simulink model "model"  (R2014a)
(part 1 of 6)
settings: Solver=VariableStepAuto  StartTime=0.0  StopTime=10.0  RelTol=1e-3
libraries: powerlib x1872
settings Model: Creator=lej  LastModifiedBy=leimhofe
settings DataIOCC: SaveFormat=Dataset
settings OptimizationCC: SimCompilerOptimization=off
settings DebuggingCC: MergeDetectMultiDrivingBlocksExec=error  SolverPrmCheckMsg=none  FrameProcessingCompatibilityMsg=error  AllowSymbolicDim=off
settings HardwareCC: ProdBitPerPointer=64  ProdLargestAtomicFloat=Float  ProdIntDivRoundTo=Zero  ProdEndianess=LittleEndian  ProdWordSize=64  ProdHWDeviceType=Intel->x86-64 (Windows64)
settings RTWCC: RTWCompilerOptimization=off
settings GRTTargetCC: GeneratePreprocessorConditionals=Use local settings
settings ConfigComp: CovMetricSettings=dw  CovHtmlReporting=on  CovSaveCumulativeToWorkspaceVar=on  CovSaveSingleToWorkspaceVar=on  CovExternalEMLEnable=off

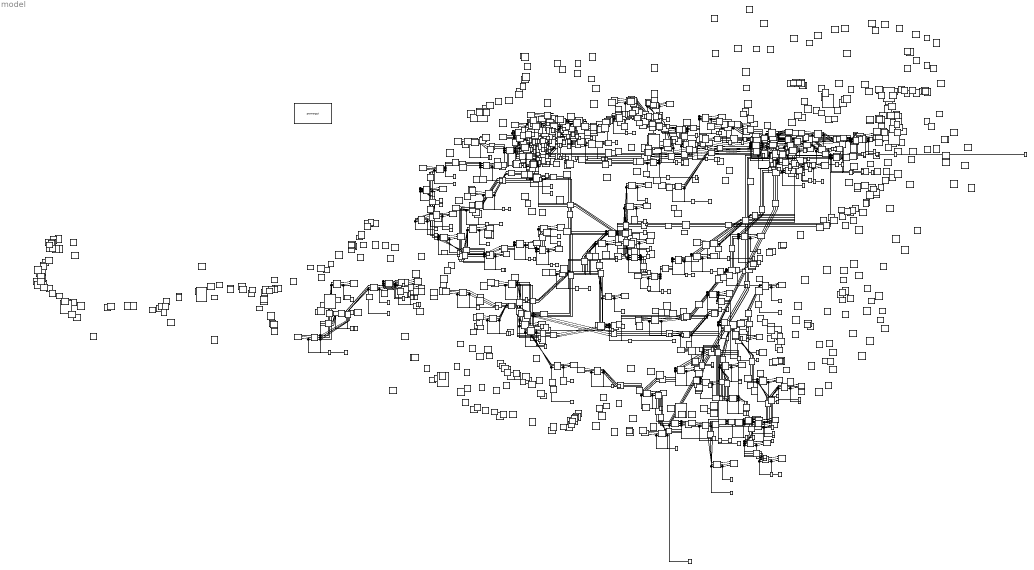
== system model ==
  note: 110000 Volts Power Line
  note: 330000 Volts Power Line
  Aigerding___Antiesenhofen_CN_95975628_110000_CN_95972388_110000 : powerlib/Elements/Distributed Parameters Line  Phases=3  Frequency=60  Resistance=[0.01273 0.3864]  Inductance="[0.9337e-3  4.1264e-3]"  Capacitance=[12.74e-9 7.751e-9]  Length=100  x1=[0 0 0 0; 0.0001244 0 0 0; 0.0002488 0 0 0; 0.0003733 0 0 0; 0.0004977 0 0 0; 0.0006221 0 0 0]  x2=[0 0 0 0; 0.0001244 0 0 0; 0.0002488 0 0 0; 0.0003733 0 0 0; 0.0004977 0 0 0; 0.0006221 0 0 0]  x3=[0 0 0 0; 0.0001244 0 0 0; 0.0002488 0 0 0; 0.0003733 0 0 0; 0.0004977 0 0 0; 0.0006221 0 0 0]  x4=[0 0 0 0; 0.0001244 0 0 0; 0.0002488 0 0 0; 0.0003733 0 0 0; 0.0004977 0 0 0; 0.0006221 0 0 0]  x5=0  V1=ones(3,3)  V2=ones(3,3)  I1=ones(3,3)  I2=ones(3,3)  nHarmo=1  Measurements=None
  Aigerding___Antiesenhofen_CN_95975628_110000_CN_95978048_110000 : powerlib/Elements/Distributed Parameters Line  Phases=3  Frequency=60  Resistance=[0.01273 0.3864]  Inductance="[0.9337e-3  4.1264e-3]"  Capacitance=[12.74e-9 7.751e-9]  Length=100  x1=[0 0 0 0; 0.0001244 0 0 0; 0.0002488 0 0 0; 0.0003733 0 0 0; 0.0004977 0 0 0; 0.0006221 0 0 0]  x2=[0 0 0 0; 0.0001244 0 0 0; 0.0002488 0 0 0; 0.0003733 0 0 0; 0.0004977 0 0 0; 0.0006221 0 0 0]  x3=[0 0 0 0; 0.0001244 0 0 0; 0.0002488 0 0 0; 0.0003733 0 0 0; 0.0004977 0 0 0; 0.0006221 0 0 0]  x4=[0 0 0 0; 0.0001244 0 0 0; 0.0002488 0 0 0; 0.0003733 0 0 0; 0.0004977 0 0 0; 0.0006221 0 0 0]  x5=0  V1=ones(3,3)  V2=ones(3,3)  I1=ones(3,3)  I2=ones(3,3)  nHarmo=1  Measurements=None
  Alutaguse_—_Estonia_Põhja_110_kV_CN_35367472_110000_CN_35594689_110000 : powerlib/Elements/Distributed Parameters Line  Phases=3  Frequency=60  Resistance=[0.01273 0.3864]  Inductance="[0.9337e-3  4.1264e-3]"  Capacitance=[12.74e-9 7.751e-9]  Length=6.3466  x1=[0 0 0 0; 0.0001244 0 0 0; 0.0002488 0 0 0; 0.0003733 0 0 0; 0.0004977 0 0 0; 0.0006221 0 0 0]  x2=[0 0 0 0; 0.0001244 0 0 0; 0.0002488 0 0 0; 0.0003733 0 0 0; 0.0004977 0 0 0; 0.0006221 0 0 0]  x3=[0 0 0 0; 0.0001244 0 0 0; 0.0002488 0 0 0; 0.0003733 0 0 0; 0.0004977 0 0 0; 0.0006221 0 0 0]  x4=[0 0 0 0; 0.0001244 0 0 0; 0.0002488 0 0 0; 0.0003733 0 0 0; 0.0004977 0 0 0; 0.0006221 0 0 0]  x5=0  V1=ones(3,3)  V2=ones(3,3)  I1=ones(3,3)  I2=ones(3,3)  nHarmo=1  Measurements=None
  Alutaguse_—_Konsu_110_kV_CN_35367472_110000_CN_34903294_110000 : powerlib/Elements/Distributed Parameters Line  Phases=3  Frequency=60  Resistance=[0.01273 0.3864]  Inductance="[0.9337e-3  4.1264e-3]"  Capacitance=[12.74e-9 7.751e-9]  Length=14.9855  x1=[0 0 0 0; 0.0001244 0 0 0; 0.0002488 0 0 0; 0.0003733 0 0 0; 0.0004977 0 0 0; 0.0006221 0 0 0]  x2=[0 0 0 0; 0.0001244 0 0 0; 0.0002488 0 0 0; 0.0003733 0 0 0; 0.0004977 0 0 0; 0.0006221 0 0 0]  x3=[0 0 0 0; 0.0001244 0 0 0; 0.0002488 0 0 0; 0.0003733 0 0 0; 0.0004977 0 0 0; 0.0006221 0 0 0]  x4=[0 0 0 0; 0.0001244 0 0 0; 0.0002488 0 0 0; 0.0003733 0 0 0; 0.0004977 0 0 0; 0.0006221 0 0 0]  x5=0  V1=ones(3,3)  V2=ones(3,3)  I1=ones(3,3)  I2=ones(3,3)  nHarmo=1  Measurements=None
  Andau___Frauenkirchen_CN_60222001_110000_CN_174474431_110000 : powerlib/Elements/Distributed Parameters Line  Phases=3  Frequency=60  Resistance=[0.01273 0.3864]  Inductance="[0.9337e-3  4.1264e-3]"  Capacitance=[12.74e-9 7.751e-9]  Length=100  x1=[0 0 0 0; 0.0001244 0 0 0; 0.0002488 0 0 0; 0.0003733 0 0 0; 0.0004977 0 0 0; 0.0006221 0 0 0]  x2=[0 0 0 0; 0.0001244 0 0 0; 0.0002488 0 0 0; 0.0003733 0 0 0; 0.0004977 0 0 0; 0.0006221 0 0 0]  x3=[0 0 0 0; 0.0001244 0 0 0; 0.0002488 0 0 0; 0.0003733 0 0 0; 0.0004977 0 0 0; 0.0006221 0 0 0]  x4=[0 0 0 0; 0.0001244 0 0 0; 0.0002488 0 0 0; 0.0003733 0 0 0; 0.0004977 0 0 0; 0.0006221 0 0 0]  x5=0  V1=ones(3,3)  V2=ones(3,3)  I1=ones(3,3)  I2=ones(3,3)  nHarmo=1  Measurements=None
  Anne_—_Kuuste_110_kV_CN_35445346_110000_CN_30228363_110000 : powerlib/Elements/Distributed Parameters Line  Phases=3  Frequency=60  Resistance=[0.01273 0.3864]  Inductance="[0.9337e-3  4.1264e-3]"  Capacitance=[12.74e-9 7.751e-9]  Length=10.9015  x1=[0 0 0 0; 0.0001244 0 0 0; 0.0002488 0 0 0; 0.0003733 0 0 0; 0.0004977 0 0 0; 0.0006221 0 0 0]  x2=[0 0 0 0; 0.0001244 0 0 0; 0.0002488 0 0 0; 0.0003733 0 0 0; 0.0004977 0 0 0; 0.0006221 0 0 0]  x3=[0 0 0 0; 0.0001244 0 0 0; 0.0002488 0 0 0; 0.0003733 0 0 0; 0.0004977 0 0 0; 0.0006221 0 0 0]  x4=[0 0 0 0; 0.0001244 0 0 0; 0.0002488 0 0 0; 0.0003733 0 0 0; 0.0004977 0 0 0; 0.0006221 0 0 0]  x5=0  V1=ones(3,3)  V2=ones(3,3)  I1=ones(3,3)  I2=ones(3,3)  nHarmo=1  Measurements=None
  Anne_—_Kuuste_110_kV_CN_35445346_110000_CN_35594688_110000 : powerlib/Elements/Distributed Parameters Line  Phases=3  Frequency=60  Resistance=[0.01273 0.3864]  Inductance="[0.9337e-3  4.1264e-3]"  Capacitance=[12.74e-9 7.751e-9]  Length=45.2985  x1=[0 0 0 0; 0.0001244 0 0 0; 0.0002488 0 0 0; 0.0003733 0 0 0; 0.0004977 0 0 0; 0.0006221 0 0 0]  x2=[0 0 0 0; 0.0001244 0 0 0; 0.0002488 0 0 0; 0.0003733 0 0 0; 0.0004977 0 0 0; 0.0006221 0 0 0]  x3=[0 0 0 0; 0.0001244 0 0 0; 0.0002488 0 0 0; 0.0003733 0 0 0; 0.0004977 0 0 0; 0.0006221 0 0 0]  x4=[0 0 0 0; 0.0001244 0 0 0; 0.0002488 0 0 0; 0.0003733 0 0 0; 0.0004977 0 0 0; 0.0006221 0 0 0]  x5=0  V1=ones(3,3)  V2=ones(3,3)  I1=ones(3,3)  I2=ones(3,3)  nHarmo=1  Measurements=None
  Aruküla_—_Jüri_110_kV_CN_34968285_110000_CN_204914596_110000 : powerlib/Elements/Distributed Parameters Line  Phases=3  Frequency=60  Resistance=[0.01273 0.3864]  Inductance="[0.9337e-3  4.1264e-3]"  Capacitance=[12.74e-9 7.751e-9]  Length=9.3434  x1=[0 0 0 0; 0.0001244 0 0 0; 0.0002488 0 0 0; 0.0003733 0 0 0; 0.0004977 0 0 0; 0.0006221 0 0 0]  x2=[0 0 0 0; 0.0001244 0 0 0; 0.0002488 0 0 0; 0.0003733 0 0 0; 0.0004977 0 0 0; 0.0006221 0 0 0]  x3=[0 0 0 0; 0.0001244 0 0 0; 0.0002488 0 0 0; 0.0003733 0 0 0; 0.0004977 0 0 0; 0.0006221 0 0 0]  x4=[0 0 0 0; 0.0001244 0 0 0; 0.0002488 0 0 0; 0.0003733 0 0 0; 0.0004977 0 0 0; 0.0006221 0 0 0]  x5=0  V1=ones(3,3)  V2=ones(3,3)  I1=ones(3,3)  I2=ones(3,3)  nHarmo=1  Measurements=None
  Aruküla_—_Kallavere_110_kV_CN_204914596_110000_CN_29979106_110000 : powerlib/Elements/Distributed Parameters Line  Phases=3  Frequency=60  Resistance=[0.01273 0.3864]  Inductance="[0.9337e-3  4.1264e-3]"  Capacitance=[12.74e-9 7.751e-9]  Length=24.2792  x1=[0 0 0 0; 0.0001244 0 0 0; 0.0002488 0 0 0; 0.0003733 0 0 0; 0.0004977 0 0 0; 0.0006221 0 0 0]  x2=[0 0 0 0; 0.0001244 0 0 0; 0.0002488 0 0 0; 0.0003733 0 0 0; 0.0004977 0 0 0; 0.0006221 0 0 0]  x3=[0 0 0 0; 0.0001244 0 0 0; 0.0002488 0 0 0; 0.0003733 0 0 0; 0.0004977 0 0 0; 0.0006221 0 0 0]  x4=[0 0 0 0; 0.0001244 0 0 0; 0.0002488 0 0 0; 0.0003733 0 0 0; 0.0004977 0 0 0; 0.0006221 0 0 0]  x5=0  V1=ones(3,3)  V2=ones(3,3)  I1=ones(3,3)  I2=ones(3,3)  nHarmo=1  Measurements=None
  Aruküla_—_Kehra_110_kV_CN_35379726_110000_CN_204914596_110000 : powerlib/Elements/Distributed Parameters Line  Phases=3  Frequency=60  Resistance=[0.01273 0.3864]  Inductance="[0.9337e-3  4.1264e-3]"  Capacitance=[12.74e-9 7.751e-9]  Length=19.2682  x1=[0 0 0 0; 0.0001244 0 0 0; 0.0002488 0 0 0; 0.0003733 0 0 0; 0.0004977 0 0 0; 0.0006221 0 0 0]  x2=[0 0 0 0; 0.0001244 0 0 0; 0.0002488 0 0 0; 0.0003733 0 0 0; 0.0004977 0 0 0; 0.0006221 0 0 0]  x3=[0 0 0 0; 0.0001244 0 0 0; 0.0002488 0 0 0; 0.0003733 0 0 0; 0.0004977 0 0 0; 0.0006221 0 0 0]  x4=[0 0 0 0; 0.0001244 0 0 0; 0.0002488 0 0 0; 0.0003733 0 0 0; 0.0004977 0 0 0; 0.0006221 0 0 0]  x5=0  V1=ones(3,3)  V2=ones(3,3)  I1=ones(3,3)  I2=ones(3,3)  nHarmo=1  Measurements=None
  Aruküla_—_Kehra_110_kV_CN_35379726_110000_CN_35384064_110000 : powerlib/Elements/Distributed Parameters Line  Phases=3  Frequency=60  Resistance=[0.01273 0.3864]  Inductance="[0.9337e-3  4.1264e-3]"  Capacitance=[12.74e-9 7.751e-9]  Length=17.352  x1=[0 0 0 0; 0.0001244 0 0 0; 0.0002488 0 0 0; 0.0003733 0 0 0; 0.0004977 0 0 0; 0.0006221 0 0 0]  x2=[0 0 0 0; 0.0001244 0 0 0; 0.0002488 0 0 0; 0.0003733 0 0 0; 0.0004977 0 0 0; 0.0006221 0 0 0]  x3=[0 0 0 0; 0.0001244 0 0 0; 0.0002488 0 0 0; 0.0003733 0 0 0; 0.0004977 0 0 0; 0.0006221 0 0 0]  x4=[0 0 0 0; 0.0001244 0 0 0; 0.0002488 0 0 0; 0.0003733 0 0 0; 0.0004977 0 0 0; 0.0006221 0 0 0]  x5=0  V1=ones(3,3)  V2=ones(3,3)  I1=ones(3,3)  I2=ones(3,3)  nHarmo=1  Measurements=None
  Attnang_Puchheim_–_Steindorf_CN_33685690_110000_CN_32493406_110000 : powerlib/Elements/Distributed Parameters Line  Phases=3  Frequency=60  Resistance=[0.01273 0.3864]  Inductance="[0.9337e-3  4.1264e-3]"  Capacitance=[12.74e-9 7.751e-9]  Length=100  x1=[0 0 0 0; 0.0001244 0 0 0; 0.0002488 0 0 0; 0.0003733 0 0 0; 0.0004977 0 0 0; 0.0006221 0 0 0]  x2=[0 0 0 0; 0.0001244 0 0 0; 0.0002488 0 0 0; 0.0003733 0 0 0; 0.0004977 0 0 0; 0.0006221 0 0 0]  x3=[0 0 0 0; 0.0001244 0 0 0; 0.0002488 0 0 0; 0.0003733 0 0 0; 0.0004977 0 0 0; 0.0006221 0 0 0]  x4=[0 0 0 0; 0.0001244 0 0 0; 0.0002488 0 0 0; 0.0003733 0 0 0; 0.0004977 0 0 0; 0.0006221 0 0 0]  x5=0  V1=ones(3,3)  V2=ones(3,3)  I1=ones(3,3)  I2=ones(3,3)  nHarmo=1  Measurements=None
  Aulepa_—_Taebla_110_kV_CN_101177924_110000_CN_34988525_110000 : powerlib/Elements/Distributed Parameters Line  Phases=3  Frequency=60  Resistance=[0.01273 0.3864]  Inductance="[0.9337e-3  4.1264e-3]"  Capacitance=[12.74e-9 7.751e-9]  Length=41.8737  x1=[0 0 0 0; 0.0001244 0 0 0; 0.0002488 0 0 0; 0.0003733 0 0 0; 0.0004977 0 0 0; 0.0006221 0 0 0]  x2=[0 0 0 0; 0.0001244 0 0 0; 0.0002488 0 0 0; 0.0003733 0 0 0; 0.0004977 0 0 0; 0.0006221 0 0 0]  x3=[0 0 0 0; 0.0001244 0 0 0; 0.0002488 0 0 0; 0.0003733 0 0 0; 0.0004977 0 0 0; 0.0006221 0 0 0]  x4=[0 0 0 0; 0.0001244 0 0 0; 0.0002488 0 0 0; 0.0003733 0 0 0; 0.0004977 0 0 0; 0.0006221 0 0 0]  x5=0  V1=ones(3,3)  V2=ones(3,3)  I1=ones(3,3)  I2=ones(3,3)  nHarmo=1  Measurements=None
  Aulepa_—_Taebla_110_kV_CN_101177924_110000_CN_34988527_110000 : powerlib/Elements/Distributed Parameters Line  Phases=3  Frequency=60  Resistance=[0.01273 0.3864]  Inductance="[0.9337e-3  4.1264e-3]"  Capacitance=[12.74e-9 7.751e-9]  Length=28.206  x1=[0 0 0 0; 0.0001244 0 0 0; 0.0002488 0 0 0; 0.0003733 0 0 0; 0.0004977 0 0 0; 0.0006221 0 0 0]  x2=[0 0 0 0; 0.0001244 0 0 0; 0.0002488 0 0 0; 0.0003733 0 0 0; 0.0004977 0 0 0; 0.0006221 0 0 0]  x3=[0 0 0 0; 0.0001244 0 0 0; 0.0002488 0 0 0; 0.0003733 0 0 0; 0.0004977 0 0 0; 0.0006221 0 0 0]  x4=[0 0 0 0; 0.0001244 0 0 0; 0.0002488 0 0 0; 0.0003733 0 0 0; 0.0004977 0 0 0; 0.0006221 0 0 0]  x5=0  V1=ones(3,3)  V2=ones(3,3)  I1=ones(3,3)  I2=ones(3,3)  nHarmo=1  Measurements=None
  Aulepa_—_Taebla_110_kV_CN_101177924_110000_CN_34988531_110000 : powerlib/Elements/Distributed Parameters Line  Phases=3  Frequency=60  Resistance=[0.01273 0.3864]  Inductance="[0.9337e-3  4.1264e-3]"  Capacitance=[12.74e-9 7.751e-9]  Length=17.3473  x1=[0 0 0 0; 0.0001244 0 0 0; 0.0002488 0 0 0; 0.0003733 0 0 0; 0.0004977 0 0 0; 0.0006221 0 0 0]  x2=[0 0 0 0; 0.0001244 0 0 0; 0.0002488 0 0 0; 0.0003733 0 0 0; 0.0004977 0 0 0; 0.0006221 0 0 0]  x3=[0 0 0 0; 0.0001244 0 0 0; 0.0002488 0 0 0; 0.0003733 0 0 0; 0.0004977 0 0 0; 0.0006221 0 0 0]  x4=[0 0 0 0; 0.0001244 0 0 0; 0.0002488 0 0 0; 0.0003733 0 0 0; 0.0004977 0 0 0; 0.0006221 0 0 0]  x5=0  V1=ones(3,3)  V2=ones(3,3)  I1=ones(3,3)  I2=ones(3,3)  nHarmo=1  Measurements=None
  Bad_Hall___Steyr_Nord;Kremsmünster___Bad_Hall_CN_95025698_110000_CN_33066376_110000 : powerlib/Elements/Distributed Parameters Line  Phases=3  Frequency=60  Resistance=[0.01273 0.3864]  Inductance="[0.9337e-3  4.1264e-3]"  Capacitance=[12.74e-9 7.751e-9]  Length=100  x1=[0 0 0 0; 0.0001244 0 0 0; 0.0002488 0 0 0; 0.0003733 0 0 0; 0.0004977 0 0 0; 0.0006221 0 0 0]  x2=[0 0 0 0; 0.0001244 0 0 0; 0.0002488 0 0 0; 0.0003733 0 0 0; 0.0004977 0 0 0; 0.0006221 0 0 0]  x3=[0 0 0 0; 0.0001244 0 0 0; 0.0002488 0 0 0; 0.0003733 0 0 0; 0.0004977 0 0 0; 0.0006221 0 0 0]  x4=[0 0 0 0; 0.0001244 0 0 0; 0.0002488 0 0 0; 0.0003733 0 0 0; 0.0004977 0 0 0; 0.0006221 0 0 0]  x5=0  V1=ones(3,3)  V2=ones(3,3)  I1=ones(3,3)  I2=ones(3,3)  nHarmo=1  Measurements=None
  Bad_Hall___Steyr_Nord;Kremsmünster___Bad_Hall_CN_95025698_110000_CN_50899766_110000 : powerlib/Elements/Distributed Parameters Line  Phases=3  Frequency=60  Resistance=[0.01273 0.3864]  Inductance="[0.9337e-3  4.1264e-3]"  Capacitance=[12.74e-9 7.751e-9]  Length=100  x1=[0 0 0 0; 0.0001244 0 0 0; 0.0002488 0 0 0; 0.0003733 0 0 0; 0.0004977 0 0 0; 0.0006221 0 0 0]  x2=[0 0 0 0; 0.0001244 0 0 0; 0.0002488 0 0 0; 0.0003733 0 0 0; 0.0004977 0 0 0; 0.0006221 0 0 0]  x3=[0 0 0 0; 0.0001244 0 0 0; 0.0002488 0 0 0; 0.0003733 0 0 0; 0.0004977 0 0 0; 0.0006221 0 0 0]  x4=[0 0 0 0; 0.0001244 0 0 0; 0.0002488 0 0 0; 0.0003733 0 0 0; 0.0004977 0 0 0; 0.0006221 0 0 0]  x5=0  V1=ones(3,3)  V2=ones(3,3)  I1=ones(3,3)  I2=ones(3,3)  nHarmo=1  Measurements=None
  Balti_EJ_—_Allika_110_kV_CN_35367481_110000_CN_34682059_110000 : powerlib/Elements/Distributed Parameters Line  Phases=3  Frequency=60  Resistance=[0.01273 0.3864]  Inductance="[0.9337e-3  4.1264e-3]"  Capacitance=[12.74e-9 7.751e-9]  Length=28.5895  x1=[0 0 0 0; 0.0001244 0 0 0; 0.0002488 0 0 0; 0.0003733 0 0 0; 0.0004977 0 0 0; 0.0006221 0 0 0]  x2=[0 0 0 0; 0.0001244 0 0 0; 0.0002488 0 0 0; 0.0003733 0 0 0; 0.0004977 0 0 0; 0.0006221 0 0 0]  x3=[0 0 0 0; 0.0001244 0 0 0; 0.0002488 0 0 0; 0.0003733 0 0 0; 0.0004977 0 0 0; 0.0006221 0 0 0]  x4=[0 0 0 0; 0.0001244 0 0 0; 0.0002488 0 0 0; 0.0003733 0 0 0; 0.0004977 0 0 0; 0.0006221 0 0 0]  x5=0  V1=ones(3,3)  V2=ones(3,3)  I1=ones(3,3)  I2=ones(3,3)  nHarmo=1  Measurements=None
  Balti_EJ_—_Narva_HEJ_110_kV_CN_34682059_110000_CN_321829090_110000 : powerlib/Elements/Distributed Parameters Line  Phases=3  Frequency=60  Resistance=[0.01273 0.3864]  Inductance="[0.9337e-3  4.1264e-3]"  Capacitance=[12.74e-9 7.751e-9]  Length=4.3361  x1=[0 0 0 0; 0.0001244 0 0 0; 0.0002488 0 0 0; 0.0003733 0 0 0; 0.0004977 0 0 0; 0.0006221 0 0 0]  x2=[0 0 0 0; 0.0001244 0 0 0; 0.0002488 0 0 0; 0.0003733 0 0 0; 0.0004977 0 0 0; 0.0006221 0 0 0]  x3=[0 0 0 0; 0.0001244 0 0 0; 0.0002488 0 0 0; 0.0003733 0 0 0; 0.0004977 0 0 0; 0.0006221 0 0 0]  x4=[0 0 0 0; 0.0001244 0 0 0; 0.0002488 0 0 0; 0.0003733 0 0 0; 0.0004977 0 0 0; 0.0006221 0 0 0]  x5=0  V1=ones(3,3)  V2=ones(3,3)  I1=ones(3,3)  I2=ones(3,3)  nHarmo=1  Measurements=None
  Balti_EJ_—_PTK_110_kV_CN_264287766_110000_CN_139400061_110000 : powerlib/Elements/Distributed Parameters Line  Phases=3  Frequency=60  Resistance=[0.01273 0.3864]  Inductance="[0.9337e-3  4.1264e-3]"  Capacitance=[12.74e-9 7.751e-9]  Length=50.4258  x1=[0 0 0 0; 0.0001244 0 0 0; 0.0002488 0 0 0; 0.0003733 0 0 0; 0.0004977 0 0 0; 0.0006221 0 0 0]  x2=[0 0 0 0; 0.0001244 0 0 0; 0.0002488 0 0 0; 0.0003733 0 0 0; 0.0004977 0 0 0; 0.0006221 0 0 0]  x3=[0 0 0 0; 0.0001244 0 0 0; 0.0002488 0 0 0; 0.0003733 0 0 0; 0.0004977 0 0 0; 0.0006221 0 0 0]  x4=[0 0 0 0; 0.0001244 0 0 0; 0.0002488 0 0 0; 0.0003733 0 0 0; 0.0004977 0 0 0; 0.0006221 0 0 0]  x5=0  V1=ones(3,3)  V2=ones(3,3)  I1=ones(3,3)  I2=ones(3,3)  nHarmo=1  Measurements=None
  Balti_EJ_—_PTK_110_kV_CN_264287766_110000_CN_205980356_110000 : powerlib/Elements/Distributed Parameters Line  Phases=3  Frequency=60  Resistance=[0.01273 0.3864]  Inductance="[0.9337e-3  4.1264e-3]"  Capacitance=[12.74e-9 7.751e-9]  Length=25.9983  x1=[0 0 0 0; 0.0001244 0 0 0; 0.0002488 0 0 0; 0.0003733 0 0 0; 0.0004977 0 0 0; 0.0006221 0 0 0]  x2=[0 0 0 0; 0.0001244 0 0 0; 0.0002488 0 0 0; 0.0003733 0 0 0; 0.0004977 0 0 0; 0.0006221 0 0 0]  x3=[0 0 0 0; 0.0001244 0 0 0; 0.0002488 0 0 0; 0.0003733 0 0 0; 0.0004977 0 0 0; 0.0006221 0 0 0]  x4=[0 0 0 0; 0.0001244 0 0 0; 0.0002488 0 0 0; 0.0003733 0 0 0; 0.0004977 0 0 0; 0.0006221 0 0 0]  x5=0  V1=ones(3,3)  V2=ones(3,3)  I1=ones(3,3)  I2=ones(3,3)  nHarmo=1  Measurements=None
  Balti_EJ_—_PTK_110_kV_CN_264287766_110000_CN_34682059_110000 : powerlib/Elements/Distributed Parameters Line  Phases=3  Frequency=60  Resistance=[0.01273 0.3864]  Inductance="[0.9337e-3  4.1264e-3]"  Capacitance=[12.74e-9 7.751e-9]  Length=53.3424  x1=[0 0 0 0; 0.0001244 0 0 0; 0.0002488 0 0 0; 0.0003733 0 0 0; 0.0004977 0 0 0; 0.0006221 0 0 0]  x2=[0 0 0 0; 0.0001244 0 0 0; 0.0002488 0 0 0; 0.0003733 0 0 0; 0.0004977 0 0 0; 0.0006221 0 0 0]  x3=[0 0 0 0; 0.0001244 0 0 0; 0.0002488 0 0 0; 0.0003733 0 0 0; 0.0004977 0 0 0; 0.0006221 0 0 0]  x4=[0 0 0 0; 0.0001244 0 0 0; 0.0002488 0 0 0; 0.0003733 0 0 0; 0.0004977 0 0 0; 0.0006221 0 0 0]  x5=0  V1=ones(3,3)  V2=ones(3,3)  I1=ones(3,3)  I2=ones(3,3)  nHarmo=1  Measurements=None
  Balti_EJ_—_PTK_110_kV_CN_264287766_110000_CN_35367480_110000 : powerlib/Elements/Distributed Parameters Line  Phases=3  Frequency=60  Resistance=[0.01273 0.3864]  Inductance="[0.9337e-3  4.1264e-3]"  Capacitance=[12.74e-9 7.751e-9]  Length=36.831  x1=[0 0 0 0; 0.0001244 0 0 0; 0.0002488 0 0 0; 0.0003733 0 0 0; 0.0004977 0 0 0; 0.0006221 0 0 0]  x2=[0 0 0 0; 0.0001244 0 0 0; 0.0002488 0 0 0; 0.0003733 0 0 0; 0.0004977 0 0 0; 0.0006221 0 0 0]  x3=[0 0 0 0; 0.0001244 0 0 0; 0.0002488 0 0 0; 0.0003733 0 0 0; 0.0004977 0 0 0; 0.0006221 0 0 0]  x4=[0 0 0 0; 0.0001244 0 0 0; 0.0002488 0 0 0; 0.0003733 0 0 0; 0.0004977 0 0 0; 0.0006221 0 0 0]  x5=0  V1=ones(3,3)  V2=ones(3,3)  I1=ones(3,3)  I2=ones(3,3)  nHarmo=1  Measurements=None
  Balti_EJ_—_PTK_110_kV_CN_264287766_110000_CN_35594697_110000 : powerlib/Elements/Distributed Parameters Line  Phases=3  Frequency=60  Resistance=[0.01273 0.3864]  Inductance="[0.9337e-3  4.1264e-3]"  Capacitance=[12.74e-9 7.751e-9]  Length=24.8341  x1=[0 0 0 0; 0.0001244 0 0 0; 0.0002488 0 0 0; 0.0003733 0 0 0; 0.0004977 0 0 0; 0.0006221 0 0 0]  x2=[0 0 0 0; 0.0001244 0 0 0; 0.0002488 0 0 0; 0.0003733 0 0 0; 0.0004977 0 0 0; 0.0006221 0 0 0]  x3=[0 0 0 0; 0.0001244 0 0 0; 0.0002488 0 0 0; 0.0003733 0 0 0; 0.0004977 0 0 0; 0.0006221 0 0 0]  x4=[0 0 0 0; 0.0001244 0 0 0; 0.0002488 0 0 0; 0.0003733 0 0 0; 0.0004977 0 0 0; 0.0006221 0 0 0]  x5=0  V1=ones(3,3)  V2=ones(3,3)  I1=ones(3,3)  I2=ones(3,3)  nHarmo=1  Measurements=None
  Balti_EJ_—_Püssi_330_kV_CN_34920675_330000_CN_34682059_330000 : powerlib/Elements/Distributed Parameters Line  Phases=3  Frequency=60  Resistance=[0.01273 0.3864]  Inductance="[0.9337e-3  4.1264e-3]"  Capacitance=[12.74e-9 7.751e-9]  Length=51.056  x1=[0 0 0 0; 0.0001244 0 0 0; 0.0002488 0 0 0; 0.0003733 0 0 0; 0.0004977 0 0 0; 0.0006221 0 0 0]  x2=[0 0 0 0; 0.0001244 0 0 0; 0.0002488 0 0 0; 0.0003733 0 0 0; 0.0004977 0 0 0; 0.0006221 0 0 0]  x3=[0 0 0 0; 0.0001244 0 0 0; 0.0002488 0 0 0; 0.0003733 0 0 0; 0.0004977 0 0 0; 0.0006221 0 0 0]  x4=[0 0 0 0; 0.0001244 0 0 0; 0.0002488 0 0 0; 0.0003733 0 0 0; 0.0004977 0 0 0; 0.0006221 0 0 0]  x5=0  V1=ones(3,3)  V2=ones(3,3)  I1=ones(3,3)  I2=ones(3,3)  nHarmo=1  Measurements=None
  Balti_—_Tartu_330_kV_&_Tartu_—_Viljandi_330_kV_CN_34682089_330000_CN_34682059_330000 : powerlib/Elements/Distributed Parameters Line  Phases=3  Frequency=60  Resistance=[0.01273 0.3864]  Inductance="[0.9337e-3  4.1264e-3]"  Capacitance=[12.74e-9 7.751e-9]  Length=51.4732  x1=[0 0 0 0; 0.0001244 0 0 0; 0.0002488 0 0 0; 0.0003733 0 0 0; 0.0004977 0 0 0; 0.0006221 0 0 0]  x2=[0 0 0 0; 0.0001244 0 0 0; 0.0002488 0 0 0; 0.0003733 0 0 0; 0.0004977 0 0 0; 0.0006221 0 0 0]  x3=[0 0 0 0; 0.0001244 0 0 0; 0.0002488 0 0 0; 0.0003733 0 0 0; 0.0004977 0 0 0; 0.0006221 0 0 0]  x4=[0 0 0 0; 0.0001244 0 0 0; 0.0002488 0 0 0; 0.0003733 0 0 0; 0.0004977 0 0 0; 0.0006221 0 0 0]  x5=0  V1=ones(3,3)  V2=ones(3,3)  I1=ones(3,3)  I2=ones(3,3)  nHarmo=1  Measurements=None
  Balti_—_Tartu_330_kV_&_Tartu_—_Viljandi_330_kV_CN_34682089_330000_CN_35450930_330000 : powerlib/Elements/Distributed Parameters Line  Phases=3  Frequency=60  Resistance=[0.01273 0.3864]  Inductance="[0.9337e-3  4.1264e-3]"  Capacitance=[12.74e-9 7.751e-9]  Length=162.6337  x1=[0 0 0 0; 0.0001244 0 0 0; 0.0002488 0 0 0; 0.0003733 0 0 0; 0.0004977 0 0 0; 0.0006221 0 0 0]  x2=[0 0 0 0; 0.0001244 0 0 0; 0.0002488 0 0 0; 0.0003733 0 0 0; 0.0004977 0 0 0; 0.0006221 0 0 0]  x3=[0 0 0 0; 0.0001244 0 0 0; 0.0002488 0 0 0; 0.0003733 0 0 0; 0.0004977 0 0 0; 0.0006221 0 0 0]  x4=[0 0 0 0; 0.0001244 0 0 0; 0.0002488 0 0 0; 0.0003733 0 0 0; 0.0004977 0 0 0; 0.0006221 0 0 0]  x5=0  V1=ones(3,3)  V2=ones(3,3)  I1=ones(3,3)  I2=ones(3,3)  nHarmo=1  Measurements=None
  Bisamberg___Mistelbach_CN_28504203_110000_CN_128734659_110000 : powerlib/Elements/Distributed Parameters Line  Phases=3  Frequency=60  Resistance=[0.01273 0.3864]  Inductance="[0.9337e-3  4.1264e-3]"  Capacitance=[12.74e-9 7.751e-9]  Length=100  x1=[0 0 0 0; 0.0001244 0 0 0; 0.0002488 0 0 0; 0.0003733 0 0 0; 0.0004977 0 0 0; 0.0006221 0 0 0]  x2=[0 0 0 0; 0.0001244 0 0 0; 0.0002488 0 0 0; 0.0003733 0 0 0; 0.0004977 0 0 0; 0.0006221 0 0 0]  x3=[0 0 0 0; 0.0001244 0 0 0; 0.0002488 0 0 0; 0.0003733 0 0 0; 0.0004977 0 0 0; 0.0006221 0 0 0]  x4=[0 0 0 0; 0.0001244 0 0 0; 0.0002488 0 0 0; 0.0003733 0 0 0; 0.0004977 0 0 0; 0.0006221 0 0 0]  x5=0  V1=ones(3,3)  V2=ones(3,3)  I1=ones(3,3)  I2=ones(3,3)  nHarmo=1  Measurements=None
  Bisamberg___Mistelbach_CN_28504203_110000_CN_96616299_110000 : powerlib/Elements/Distributed Parameters Line  Phases=3  Frequency=60  Resistance=[0.01273 0.3864]  Inductance="[0.9337e-3  4.1264e-3]"  Capacitance=[12.74e-9 7.751e-9]  Length=100  x1=[0 0 0 0; 0.0001244 0 0 0; 0.0002488 0 0 0; 0.0003733 0 0 0; 0.0004977 0 0 0; 0.0006221 0 0 0]  x2=[0 0 0 0; 0.0001244 0 0 0; 0.0002488 0 0 0; 0.0003733 0 0 0; 0.0004977 0 0 0; 0.0006221 0 0 0]  x3=[0 0 0 0; 0.0001244 0 0 0; 0.0002488 0 0 0; 0.0003733 0 0 0; 0.0004977 0 0 0; 0.0006221 0 0 0]  x4=[0 0 0 0; 0.0001244 0 0 0; 0.0002488 0 0 0; 0.0003733 0 0 0; 0.0004977 0 0 0; 0.0006221 0 0 0]  x5=0  V1=ones(3,3)  V2=ones(3,3)  I1=ones(3,3)  I2=ones(3,3)  nHarmo=1  Measurements=None
  Bockfließ___Gänserndorf_CN_96346322_110000_CN_123444716_110000 : powerlib/Elements/Distributed Parameters Line  Phases=3  Frequency=60  Resistance=[0.01273 0.3864]  Inductance="[0.9337e-3  4.1264e-3]"  Capacitance=[12.74e-9 7.751e-9]  Length=100  x1=[0 0 0 0; 0.0001244 0 0 0; 0.0002488 0 0 0; 0.0003733 0 0 0; 0.0004977 0 0 0; 0.0006221 0 0 0]  x2=[0 0 0 0; 0.0001244 0 0 0; 0.0002488 0 0 0; 0.0003733 0 0 0; 0.0004977 0 0 0; 0.0006221 0 0 0]  x3=[0 0 0 0; 0.0001244 0 0 0; 0.0002488 0 0 0; 0.0003733 0 0 0; 0.0004977 0 0 0; 0.0006221 0 0 0]  x4=[0 0 0 0; 0.0001244 0 0 0; 0.0002488 0 0 0; 0.0003733 0 0 0; 0.0004977 0 0 0; 0.0006221 0 0 0]  x5=0  V1=ones(3,3)  V2=ones(3,3)  I1=ones(3,3)  I2=ones(3,3)  nHarmo=1  Measurements=None
  Braz_–_Bludenz_CN_126218483_110000_CN_101976746_110000 : powerlib/Elements/Distributed Parameters Line  Phases=3  Frequency=60  Resistance=[0.01273 0.3864]  Inductance="[0.9337e-3  4.1264e-3]"  Capacitance=[12.74e-9 7.751e-9]  Length=100  x1=[0 0 0 0; 0.0001244 0 0 0; 0.0002488 0 0 0; 0.0003733 0 0 0; 0.0004977 0 0 0; 0.0006221 0 0 0]  x2=[0 0 0 0; 0.0001244 0 0 0; 0.0002488 0 0 0; 0.0003733 0 0 0; 0.0004977 0 0 0; 0.0006221 0 0 0]  x3=[0 0 0 0; 0.0001244 0 0 0; 0.0002488 0 0 0; 0.0003733 0 0 0; 0.0004977 0 0 0; 0.0006221 0 0 0]  x4=[0 0 0 0; 0.0001244 0 0 0; 0.0002488 0 0 0; 0.0003733 0 0 0; 0.0004977 0 0 0; 0.0006221 0 0 0]  x5=0  V1=ones(3,3)  V2=ones(3,3)  I1=ones(3,3)  I2=ones(3,3)  nHarmo=1  Measurements=None
  Braz_–_Bludenz_CN_126218483_110000_CN_32821660_110000 : powerlib/Elements/Distributed Parameters Line  Phases=3  Frequency=60  Resistance=[0.01273 0.3864]  Inductance="[0.9337e-3  4.1264e-3]"  Capacitance=[12.74e-9 7.751e-9]  Length=100  x1=[0 0 0 0; 0.0001244 0 0 0; 0.0002488 0 0 0; 0.0003733 0 0 0; 0.0004977 0 0 0; 0.0006221 0 0 0]  x2=[0 0 0 0; 0.0001244 0 0 0; 0.0002488 0 0 0; 0.0003733 0 0 0; 0.0004977 0 0 0; 0.0006221 0 0 0]  x3=[0 0 0 0; 0.0001244 0 0 0; 0.0002488 0 0 0; 0.0003733 0 0 0; 0.0004977 0 0 0; 0.0006221 0 0 0]  x4=[0 0 0 0; 0.0001244 0 0 0; 0.0002488 0 0 0; 0.0003733 0 0 0; 0.0004977 0 0 0; 0.0006221 0 0 0]  x5=0  V1=ones(3,3)  V2=ones(3,3)  I1=ones(3,3)  I2=ones(3,3)  nHarmo=1  Measurements=None
  Bruck_Mur___Hieflau_CN_81611149_110000_CN_96763013_110000 : powerlib/Elements/Distributed Parameters Line  Phases=3  Frequency=60  Resistance=[0.01273 0.3864]  Inductance="[0.9337e-3  4.1264e-3]"  Capacitance=[12.74e-9 7.751e-9]  Length=100  x1=[0 0 0 0; 0.0001244 0 0 0; 0.0002488 0 0 0; 0.0003733 0 0 0; 0.0004977 0 0 0; 0.0006221 0 0 0]  x2=[0 0 0 0; 0.0001244 0 0 0; 0.0002488 0 0 0; 0.0003733 0 0 0; 0.0004977 0 0 0; 0.0006221 0 0 0]  x3=[0 0 0 0; 0.0001244 0 0 0; 0.0002488 0 0 0; 0.0003733 0 0 0; 0.0004977 0 0 0; 0.0006221 0 0 0]  x4=[0 0 0 0; 0.0001244 0 0 0; 0.0002488 0 0 0; 0.0003733 0 0 0; 0.0004977 0 0 0; 0.0006221 0 0 0]  x5=0  V1=ones(3,3)  V2=ones(3,3)  I1=ones(3,3)  I2=ones(3,3)  nHarmo=1  Measurements=None
  Böckstein___Angertal_CN_88844735_110000_CN_86331083_110000 : powerlib/Elements/Distributed Parameters Line  Phases=3  Frequency=60  Resistance=[0.01273 0.3864]  Inductance="[0.9337e-3  4.1264e-3]"  Capacitance=[12.74e-9 7.751e-9]  Length=100  x1=[0 0 0 0; 0.0001244 0 0 0; 0.0002488 0 0 0; 0.0003733 0 0 0; 0.0004977 0 0 0; 0.0006221 0 0 0]  x2=[0 0 0 0; 0.0001244 0 0 0; 0.0002488 0 0 0; 0.0003733 0 0 0; 0.0004977 0 0 0; 0.0006221 0 0 0]  x3=[0 0 0 0; 0.0001244 0 0 0; 0.0002488 0 0 0; 0.0003733 0 0 0; 0.0004977 0 0 0; 0.0006221 0 0 0]  x4=[0 0 0 0; 0.0001244 0 0 0; 0.0002488 0 0 0; 0.0003733 0 0 0; 0.0004977 0 0 0; 0.0006221 0 0 0]  x5=0  V1=ones(3,3)  V2=ones(3,3)  I1=ones(3,3)  I2=ones(3,3)  nHarmo=1  Measurements=None
  Böckstein___Angertal_CN_88844735_110000_CN_86331084_110000 : powerlib/Elements/Distributed Parameters Line  Phases=3  Frequency=60  Resistance=[0.01273 0.3864]  Inductance="[0.9337e-3  4.1264e-3]"  Capacitance=[12.74e-9 7.751e-9]  Length=100  x1=[0 0 0 0; 0.0001244 0 0 0; 0.0002488 0 0 0; 0.0003733 0 0 0; 0.0004977 0 0 0; 0.0006221 0 0 0]  x2=[0 0 0 0; 0.0001244 0 0 0; 0.0002488 0 0 0; 0.0003733 0 0 0; 0.0004977 0 0 0; 0.0006221 0 0 0]  x3=[0 0 0 0; 0.0001244 0 0 0; 0.0002488 0 0 0; 0.0003733 0 0 0; 0.0004977 0 0 0; 0.0006221 0 0 0]  x4=[0 0 0 0; 0.0001244 0 0 0; 0.0002488 0 0 0; 0.0003733 0 0 0; 0.0004977 0 0 0; 0.0006221 0 0 0]  x5=0  V1=ones(3,3)  V2=ones(3,3)  I1=ones(3,3)  I2=ones(3,3)  nHarmo=1  Measurements=None
  Bösdornau___Zell_CN_156973414_110000_CN_99858973_110000 : powerlib/Elements/Distributed Parameters Line  Phases=3  Frequency=60  Resistance=[0.01273 0.3864]  Inductance="[0.9337e-3  4.1264e-3]"  Capacitance=[12.74e-9 7.751e-9]  Length=100  x1=[0 0 0 0; 0.0001244 0 0 0; 0.0002488 0 0 0; 0.0003733 0 0 0; 0.0004977 0 0 0; 0.0006221 0 0 0]  x2=[0 0 0 0; 0.0001244 0 0 0; 0.0002488 0 0 0; 0.0003733 0 0 0; 0.0004977 0 0 0; 0.0006221 0 0 0]  x3=[0 0 0 0; 0.0001244 0 0 0; 0.0002488 0 0 0; 0.0003733 0 0 0; 0.0004977 0 0 0; 0.0006221 0 0 0]  x4=[0 0 0 0; 0.0001244 0 0 0; 0.0002488 0 0 0; 0.0003733 0 0 0; 0.0004977 0 0 0; 0.0006221 0 0 0]  x5=0  V1=ones(3,3)  V2=ones(3,3)  I1=ones(3,3)  I2=ones(3,3)  nHarmo=1  Measurements=None
  Deutsch_Altenburg___Gänserndorf_CN_96346322_110000_CN_83643796_110000 : powerlib/Elements/Distributed Parameters Line  Phases=3  Frequency=60  Resistance=[0.01273 0.3864]  Inductance="[0.9337e-3  4.1264e-3]"  Capacitance=[12.74e-9 7.751e-9]  Length=100  x1=[0 0 0 0; 0.0001244 0 0 0; 0.0002488 0 0 0; 0.0003733 0 0 0; 0.0004977 0 0 0; 0.0006221 0 0 0]  x2=[0 0 0 0; 0.0001244 0 0 0; 0.0002488 0 0 0; 0.0003733 0 0 0; 0.0004977 0 0 0; 0.0006221 0 0 0]  x3=[0 0 0 0; 0.0001244 0 0 0; 0.0002488 0 0 0; 0.0003733 0 0 0; 0.0004977 0 0 0; 0.0006221 0 0 0]  x4=[0 0 0 0; 0.0001244 0 0 0; 0.0002488 0 0 0; 0.0003733 0 0 0; 0.0004977 0 0 0; 0.0006221 0 0 0]  x5=0  V1=ones(3,3)  V2=ones(3,3)  I1=ones(3,3)  I2=ones(3,3)  nHarmo=1  Measurements=None
  Deutschlandsberg___Bergla_CN_89555133_110000_CN_87702041_110000 : powerlib/Elements/Distributed Parameters Line  Phases=3  Frequency=60  Resistance=[0.01273 0.3864]  Inductance="[0.9337e-3  4.1264e-3]"  Capacitance=[12.74e-9 7.751e-9]  Length=100  x1=[0 0 0 0; 0.0001244 0 0 0; 0.0002488 0 0 0; 0.0003733 0 0 0; 0.0004977 0 0 0; 0.0006221 0 0 0]  x2=[0 0 0 0; 0.0001244 0 0 0; 0.0002488 0 0 0; 0.0003733 0 0 0; 0.0004977 0 0 0; 0.0006221 0 0 0]  x3=[0 0 0 0; 0.0001244 0 0 0; 0.0002488 0 0 0; 0.0003733 0 0 0; 0.0004977 0 0 0; 0.0006221 0 0 0]  x4=[0 0 0 0; 0.0001244 0 0 0; 0.0002488 0 0 0; 0.0003733 0 0 0; 0.0004977 0 0 0; 0.0006221 0 0 0]  x5=0  V1=ones(3,3)  V2=ones(3,3)  I1=ones(3,3)  I2=ones(3,3)  nHarmo=1  Measurements=None
  Dürnrohr___Tulln_CN_33632720_110000_CN_288347513_110000 : powerlib/Elements/Distributed Parameters Line  Phases=3  Frequency=60  Resistance=[0.01273 0.3864]  Inductance="[0.9337e-3  4.1264e-3]"  Capacitance=[12.74e-9 7.751e-9]  Length=100  x1=[0 0 0 0; 0.0001244 0 0 0; 0.0002488 0 0 0; 0.0003733 0 0 0; 0.0004977 0 0 0; 0.0006221 0 0 0]  x2=[0 0 0 0; 0.0001244 0 0 0; 0.0002488 0 0 0; 0.0003733 0 0 0; 0.0004977 0 0 0; 0.0006221 0 0 0]  x3=[0 0 0 0; 0.0001244 0 0 0; 0.0002488 0 0 0; 0.0003733 0 0 0; 0.0004977 0 0 0; 0.0006221 0 0 0]  x4=[0 0 0 0; 0.0001244 0 0 0; 0.0002488 0 0 0; 0.0003733 0 0 0; 0.0004977 0 0 0; 0.0006221 0 0 0]  x5=0  V1=ones(3,3)  V2=ones(3,3)  I1=ones(3,3)  I2=ones(3,3)  nHarmo=1  Measurements=None
  Dürnrohr___Tulln_CN_33632720_110000_CN_33631764_110000 : powerlib/Elements/Distributed Parameters Line  Phases=3  Frequency=60  Resistance=[0.01273 0.3864]  Inductance="[0.9337e-3  4.1264e-3]"  Capacitance=[12.74e-9 7.751e-9]  Length=100  x1=[0 0 0 0; 0.0001244 0 0 0; 0.0002488 0 0 0; 0.0003733 0 0 0; 0.0004977 0 0 0; 0.0006221 0 0 0]  x2=[0 0 0 0; 0.0001244 0 0 0; 0.0002488 0 0 0; 0.0003733 0 0 0; 0.0004977 0 0 0; 0.0006221 0 0 0]  x3=[0 0 0 0; 0.0001244 0 0 0; 0.0002488 0 0 0; 0.0003733 0 0 0; 0.0004977 0 0 0; 0.0006221 0 0 0]  x4=[0 0 0 0; 0.0001244 0 0 0; 0.0002488 0 0 0; 0.0003733 0 0 0; 0.0004977 0 0 0; 0.0006221 0 0 0]  x5=0  V1=ones(3,3)  V2=ones(3,3)  I1=ones(3,3)  I2=ones(3,3)  nHarmo=1  Measurements=None
  Eesti_EJ_—_Balti_EJ_330_kV_CN_34682059_330000_CN_34685101_330000 : powerlib/Elements/Distributed Parameters Line  Phases=3  Frequency=60  Resistance=[0.01273 0.3864]  Inductance="[0.9337e-3  4.1264e-3]"  Capacitance=[12.74e-9 7.751e-9]  Length=21.7388  x1=[0 0 0 0; 0.0001244 0 0 0; 0.0002488 0 0 0; 0.0003733 0 0 0; 0.0004977 0 0 0; 0.0006221 0 0 0]  x2=[0 0 0 0; 0.0001244 0 0 0; 0.0002488 0 0 0; 0.0003733 0 0 0; 0.0004977 0 0 0; 0.0006221 0 0 0]  x3=[0 0 0 0; 0.0001244 0 0 0; 0.0002488 0 0 0; 0.0003733 0 0 0; 0.0004977 0 0 0; 0.0006221 0 0 0]  x4=[0 0 0 0; 0.0001244 0 0 0; 0.0002488 0 0 0; 0.0003733 0 0 0; 0.0004977 0 0 0; 0.0006221 0 0 0]  x5=0  V1=ones(3,3)  V2=ones(3,3)  I1=ones(3,3)  I2=ones(3,3)  nHarmo=1  Measurements=None
  Eesti_EJ_—_Paide_330_kV_CN_34685101_330000_CN_35343343_330000 : powerlib/Elements/Distributed Parameters Line  Phases=3  Frequency=60  Resistance=[0.01273 0.3864]  Inductance="[0.9337e-3  4.1264e-3]"  Capacitance=[12.74e-9 7.751e-9]  Length=13.6908  x1=[0 0 0 0; 0.0001244 0 0 0; 0.0002488 0 0 0; 0.0003733 0 0 0; 0.0004977 0 0 0; 0.0006221 0 0 0]  x2=[0 0 0 0; 0.0001244 0 0 0; 0.0002488 0 0 0; 0.0003733 0 0 0; 0.0004977 0 0 0; 0.0006221 0 0 0]  x3=[0 0 0 0; 0.0001244 0 0 0; 0.0002488 0 0 0; 0.0003733 0 0 0; 0.0004977 0 0 0; 0.0006221 0 0 0]  x4=[0 0 0 0; 0.0001244 0 0 0; 0.0002488 0 0 0; 0.0003733 0 0 0; 0.0004977 0 0 0; 0.0006221 0 0 0]  x5=0  V1=ones(3,3)  V2=ones(3,3)  I1=ones(3,3)  I2=ones(3,3)  nHarmo=1  Measurements=None
  Eesti_EJ_—_Püssi_330_kV_CN_34920675_330000_CN_34685101_330000 : powerlib/Elements/Distributed Parameters Line  Phases=3  Frequency=60  Resistance=[0.01273 0.3864]  Inductance="[0.9337e-3  4.1264e-3]"  Capacitance=[12.74e-9 7.751e-9]  Length=51.0804  x1=[0 0 0 0; 0.0001244 0 0 0; 0.0002488 0 0 0; 0.0003733 0 0 0; 0.0004977 0 0 0; 0.0006221 0 0 0]  x2=[0 0 0 0; 0.0001244 0 0 0; 0.0002488 0 0 0; 0.0003733 0 0 0; 0.0004977 0 0 0; 0.0006221 0 0 0]  x3=[0 0 0 0; 0.0001244 0 0 0; 0.0002488 0 0 0; 0.0003733 0 0 0; 0.0004977 0 0 0; 0.0006221 0 0 0]  x4=[0 0 0 0; 0.0001244 0 0 0; 0.0002488 0 0 0; 0.0003733 0 0 0; 0.0004977 0 0 0; 0.0006221 0 0 0]  x5=0  V1=ones(3,3)  V2=ones(3,3)  I1=ones(3,3)  I2=ones(3,3)  nHarmo=1  Measurements=None
  Egglfing___Rotthalmünster___Ering_CN_133669362_110000_CN_81540198_110000 : powerlib/Elements/Distributed Parameters Line  Phases=3  Frequency=60  Resistance=[0.01273 0.3864]  Inductance="[0.9337e-3  4.1264e-3]"  Capacitance=[12.74e-9 7.751e-9]  Length=100  x1=[0 0 0 0; 0.0001244 0 0 0; 0.0002488 0 0 0; 0.0003733 0 0 0; 0.0004977 0 0 0; 0.0006221 0 0 0]  x2=[0 0 0 0; 0.0001244 0 0 0; 0.0002488 0 0 0; 0.0003733 0 0 0; 0.0004977 0 0 0; 0.0006221 0 0 0]  x3=[0 0 0 0; 0.0001244 0 0 0; 0.0002488 0 0 0; 0.0003733 0 0 0; 0.0004977 0 0 0; 0.0006221 0 0 0]  x4=[0 0 0 0; 0.0001244 0 0 0; 0.0002488 0 0 0; 0.0003733 0 0 0; 0.0004977 0 0 0; 0.0006221 0 0 0]  x5=0  V1=ones(3,3)  V2=ones(3,3)  I1=ones(3,3)  I2=ones(3,3)  nHarmo=1  Measurements=None
  Egglfing___Rotthalmünster___Ering_CN_133669362_110000_CN_95972388_110000 : powerlib/Elements/Distributed Parameters Line  Phases=3  Frequency=60  Resistance=[0.01273 0.3864]  Inductance="[0.9337e-3  4.1264e-3]"  Capacitance=[12.74e-9 7.751e-9]  Length=100  x1=[0 0 0 0; 0.0001244 0 0 0; 0.0002488 0 0 0; 0.0003733 0 0 0; 0.0004977 0 0 0; 0.0006221 0 0 0]  x2=[0 0 0 0; 0.0001244 0 0 0; 0.0002488 0 0 0; 0.0003733 0 0 0; 0.0004977 0 0 0; 0.0006221 0 0 0]  x3=[0 0 0 0; 0.0001244 0 0 0; 0.0002488 0 0 0; 0.0003733 0 0 0; 0.0004977 0 0 0; 0.0006221 0 0 0]  x4=[0 0 0 0; 0.0001244 0 0 0; 0.0002488 0 0 0; 0.0003733 0 0 0; 0.0004977 0 0 0; 0.0006221 0 0 0]  x5=0  V1=ones(3,3)  V2=ones(3,3)  I1=ones(3,3)  I2=ones(3,3)  nHarmo=1  Measurements=None
  Eibesbrunn___Bockfließ_CN_28504203_110000_CN_123444716_110000 : powerlib/Elements/Distributed Parameters Line  Phases=3  Frequency=60  Resistance=[0.01273 0.3864]  Inductance="[0.9337e-3  4.1264e-3]"  Capacitance=[12.74e-9 7.751e-9]  Length=100  x1=[0 0 0 0; 0.0001244 0 0 0; 0.0002488 0 0 0; 0.0003733 0 0 0; 0.0004977 0 0 0; 0.0006221 0 0 0]  x2=[0 0 0 0; 0.0001244 0 0 0; 0.0002488 0 0 0; 0.0003733 0 0 0; 0.0004977 0 0 0; 0.0006221 0 0 0]  x3=[0 0 0 0; 0.0001244 0 0 0; 0.0002488 0 0 0; 0.0003733 0 0 0; 0.0004977 0 0 0; 0.0006221 0 0 0]  x4=[0 0 0 0; 0.0001244 0 0 0; 0.0002488 0 0 0; 0.0003733 0 0 0; 0.0004977 0 0 0; 0.0006221 0 0 0]  x5=0  V1=ones(3,3)  V2=ones(3,3)  I1=ones(3,3)  I2=ones(3,3)  nHarmo=1  Measurements=None
  Eibesbrunn___Bockfließ_CN_28504203_110000_CN_24253250_110000 : powerlib/Elements/Distributed Parameters Line  Phases=3  Frequency=60  Resistance=[0.01273 0.3864]  Inductance="[0.9337e-3  4.1264e-3]"  Capacitance=[12.74e-9 7.751e-9]  Length=100  x1=[0 0 0 0; 0.0001244 0 0 0; 0.0002488 0 0 0; 0.0003733 0 0 0; 0.0004977 0 0 0; 0.0006221 0 0 0]  x2=[0 0 0 0; 0.0001244 0 0 0; 0.0002488 0 0 0; 0.0003733 0 0 0; 0.0004977 0 0 0; 0.0006221 0 0 0]  x3=[0 0 0 0; 0.0001244 0 0 0; 0.0002488 0 0 0; 0.0003733 0 0 0; 0.0004977 0 0 0; 0.0006221 0 0 0]  x4=[0 0 0 0; 0.0001244 0 0 0; 0.0002488 0 0 0; 0.0003733 0 0 0; 0.0004977 0 0 0; 0.0006221 0 0 0]  x5=0  V1=ones(3,3)  V2=ones(3,3)  I1=ones(3,3)  I2=ones(3,3)  nHarmo=1  Measurements=None
  Ernsthofen___Hütte_Linz_CN_29563097_110000_CN_93370554_110000 : powerlib/Elements/Distributed Parameters Line  Phases=3  Frequency=60  Resistance=[0.01273 0.3864]  Inductance="[0.9337e-3  4.1264e-3]"  Capacitance=[12.74e-9 7.751e-9]  Length=100  x1=[0 0 0 0; 0.0001244 0 0 0; 0.0002488 0 0 0; 0.0003733 0 0 0; 0.0004977 0 0 0; 0.0006221 0 0 0]  x2=[0 0 0 0; 0.0001244 0 0 0; 0.0002488 0 0 0; 0.0003733 0 0 0; 0.0004977 0 0 0; 0.0006221 0 0 0]  x3=[0 0 0 0; 0.0001244 0 0 0; 0.0002488 0 0 0; 0.0003733 0 0 0; 0.0004977 0 0 0; 0.0006221 0 0 0]  x4=[0 0 0 0; 0.0001244 0 0 0; 0.0002488 0 0 0; 0.0003733 0 0 0; 0.0004977 0 0 0; 0.0006221 0 0 0]  x5=0  V1=ones(3,3)  V2=ones(3,3)  I1=ones(3,3)  I2=ones(3,3)  nHarmo=1  Measurements=None
  Ernsthofen___St__Pantaleon_CN_95828351_110000_CN_27763479_110000 : powerlib/Elements/Distributed Parameters Line  Phases=3  Frequency=60  Resistance=[0.01273 0.3864]  Inductance="[0.9337e-3  4.1264e-3]"  Capacitance=[12.74e-9 7.751e-9]  Length=100  x1=[0 0 0 0; 0.0001244 0 0 0; 0.0002488 0 0 0; 0.0003733 0 0 0; 0.0004977 0 0 0; 0.0006221 0 0 0]  x2=[0 0 0 0; 0.0001244 0 0 0; 0.0002488 0 0 0; 0.0003733 0 0 0; 0.0004977 0 0 0; 0.0006221 0 0 0]  x3=[0 0 0 0; 0.0001244 0 0 0; 0.0002488 0 0 0; 0.0003733 0 0 0; 0.0004977 0 0 0; 0.0006221 0 0 0]  x4=[0 0 0 0; 0.0001244 0 0 0; 0.0002488 0 0 0; 0.0003733 0 0 0; 0.0004977 0 0 0; 0.0006221 0 0 0]  x5=0  V1=ones(3,3)  V2=ones(3,3)  I1=ones(3,3)  I2=ones(3,3)  nHarmo=1  Measurements=None
  Ernsthofen___St__Pantaleon_CN_95828351_110000_CN_33064531_110000 : powerlib/Elements/Distributed Parameters Line  Phases=3  Frequency=60  Resistance=[0.01273 0.3864]  Inductance="[0.9337e-3  4.1264e-3]"  Capacitance=[12.74e-9 7.751e-9]  Length=100  x1=[0 0 0 0; 0.0001244 0 0 0; 0.0002488 0 0 0; 0.0003733 0 0 0; 0.0004977 0 0 0; 0.0006221 0 0 0]  x2=[0 0 0 0; 0.0001244 0 0 0; 0.0002488 0 0 0; 0.0003733 0 0 0; 0.0004977 0 0 0; 0.0006221 0 0 0]  x3=[0 0 0 0; 0.0001244 0 0 0; 0.0002488 0 0 0; 0.0003733 0 0 0; 0.0004977 0 0 0; 0.0006221 0 0 0]  x4=[0 0 0 0; 0.0001244 0 0 0; 0.0002488 0 0 0; 0.0003733 0 0 0; 0.0004977 0 0 0; 0.0006221 0 0 0]  x5=0  V1=ones(3,3)  V2=ones(3,3)  I1=ones(3,3)  I2=ones(3,3)  nHarmo=1  Measurements=None
  Frastanz___Feldkirch_weiß_CN_169304139_110000_CN_32293834_110000 : powerlib/Elements/Distributed Parameters Line  Phases=3  Frequency=60  Resistance=[0.01273 0.3864]  Inductance="[0.9337e-3  4.1264e-3]"  Capacitance=[12.74e-9 7.751e-9]  Length=100  x1=[0 0 0 0; 0.0001244 0 0 0; 0.0002488 0 0 0; 0.0003733 0 0 0; 0.0004977 0 0 0; 0.0006221 0 0 0]  x2=[0 0 0 0; 0.0001244 0 0 0; 0.0002488 0 0 0; 0.0003733 0 0 0; 0.0004977 0 0 0; 0.0006221 0 0 0]  x3=[0 0 0 0; 0.0001244 0 0 0; 0.0002488 0 0 0; 0.0003733 0 0 0; 0.0004977 0 0 0; 0.0006221 0 0 0]  x4=[0 0 0 0; 0.0001244 0 0 0; 0.0002488 0 0 0; 0.0003733 0 0 0; 0.0004977 0 0 0; 0.0006221 0 0 0]  x5=0  V1=ones(3,3)  V2=ones(3,3)  I1=ones(3,3)  I2=ones(3,3)  nHarmo=1  Measurements=None
  Funsingau___Zell_CN_156973414_110000_CN_106512774_110000 : powerlib/Elements/Distributed Parameters Line  Phases=3  Frequency=60  Resistance=[0.01273 0.3864]  Inductance="[0.9337e-3  4.1264e-3]"  Capacitance=[12.74e-9 7.751e-9]  Length=100  x1=[0 0 0 0; 0.0001244 0 0 0; 0.0002488 0 0 0; 0.0003733 0 0 0; 0.0004977 0 0 0; 0.0006221 0 0 0]  x2=[0 0 0 0; 0.0001244 0 0 0; 0.0002488 0 0 0; 0.0003733 0 0 0; 0.0004977 0 0 0; 0.0006221 0 0 0]  x3=[0 0 0 0; 0.0001244 0 0 0; 0.0002488 0 0 0; 0.0003733 0 0 0; 0.0004977 0 0 0; 0.0006221 0 0 0]  x4=[0 0 0 0; 0.0001244 0 0 0; 0.0002488 0 0 0; 0.0003733 0 0 0; 0.0004977 0 0 0; 0.0006221 0 0 0]  x5=0  V1=ones(3,3)  V2=ones(3,3)  I1=ones(3,3)  I2=ones(3,3)  nHarmo=1  Measurements=None
  G_100872499_Kraftwerk_Imst : powerlib/Electrical Sources/Three-Phase Source  Voltage=25e3  PhaseAngle=0  Frequency=60  InternalConnection=Yg  SpecifyImpedance=on  Resistance=0.8929  Inductance=16.58e-3  ShortCircuitLevel=100e6  BaseVoltage=25e3  XRratio=7  BusType=swing  Pref=0  Qref=0  Qmin=-inf  Qmax=inf
  G_102702768_Kraftwerk_Dießbach : powerlib/Electrical Sources/Three-Phase Source  Voltage=25e3  PhaseAngle=0  Frequency=60  InternalConnection=Yg  SpecifyImpedance=on  Resistance=0.8929  Inductance=16.58e-3  ShortCircuitLevel=100e6  BaseVoltage=25e3  XRratio=7  BusType=swing  Pref=0  Qref=0  Qmin=-inf  Qmax=inf
  G_106512774_Kraftwerk_Funsingau : powerlib/Electrical Sources/Three-Phase Source  Voltage=25e3  PhaseAngle=0  Frequency=60  InternalConnection=Yg  SpecifyImpedance=on  Resistance=0.8929  Inductance=16.58e-3  ShortCircuitLevel=100e6  BaseVoltage=25e3  XRratio=7  BusType=swing  Pref=0  Qref=0  Qmin=-inf  Qmax=inf
  G_118134590_Kraftwerk_Krippau : powerlib/Electrical Sources/Three-Phase Source  Voltage=25e3  PhaseAngle=0  Frequency=60  InternalConnection=Yg  SpecifyImpedance=on  Resistance=0.8929  Inductance=16.58e-3  ShortCircuitLevel=100e6  BaseVoltage=25e3  XRratio=7  BusType=swing  Pref=0  Qref=0  Qmin=-inf  Qmax=inf
  G_118135035_Kraftwerk_Altenmarkt : powerlib/Electrical Sources/Three-Phase Source  Voltage=25e3  PhaseAngle=0  Frequency=60  InternalConnection=Yg  SpecifyImpedance=on  Resistance=0.8929  Inductance=16.58e-3  ShortCircuitLevel=100e6  BaseVoltage=25e3  XRratio=7  BusType=swing  Pref=0  Qref=0  Qmin=-inf  Qmax=inf
  G_122776766_Wasserkraftwerk_Opponitz : powerlib/Electrical Sources/Three-Phase Source  Voltage=25e3  PhaseAngle=0  Frequency=60  InternalConnection=Yg  SpecifyImpedance=on  Resistance=0.8929  Inductance=16.58e-3  ShortCircuitLevel=100e6  BaseVoltage=25e3  XRratio=7  BusType=swing  Pref=0  Qref=0  Qmin=-inf  Qmax=inf
  G_122820367_Kraftwerk_Annabrücke : powerlib/Electrical Sources/Three-Phase Source  Voltage=25e3  PhaseAngle=0  Frequency=60  InternalConnection=Yg  SpecifyImpedance=on  Resistance=0.8929  Inductance=16.58e-3  ShortCircuitLevel=100e6  BaseVoltage=25e3  XRratio=7  BusType=swing  Pref=0  Qref=0  Qmin=-inf  Qmax=inf
  G_123588260_Kraftwerk_Rosegg_St__Jakob : powerlib/Electrical Sources/Three-Phase Source  Voltage=25e3  PhaseAngle=0  Frequency=60  InternalConnection=Yg  SpecifyImpedance=on  Resistance=0.8929  Inductance=16.58e-3  ShortCircuitLevel=100e6  BaseVoltage=25e3  XRratio=7  BusType=swing  Pref=0  Qref=0  Qmin=-inf  Qmax=inf
  G_123754668_Fernheizkraftwerk_Linz_Süd : powerlib/Electrical Sources/Three-Phase Source  Voltage=25e3  PhaseAngle=0  Frequency=60  InternalConnection=Yg  SpecifyImpedance=on  Resistance=0.8929  Inductance=16.58e-3  ShortCircuitLevel=100e6  BaseVoltage=25e3  XRratio=7  BusType=swing  Pref=0  Qref=0  Qmin=-inf  Qmax=inf
  G_156083802_Kraftwerk_Kühtai : powerlib/Electrical Sources/Three-Phase Source  Voltage=25e3  PhaseAngle=0  Frequency=60  InternalConnection=Yg  SpecifyImpedance=on  Resistance=0.8929  Inductance=16.58e-3  ShortCircuitLevel=100e6  BaseVoltage=25e3  XRratio=7  BusType=swing  Pref=0  Qref=0  Qmin=-inf  Qmax=inf
  G_15734776_Heizkraftwerk_Linz_Mitte : powerlib/Electrical Sources/Three-Phase Source  Voltage=25e3  PhaseAngle=0  Frequency=60  InternalConnection=Yg  SpecifyImpedance=on  Resistance=0.8929  Inductance=16.58e-3  ShortCircuitLevel=100e6  BaseVoltage=25e3  XRratio=7  BusType=swing  Pref=0  Qref=0  Qmin=-inf  Qmax=inf
  G_176377270_Kraftwerk_Malta_Oberstufe : powerlib/Electrical Sources/Three-Phase Source  Voltage=25e3  PhaseAngle=0  Frequency=60  InternalConnection=Yg  SpecifyImpedance=on  Resistance=0.8929  Inductance=16.58e-3  ShortCircuitLevel=100e6  BaseVoltage=25e3  XRratio=7  BusType=swing  Pref=0  Qref=0  Qmin=-inf  Qmax=inf
  G_265791084_Kiisa_AREJ : powerlib/Electrical Sources/Three-Phase Source  Voltage=110000  PhaseAngle=0  Frequency=60  InternalConnection=Yg  SpecifyImpedance=on  Resistance=0.8929  Inductance=16.58e-3  ShortCircuitLevel=100e6  BaseVoltage=110000  XRratio=7  BusType=swing  Pref=250000000  Qref=0  Qmin=-inf  Qmax=inf
  G_27661875_Kraftwerk_Passau_Ingling : powerlib/Electrical Sources/Three-Phase Source  Voltage=25e3  PhaseAngle=0  Frequency=60  InternalConnection=Yg  SpecifyImpedance=on  Resistance=0.8929  Inductance=16.58e-3  ShortCircuitLevel=100e6  BaseVoltage=25e3  XRratio=7  BusType=swing  Pref=0  Qref=0  Qmin=-inf  Qmax=inf
  G_30880774_Achenseekraftwerk : powerlib/Electrical Sources/Three-Phase Source  Voltage=25e3  PhaseAngle=0  Frequency=60  InternalConnection=Yg  SpecifyImpedance=on  Resistance=0.8929  Inductance=16.58e-3  ShortCircuitLevel=100e6  BaseVoltage=25e3  XRratio=7  BusType=swing  Pref=0  Qref=0  Qmin=-inf  Qmax=inf
  G_30893241_Kraftwerk_Fulpmes : powerlib/Electrical Sources/Three-Phase Source  Voltage=25e3  PhaseAngle=0  Frequency=60  InternalConnection=Yg  SpecifyImpedance=on  Resistance=0.8929  Inductance=16.58e-3  ShortCircuitLevel=100e6  BaseVoltage=25e3  XRratio=7  BusType=swing  Pref=0  Qref=0  Qmin=-inf  Qmax=inf
  G_316403914_BürgerInnen_Solarkraftwerk_Hietzing : powerlib/Electrical Sources/Three-Phase Source  Voltage=25e3  PhaseAngle=0  Frequency=60  InternalConnection=Yg  SpecifyImpedance=on  Resistance=0.8929  Inductance=16.58e-3  ShortCircuitLevel=100e6  BaseVoltage=25e3  XRratio=7  BusType=swing  Pref=0  Qref=0  Qmin=-inf  Qmax=inf
  G_32497342_Wasserkraftwerk_Abwinden_Asten : powerlib/Electrical Sources/Three-Phase Source  Voltage=25e3  PhaseAngle=0  Frequency=60  InternalConnection=Yg  SpecifyImpedance=on  Resistance=0.8929  Inductance=16.58e-3  ShortCircuitLevel=100e6  BaseVoltage=25e3  XRratio=7  BusType=swing  Pref=0  Qref=0  Qmin=-inf  Qmax=inf
  G_33062622_Kraftwerk_Staning : powerlib/Electrical Sources/Three-Phase Source  Voltage=25e3  PhaseAngle=0  Frequency=60  InternalConnection=Yg  SpecifyImpedance=on  Resistance=0.8929  Inductance=16.58e-3  ShortCircuitLevel=100e6  BaseVoltage=25e3  XRratio=7  BusType=swing  Pref=0  Qref=0  Qmin=-inf  Qmax=inf
  G_34682060_Balti_Elektrijaam : powerlib/Electrical Sources/Three-Phase Source  Voltage=110000  PhaseAngle=0  Frequency=60  InternalConnection=Yg  SpecifyImpedance=on  Resistance=0.8929  Inductance=16.58e-3  ShortCircuitLevel=100e6  BaseVoltage=110000  XRratio=7  BusType=swing  Pref=0  Qref=0  Qmin=-inf  Qmax=inf
  G_34682061_ : powerlib/Electrical Sources/Three-Phase Source  Voltage=330000  PhaseAngle=0  Frequency=60  InternalConnection=Yg  SpecifyImpedance=on  Resistance=0.8929  Inductance=16.58e-3  ShortCircuitLevel=100e6  BaseVoltage=330000  XRratio=7  BusType=swing  Pref=0  Qref=0  Qmin=-inf  Qmax=inf
  G_39596992_Pumpspeicherkraftwerk_Ottenstein : powerlib/Electrical Sources/Three-Phase Source  Voltage=25e3  PhaseAngle=0  Frequency=60  InternalConnection=Yg  SpecifyImpedance=on  Resistance=0.8929  Inductance=16.58e-3  ShortCircuitLevel=100e6  BaseVoltage=25e3  XRratio=7  BusType=swing  Pref=0  Qref=0  Qmin=-inf  Qmax=inf
  G_41970883_Kraftwerk_Arnstein : powerlib/Electrical Sources/Three-Phase Source  Voltage=25e3  PhaseAngle=0  Frequency=60  InternalConnection=Yg  SpecifyImpedance=on  Resistance=0.8929  Inductance=16.58e-3  ShortCircuitLevel=100e6  BaseVoltage=25e3  XRratio=7  BusType=swing  Pref=0  Qref=0  Qmin=-inf  Qmax=inf
  G_47001764_Kraftwerk_Theiß : powerlib/Electrical Sources/Three-Phase Source  Voltage=25e3  PhaseAngle=0  Frequency=60  InternalConnection=Yg  SpecifyImpedance=on  Resistance=0.8929  Inductance=16.58e-3  ShortCircuitLevel=100e6  BaseVoltage=25e3  XRratio=7  BusType=swing  Pref=0  Qref=0  Qmin=-inf  Qmax=inf
  G_62238576_Kraftwerk_Häusling : powerlib/Electrical Sources/Three-Phase Source  Voltage=25e3  PhaseAngle=0  Frequency=60  InternalConnection=Yg  SpecifyImpedance=on  Resistance=0.8929  Inductance=16.58e-3  ShortCircuitLevel=100e6  BaseVoltage=25e3  XRratio=7  BusType=swing  Pref=0  Qref=0  Qmin=-inf  Qmax=inf
  G_83805041_Kraftstation_Rottau : powerlib/Electrical Sources/Three-Phase Source  Voltage=25e3  PhaseAngle=0  Frequency=60  InternalConnection=Yg  SpecifyImpedance=on  Resistance=0.8929  Inductance=16.58e-3  ShortCircuitLevel=100e6  BaseVoltage=25e3  XRratio=7  BusType=swing  Pref=0  Qref=0  Qmin=-inf  Qmax=inf
  G_84526686_Kraftwerk_Obervellach : powerlib/Electrical Sources/Three-Phase Source  Voltage=25e3  PhaseAngle=0  Frequency=60  InternalConnection=Yg  SpecifyImpedance=on  Resistance=0.8929  Inductance=16.58e-3  ShortCircuitLevel=100e6  BaseVoltage=25e3  XRratio=7  BusType=swing  Pref=0  Qref=0  Qmin=-inf  Qmax=inf
  G_85291082_KW_Amlach : powerlib/Electrical Sources/Three-Phase Source  Voltage=25e3  PhaseAngle=0  Frequency=60  InternalConnection=Yg  SpecifyImpedance=on  Resistance=0.8929  Inductance=16.58e-3  ShortCircuitLevel=100e6  BaseVoltage=25e3  XRratio=7  BusType=swing  Pref=0  Qref=0  Qmin=-inf  Qmax=inf
  G_85673117_Kraftwerk_Losenstein : powerlib/Electrical Sources/Three-Phase Source  Voltage=25e3  PhaseAngle=0  Frequency=60  InternalConnection=Yg  SpecifyImpedance=on  Resistance=0.8929  Inductance=16.58e-3  ShortCircuitLevel=100e6  BaseVoltage=25e3  XRratio=7  BusType=swing  Pref=0  Qref=0  Qmin=-inf  Qmax=inf
  G_86299764_KW_Zirknitz : powerlib/Electrical Sources/Three-Phase Source  Voltage=25e3  PhaseAngle=0  Frequency=60  InternalConnection=Yg  SpecifyImpedance=on  Resistance=0.8929  Inductance=16.58e-3  ShortCircuitLevel=100e6  BaseVoltage=25e3  XRratio=7  BusType=swing  Pref=0  Qref=0  Qmin=-inf  Qmax=inf
  G_86321271_KW_Ferlach : powerlib/Electrical Sources/Three-Phase Source  Voltage=25e3  PhaseAngle=0  Frequency=60  InternalConnection=Yg  SpecifyImpedance=on  Resistance=0.8929  Inductance=16.58e-3  ShortCircuitLevel=100e6  BaseVoltage=25e3  XRratio=7  BusType=swing  Pref=0  Qref=0  Qmin=-inf  Qmax=inf
  G_86331083_Kraftwerk_Nassfeld : powerlib/Electrical Sources/Three-Phase Source  Voltage=25e3  PhaseAngle=0  Frequency=60  InternalConnection=Yg  SpecifyImpedance=on  Resistance=0.8929  Inductance=16.58e-3  ShortCircuitLevel=100e6  BaseVoltage=25e3  XRratio=7  BusType=swing  Pref=0  Qref=0  Qmin=-inf  Qmax=inf
  G_86331084_Kraftwerk_Böckstein : powerlib/Electrical Sources/Three-Phase Source  Voltage=25e3  PhaseAngle=0  Frequency=60  InternalConnection=Yg  SpecifyImpedance=on  Resistance=0.8929  Inductance=16.58e-3  ShortCircuitLevel=100e6  BaseVoltage=25e3  XRratio=7  BusType=swing  Pref=0  Qref=0  Qmin=-inf  Qmax=inf
  G_94098464_KW_Uttendorf : powerlib/Electrical Sources/Three-Phase Source  Voltage=25e3  PhaseAngle=0  Frequency=60  InternalConnection=Yg  SpecifyImpedance=on  Resistance=0.8929  Inductance=16.58e-3  ShortCircuitLevel=100e6  BaseVoltage=25e3  XRratio=7  BusType=swing  Pref=0  Qref=0  Qmin=-inf  Qmax=inf
  G_94149192_KW_Schneiderau : powerlib/Electrical Sources/Three-Phase Source  Voltage=25e3  PhaseAngle=0  Frequency=60  InternalConnection=Yg  SpecifyImpedance=on  Resistance=0.8929  Inductance=16.58e-3  ShortCircuitLevel=100e6  BaseVoltage=25e3  XRratio=7  BusType=swing  Pref=0  Qref=0  Qmin=-inf  Qmax=inf
  G_94412177_Kraftwerk_Langkampfen : powerlib/Electrical Sources/Three-Phase Source  Voltage=25e3  PhaseAngle=0  Frequency=60  InternalConnection=Yg  SpecifyImpedance=on  Resistance=0.8929  Inductance=16.58e-3  ShortCircuitLevel=100e6  BaseVoltage=25e3  XRratio=7  BusType=swing  Pref=0  Qref=0  Qmin=-inf  Qmax=inf
  G_95195213_Kraftwerk_Erlauf : powerlib/Electrical Sources/Three-Phase Source  Voltage=25e3  PhaseAngle=0  Frequency=60  InternalConnection=Yg  SpecifyImpedance=on  Resistance=0.8929  Inductance=16.58e-3  ShortCircuitLevel=100e6  BaseVoltage=25e3  XRratio=7  BusType=swing  Pref=0  Qref=0  Qmin=-inf  Qmax=inf
  G_95828353_Kraftwerk_St__Pantaleon_Erla : powerlib/Electrical Sources/Three-Phase Source  Voltage=25e3  PhaseAngle=0  Frequency=60  InternalConnection=Yg  SpecifyImpedance=on  Resistance=0.8929  Inductance=16.58e-3  ShortCircuitLevel=100e6  BaseVoltage=25e3  XRratio=7  BusType=swing  Pref=0  Qref=0  Qmin=-inf  Qmax=inf
  G_96250617_Kraftwerk_Partenstein : powerlib/Electrical Sources/Three-Phase Source  Voltage=25e3  PhaseAngle=0  Frequency=60  InternalConnection=Yg  SpecifyImpedance=on  Resistance=0.8929  Inductance=16.58e-3  ShortCircuitLevel=100e6  BaseVoltage=25e3  XRratio=7  BusType=swing  Pref=0  Qref=0  Qmin=-inf  Qmax=inf
  G_96763013_Kraftwerk_Hieflau : powerlib/Electrical Sources/Three-Phase Source  Voltage=25e3  PhaseAngle=0  Frequency=60  InternalConnection=Yg  SpecifyImpedance=on  Resistance=0.8929  Inductance=16.58e-3  ShortCircuitLevel=100e6  BaseVoltage=25e3  XRratio=7  BusType=swing  Pref=0  Qref=0  Qmin=-inf  Qmax=inf
  G_96837486_Kraftwerk_Weyer : powerlib/Electrical Sources/Three-Phase Source  Voltage=25e3  PhaseAngle=0  Frequency=60  InternalConnection=Yg  SpecifyImpedance=on  Resistance=0.8929  Inductance=16.58e-3  ShortCircuitLevel=100e6  BaseVoltage=25e3  XRratio=7  BusType=swing  Pref=0  Qref=0  Qmin=-inf  Qmax=inf
  G_98291700_Kraftwerk_Lavamünd : powerlib/Electrical Sources/Three-Phase Source  Voltage=25e3  PhaseAngle=0  Frequency=60  InternalConnection=Yg  SpecifyImpedance=on  Resistance=0.8929  Inductance=16.58e-3  ShortCircuitLevel=100e6  BaseVoltage=25e3  XRratio=7  BusType=swing  Pref=0  Qref=0  Qmin=-inf  Qmax=inf
  G_98429378_Kraftwerk_Wald : powerlib/Electrical Sources/Three-Phase Source  Voltage=25e3  PhaseAngle=0  Frequency=60  InternalConnection=Yg  SpecifyImpedance=on  Resistance=0.8929  Inductance=16.58e-3  ShortCircuitLevel=100e6  BaseVoltage=25e3  XRratio=7  BusType=swing  Pref=0  Qref=0  Qmin=-inf  Qmax=inf
  G_99858973_Kraftwerk_Bösdornau : powerlib/Electrical Sources/Three-Phase Source  Voltage=25e3  PhaseAngle=0  Frequency=60  InternalConnection=Yg  SpecifyImpedance=on  Resistance=0.8929  Inductance=16.58e-3  ShortCircuitLevel=100e6  BaseVoltage=25e3  XRratio=7  BusType=swing  Pref=0  Qref=0  Qmin=-inf  Qmax=inf
  Gisingen___Feldkirch_blau_CN_169304139_110000_CN_114715432_110000 : powerlib/Elements/Distributed Parameters Line  Phases=3  Frequency=60  Resistance=[0.01273 0.3864]  Inductance="[0.9337e-3  4.1264e-3]"  Capacitance=[12.74e-9 7.751e-9]  Length=100  x1=[0 0 0 0; 0.0001244 0 0 0; 0.0002488 0 0 0; 0.0003733 0 0 0; 0.0004977 0 0 0; 0.0006221 0 0 0]  x2=[0 0 0 0; 0.0001244 0 0 0; 0.0002488 0 0 0; 0.0003733 0 0 0; 0.0004977 0 0 0; 0.0006221 0 0 0]  x3=[0 0 0 0; 0.0001244 0 0 0; 0.0002488 0 0 0; 0.0003733 0 0 0; 0.0004977 0 0 0; 0.0006221 0 0 0]  x4=[0 0 0 0; 0.0001244 0 0 0; 0.0002488 0 0 0; 0.0003733 0 0 0; 0.0004977 0 0 0; 0.0006221 0 0 0]  x5=0  V1=ones(3,3)  V2=ones(3,3)  I1=ones(3,3)  I2=ones(3,3)  nHarmo=1  Measurements=None
  Gundertshausen___Mattighofen;Wagenham___Mattighofen_CN_185860195_110000_CN_95003268_110000 : powerlib/Elements/Distributed Parameters Line  Phases=3  Frequency=60  Resistance=[0.01273 0.3864]  Inductance="[0.9337e-3  4.1264e-3]"  Capacitance=[12.74e-9 7.751e-9]  Length=100  x1=[0 0 0 0; 0.0001244 0 0 0; 0.0002488 0 0 0; 0.0003733 0 0 0; 0.0004977 0 0 0; 0.0006221 0 0 0]  x2=[0 0 0 0; 0.0001244 0 0 0; 0.0002488 0 0 0; 0.0003733 0 0 0; 0.0004977 0 0 0; 0.0006221 0 0 0]  x3=[0 0 0 0; 0.0001244 0 0 0; 0.0002488 0 0 0; 0.0003733 0 0 0; 0.0004977 0 0 0; 0.0006221 0 0 0]  x4=[0 0 0 0; 0.0001244 0 0 0; 0.0002488 0 0 0; 0.0003733 0 0 0; 0.0004977 0 0 0; 0.0006221 0 0 0]  x5=0  V1=ones(3,3)  V2=ones(3,3)  I1=ones(3,3)  I2=ones(3,3)  nHarmo=1  Measurements=None
  Gundertshausen___Mattighofen_CN_185860195_110000_CN_122462450_110000 : powerlib/Elements/Distributed Parameters Line  Phases=3  Frequency=60  Resistance=[0.01273 0.3864]  Inductance="[0.9337e-3  4.1264e-3]"  Capacitance=[12.74e-9 7.751e-9]  Length=100  x1=[0 0 0 0; 0.0001244 0 0 0; 0.0002488 0 0 0; 0.0003733 0 0 0; 0.0004977 0 0 0; 0.0006221 0 0 0]  x2=[0 0 0 0; 0.0001244 0 0 0; 0.0002488 0 0 0; 0.0003733 0 0 0; 0.0004977 0 0 0; 0.0006221 0 0 0]  x3=[0 0 0 0; 0.0001244 0 0 0; 0.0002488 0 0 0; 0.0003733 0 0 0; 0.0004977 0 0 0; 0.0006221 0 0 0]  x4=[0 0 0 0; 0.0001244 0 0 0; 0.0002488 0 0 0; 0.0003733 0 0 0; 0.0004977 0 0 0; 0.0006221 0 0 0]  x5=0  V1=ones(3,3)  V2=ones(3,3)  I1=ones(3,3)  I2=ones(3,3)  nHarmo=1  Measurements=None
  Gundertshausen___Mattighofen_CN_185860195_110000_CN_97870174_110000 : powerlib/Elements/Distributed Parameters Line  Phases=3  Frequency=60  Resistance=[0.01273 0.3864]  Inductance="[0.9337e-3  4.1264e-3]"  Capacitance=[12.74e-9 7.751e-9]  Length=100  x1=[0 0 0 0; 0.0001244 0 0 0; 0.0002488 0 0 0; 0.0003733 0 0 0; 0.0004977 0 0 0; 0.0006221 0 0 0]  x2=[0 0 0 0; 0.0001244 0 0 0; 0.0002488 0 0 0; 0.0003733 0 0 0; 0.0004977 0 0 0; 0.0006221 0 0 0]  x3=[0 0 0 0; 0.0001244 0 0 0; 0.0002488 0 0 0; 0.0003733 0 0 0; 0.0004977 0 0 0; 0.0006221 0 0 0]  x4=[0 0 0 0; 0.0001244 0 0 0; 0.0002488 0 0 0; 0.0003733 0 0 0; 0.0004977 0 0 0; 0.0006221 0 0 0]  x5=0  V1=ones(3,3)  V2=ones(3,3)  I1=ones(3,3)  I2=ones(3,3)  nHarmo=1  Measurements=None
  Gänserndorf___Neusiedl_an_der_Zaya_CN_96346322_110000_CN_96616299_110000 : powerlib/Elements/Distributed Parameters Line  Phases=3  Frequency=60  Resistance=[0.01273 0.3864]  Inductance="[0.9337e-3  4.1264e-3]"  Capacitance=[12.74e-9 7.751e-9]  Length=100  x1=[0 0 0 0; 0.0001244 0 0 0; 0.0002488 0 0 0; 0.0003733 0 0 0; 0.0004977 0 0 0; 0.0006221 0 0 0]  x2=[0 0 0 0; 0.0001244 0 0 0; 0.0002488 0 0 0; 0.0003733 0 0 0; 0.0004977 0 0 0; 0.0006221 0 0 0]  x3=[0 0 0 0; 0.0001244 0 0 0; 0.0002488 0 0 0; 0.0003733 0 0 0; 0.0004977 0 0 0; 0.0006221 0 0 0]  x4=[0 0 0 0; 0.0001244 0 0 0; 0.0002488 0 0 0; 0.0003733 0 0 0; 0.0004977 0 0 0; 0.0006221 0 0 0]  x5=0  V1=ones(3,3)  V2=ones(3,3)  I1=ones(3,3)  I2=ones(3,3)  nHarmo=1  Measurements=None
  Göming___Riedersbach_CN_97870174_110000_CN_98007002_110000 : powerlib/Elements/Distributed Parameters Line  Phases=3  Frequency=60  Resistance=[0.01273 0.3864]  Inductance="[0.9337e-3  4.1264e-3]"  Capacitance=[12.74e-9 7.751e-9]  Length=100  x1=[0 0 0 0; 0.0001244 0 0 0; 0.0002488 0 0 0; 0.0003733 0 0 0; 0.0004977 0 0 0; 0.0006221 0 0 0]  x2=[0 0 0 0; 0.0001244 0 0 0; 0.0002488 0 0 0; 0.0003733 0 0 0; 0.0004977 0 0 0; 0.0006221 0 0 0]  x3=[0 0 0 0; 0.0001244 0 0 0; 0.0002488 0 0 0; 0.0003733 0 0 0; 0.0004977 0 0 0; 0.0006221 0 0 0]  x4=[0 0 0 0; 0.0001244 0 0 0; 0.0002488 0 0 0; 0.0003733 0 0 0; 0.0004977 0 0 0; 0.0006221 0 0 0]  x5=0  V1=ones(3,3)  V2=ones(3,3)  I1=ones(3,3)  I2=ones(3,3)  nHarmo=1  Measurements=None
  Götzendorf_–_Kledering_CN_28449168_110000_CN_25539194_110000 : powerlib/Elements/Distributed Parameters Line  Phases=3  Frequency=60  Resistance=[0.01273 0.3864]  Inductance="[0.9337e-3  4.1264e-3]"  Capacitance=[12.74e-9 7.751e-9]  Length=100  x1=[0 0 0 0; 0.0001244 0 0 0; 0.0002488 0 0 0; 0.0003733 0 0 0; 0.0004977 0 0 0; 0.0006221 0 0 0]  x2=[0 0 0 0; 0.0001244 0 0 0; 0.0002488 0 0 0; 0.0003733 0 0 0; 0.0004977 0 0 0; 0.0006221 0 0 0]  x3=[0 0 0 0; 0.0001244 0 0 0; 0.0002488 0 0 0; 0.0003733 0 0 0; 0.0004977 0 0 0; 0.0006221 0 0 0]  x4=[0 0 0 0; 0.0001244 0 0 0; 0.0002488 0 0 0; 0.0003733 0 0 0; 0.0004977 0 0 0; 0.0006221 0 0 0]  x5=0  V1=ones(3,3)  V2=ones(3,3)  I1=ones(3,3)  I2=ones(3,3)  nHarmo=1  Measurements=None
  Götzendorf_–_Kledering_CN_28449168_110000_CN_28447213_110000 : powerlib/Elements/Distributed Parameters Line  Phases=3  Frequency=60  Resistance=[0.01273 0.3864]  Inductance="[0.9337e-3  4.1264e-3]"  Capacitance=[12.74e-9 7.751e-9]  Length=100  x1=[0 0 0 0; 0.0001244 0 0 0; 0.0002488 0 0 0; 0.0003733 0 0 0; 0.0004977 0 0 0; 0.0006221 0 0 0]  x2=[0 0 0 0; 0.0001244 0 0 0; 0.0002488 0 0 0; 0.0003733 0 0 0; 0.0004977 0 0 0; 0.0006221 0 0 0]  x3=[0 0 0 0; 0.0001244 0 0 0; 0.0002488 0 0 0; 0.0003733 0 0 0; 0.0004977 0 0 0; 0.0006221 0 0 0]  x4=[0 0 0 0; 0.0001244 0 0 0; 0.0002488 0 0 0; 0.0003733 0 0 0; 0.0004977 0 0 0; 0.0006221 0 0 0]  x5=0  V1=ones(3,3)  V2=ones(3,3)  I1=ones(3,3)  I2=ones(3,3)  nHarmo=1  Measurements=None
  Götzendorf_–_Wr__Neustadt_CN_28449168_110000_CN_97094294_110000 : powerlib/Elements/Distributed Parameters Line  Phases=3  Frequency=60  Resistance=[0.01273 0.3864]  Inductance="[0.9337e-3  4.1264e-3]"  Capacitance=[12.74e-9 7.751e-9]  Length=100  x1=[0 0 0 0; 0.0001244 0 0 0; 0.0002488 0 0 0; 0.0003733 0 0 0; 0.0004977 0 0 0; 0.0006221 0 0 0]  x2=[0 0 0 0; 0.0001244 0 0 0; 0.0002488 0 0 0; 0.0003733 0 0 0; 0.0004977 0 0 0; 0.0006221 0 0 0]  x3=[0 0 0 0; 0.0001244 0 0 0; 0.0002488 0 0 0; 0.0003733 0 0 0; 0.0004977 0 0 0; 0.0006221 0 0 0]  x4=[0 0 0 0; 0.0001244 0 0 0; 0.0002488 0 0 0; 0.0003733 0 0 0; 0.0004977 0 0 0; 0.0006221 0 0 0]  x5=0  V1=ones(3,3)  V2=ones(3,3)  I1=ones(3,3)  I2=ones(3,3)  nHarmo=1  Measurements=None
  Haljala_haruliin_CN_34920691_110000_CN_34920699_110000 : powerlib/Elements/Distributed Parameters Line  Phases=3  Frequency=60  Resistance=[0.01273 0.3864]  Inductance="[0.9337e-3  4.1264e-3]"  Capacitance=[12.74e-9 7.751e-9]  Length=9.9717  x1=[0 0 0 0; 0.0001244 0 0 0; 0.0002488 0 0 0; 0.0003733 0 0 0; 0.0004977 0 0 0; 0.0006221 0 0 0]  x2=[0 0 0 0; 0.0001244 0 0 0; 0.0002488 0 0 0; 0.0003733 0 0 0; 0.0004977 0 0 0; 0.0006221 0 0 0]  x3=[0 0 0 0; 0.0001244 0 0 0; 0.0002488 0 0 0; 0.0003733 0 0 0; 0.0004977 0 0 0; 0.0006221 0 0 0]  x4=[0 0 0 0; 0.0001244 0 0 0; 0.0002488 0 0 0; 0.0003733 0 0 0; 0.0004977 0 0 0; 0.0006221 0 0 0]  x5=0  V1=ones(3,3)  V2=ones(3,3)  I1=ones(3,3)  I2=ones(3,3)  nHarmo=1  Measurements=None
  Haljala_haruliin_CN_34920691_110000_CN_35555161_110000 : powerlib/Elements/Distributed Parameters Line  Phases=3  Frequency=60  Resistance=[0.01273 0.3864]  Inductance="[0.9337e-3  4.1264e-3]"  Capacitance=[12.74e-9 7.751e-9]  Length=24.1997  x1=[0 0 0 0; 0.0001244 0 0 0; 0.0002488 0 0 0; 0.0003733 0 0 0; 0.0004977 0 0 0; 0.0006221 0 0 0]  x2=[0 0 0 0; 0.0001244 0 0 0; 0.0002488 0 0 0; 0.0003733 0 0 0; 0.0004977 0 0 0; 0.0006221 0 0 0]  x3=[0 0 0 0; 0.0001244 0 0 0; 0.0002488 0 0 0; 0.0003733 0 0 0; 0.0004977 0 0 0; 0.0006221 0 0 0]  x4=[0 0 0 0; 0.0001244 0 0 0; 0.0002488 0 0 0; 0.0003733 0 0 0; 0.0004977 0 0 0; 0.0006221 0 0 0]  x5=0  V1=ones(3,3)  V2=ones(3,3)  I1=ones(3,3)  I2=ones(3,3)  nHarmo=1  Measurements=None
  Haljala_haruliin_CN_34920691_110000_CN_35555163_110000 : powerlib/Elements/Distributed Parameters Line  Phases=3  Frequency=60  Resistance=[0.01273 0.3864]  Inductance="[0.9337e-3  4.1264e-3]"  Capacitance=[12.74e-9 7.751e-9]  Length=31.4129  x1=[0 0 0 0; 0.0001244 0 0 0; 0.0002488 0 0 0; 0.0003733 0 0 0; 0.0004977 0 0 0; 0.0006221 0 0 0]  x2=[0 0 0 0; 0.0001244 0 0 0; 0.0002488 0 0 0; 0.0003733 0 0 0; 0.0004977 0 0 0; 0.0006221 0 0 0]  x3=[0 0 0 0; 0.0001244 0 0 0; 0.0002488 0 0 0; 0.0003733 0 0 0; 0.0004977 0 0 0; 0.0006221 0 0 0]  x4=[0 0 0 0; 0.0001244 0 0 0; 0.0002488 0 0 0; 0.0003733 0 0 0; 0.0004977 0 0 0; 0.0006221 0 0 0]  x5=0  V1=ones(3,3)  V2=ones(3,3)  I1=ones(3,3)  I2=ones(3,3)  nHarmo=1  Measurements=None
  Haljala_haruliin_CN_34920691_110000_CN_35555165_110000 : powerlib/Elements/Distributed Parameters Line  Phases=3  Frequency=60  Resistance=[0.01273 0.3864]  Inductance="[0.9337e-3  4.1264e-3]"  Capacitance=[12.74e-9 7.751e-9]  Length=55.2791  x1=[0 0 0 0; 0.0001244 0 0 0; 0.0002488 0 0 0; 0.0003733 0 0 0; 0.0004977 0 0 0; 0.0006221 0 0 0]  x2=[0 0 0 0; 0.0001244 0 0 0; 0.0002488 0 0 0; 0.0003733 0 0 0; 0.0004977 0 0 0; 0.0006221 0 0 0]  x3=[0 0 0 0; 0.0001244 0 0 0; 0.0002488 0 0 0; 0.0003733 0 0 0; 0.0004977 0 0 0; 0.0006221 0 0 0]  x4=[0 0 0 0; 0.0001244 0 0 0; 0.0002488 0 0 0; 0.0003733 0 0 0; 0.0004977 0 0 0; 0.0006221 0 0 0]  x5=0  V1=ones(3,3)  V2=ones(3,3)  I1=ones(3,3)  I2=ones(3,3)  nHarmo=1  Measurements=None
  Haljala_haruliin_CN_34920691_110000_CN_35555166_110000 : powerlib/Elements/Distributed Parameters Line  Phases=3  Frequency=60  Resistance=[0.01273 0.3864]  Inductance="[0.9337e-3  4.1264e-3]"  Capacitance=[12.74e-9 7.751e-9]  Length=55.2558  x1=[0 0 0 0; 0.0001244 0 0 0; 0.0002488 0 0 0; 0.0003733 0 0 0; 0.0004977 0 0 0; 0.0006221 0 0 0]  x2=[0 0 0 0; 0.0001244 0 0 0; 0.0002488 0 0 0; 0.0003733 0 0 0; 0.0004977 0 0 0; 0.0006221 0 0 0]  x3=[0 0 0 0; 0.0001244 0 0 0; 0.0002488 0 0 0; 0.0003733 0 0 0; 0.0004977 0 0 0; 0.0006221 0 0 0]  x4=[0 0 0 0; 0.0001244 0 0 0; 0.0002488 0 0 0; 0.0003733 0 0 0; 0.0004977 0 0 0; 0.0006221 0 0 0]  x5=0  V1=ones(3,3)  V2=ones(3,3)  I1=ones(3,3)  I2=ones(3,3)  nHarmo=1  Measurements=None
  Haljala_haruliin_CN_34920691_110000_CN_35555175_110000 : powerlib/Elements/Distributed Parameters Line  Phases=3  Frequency=60  Resistance=[0.01273 0.3864]  Inductance="[0.9337e-3  4.1264e-3]"  Capacitance=[12.74e-9 7.751e-9]  Length=19.6552  x1=[0 0 0 0; 0.0001244 0 0 0; 0.0002488 0 0 0; 0.0003733 0 0 0; 0.0004977 0 0 0; 0.0006221 0 0 0]  x2=[0 0 0 0; 0.0001244 0 0 0; 0.0002488 0 0 0; 0.0003733 0 0 0; 0.0004977 0 0 0; 0.0006221 0 0 0]  x3=[0 0 0 0; 0.0001244 0 0 0; 0.0002488 0 0 0; 0.0003733 0 0 0; 0.0004977 0 0 0; 0.0006221 0 0 0]  x4=[0 0 0 0; 0.0001244 0 0 0; 0.0002488 0 0 0; 0.0003733 0 0 0; 0.0004977 0 0 0; 0.0006221 0 0 0]  x5=0  V1=ones(3,3)  V2=ones(3,3)  I1=ones(3,3)  I2=ones(3,3)  nHarmo=1  Measurements=None
  Harku_—_Aruküla_330_kV_CN_34968224_330000_CN_204914596_330000 : powerlib/Elements/Distributed Parameters Line  Phases=3  Frequency=60  Resistance=[0.01273 0.3864]  Inductance="[0.9337e-3  4.1264e-3]"  Capacitance=[12.74e-9 7.751e-9]  Length=46.282  x1=[0 0 0 0; 0.0001244 0 0 0; 0.0002488 0 0 0; 0.0003733 0 0 0; 0.0004977 0 0 0; 0.0006221 0 0 0]  x2=[0 0 0 0; 0.0001244 0 0 0; 0.0002488 0 0 0; 0.0003733 0 0 0; 0.0004977 0 0 0; 0.0006221 0 0 0]  x3=[0 0 0 0; 0.0001244 0 0 0; 0.0002488 0 0 0; 0.0003733 0 0 0; 0.0004977 0 0 0; 0.0006221 0 0 0]  x4=[0 0 0 0; 0.0001244 0 0 0; 0.0002488 0 0 0; 0.0003733 0 0 0; 0.0004977 0 0 0; 0.0006221 0 0 0]  x5=0  V1=ones(3,3)  V2=ones(3,3)  I1=ones(3,3)  I2=ones(3,3)  nHarmo=1  Measurements=None
  Harku_—_Aruküla_330_kV_CN_34968224_330000_CN_34682059_330000 : powerlib/Elements/Distributed Parameters Line  Phases=3  Frequency=60  Resistance=[0.01273 0.3864]  Inductance="[0.9337e-3  4.1264e-3]"  Capacitance=[12.74e-9 7.751e-9]  Length=78.6594  x1=[0 0 0 0; 0.0001244 0 0 0; 0.0002488 0 0 0; 0.0003733 0 0 0; 0.0004977 0 0 0; 0.0006221 0 0 0]  x2=[0 0 0 0; 0.0001244 0 0 0; 0.0002488 0 0 0; 0.0003733 0 0 0; 0.0004977 0 0 0; 0.0006221 0 0 0]  x3=[0 0 0 0; 0.0001244 0 0 0; 0.0002488 0 0 0; 0.0003733 0 0 0; 0.0004977 0 0 0; 0.0006221 0 0 0]  x4=[0 0 0 0; 0.0001244 0 0 0; 0.0002488 0 0 0; 0.0003733 0 0 0; 0.0004977 0 0 0; 0.0006221 0 0 0]  x5=0  V1=ones(3,3)  V2=ones(3,3)  I1=ones(3,3)  I2=ones(3,3)  nHarmo=1  Measurements=None
  Harku_—_Aruküla_330_kV_CN_34968224_330000_CN_34935436_330000 : powerlib/Elements/Distributed Parameters Line  Phases=3  Frequency=60  Resistance=[0.01273 0.3864]  Inductance="[0.9337e-3  4.1264e-3]"  Capacitance=[12.74e-9 7.751e-9]  Length=18.865  x1=[0 0 0 0; 0.0001244 0 0 0; 0.0002488 0 0 0; 0.0003733 0 0 0; 0.0004977 0 0 0; 0.0006221 0 0 0]  x2=[0 0 0 0; 0.0001244 0 0 0; 0.0002488 0 0 0; 0.0003733 0 0 0; 0.0004977 0 0 0; 0.0006221 0 0 0]  x3=[0 0 0 0; 0.0001244 0 0 0; 0.0002488 0 0 0; 0.0003733 0 0 0; 0.0004977 0 0 0; 0.0006221 0 0 0]  x4=[0 0 0 0; 0.0001244 0 0 0; 0.0002488 0 0 0; 0.0003733 0 0 0; 0.0004977 0 0 0; 0.0006221 0 0 0]  x5=0  V1=ones(3,3)  V2=ones(3,3)  I1=ones(3,3)  I2=ones(3,3)  nHarmo=1  Measurements=None
  Harku_—_Keila_110_kV_CN_34968224_110000_CN_262229346_110000 : powerlib/Elements/Distributed Parameters Line  Phases=3  Frequency=60  Resistance=[0.01273 0.3864]  Inductance="[0.9337e-3  4.1264e-3]"  Capacitance=[12.74e-9 7.751e-9]  Length=11.9822  x1=[0 0 0 0; 0.0001244 0 0 0; 0.0002488 0 0 0; 0.0003733 0 0 0; 0.0004977 0 0 0; 0.0006221 0 0 0]  x2=[0 0 0 0; 0.0001244 0 0 0; 0.0002488 0 0 0; 0.0003733 0 0 0; 0.0004977 0 0 0; 0.0006221 0 0 0]  x3=[0 0 0 0; 0.0001244 0 0 0; 0.0002488 0 0 0; 0.0003733 0 0 0; 0.0004977 0 0 0; 0.0006221 0 0 0]  x4=[0 0 0 0; 0.0001244 0 0 0; 0.0002488 0 0 0; 0.0003733 0 0 0; 0.0004977 0 0 0; 0.0006221 0 0 0]  x5=0  V1=ones(3,3)  V2=ones(3,3)  I1=ones(3,3)  I2=ones(3,3)  nHarmo=1  Measurements=None
  Harku_—_Keila_110_kV_CN_34968224_110000_CN_34988480_110000 : powerlib/Elements/Distributed Parameters Line  Phases=3  Frequency=60  Resistance=[0.01273 0.3864]  Inductance="[0.9337e-3  4.1264e-3]"  Capacitance=[12.74e-9 7.751e-9]  Length=5.1217  x1=[0 0 0 0; 0.0001244 0 0 0; 0.0002488 0 0 0; 0.0003733 0 0 0; 0.0004977 0 0 0; 0.0006221 0 0 0]  x2=[0 0 0 0; 0.0001244 0 0 0; 0.0002488 0 0 0; 0.0003733 0 0 0; 0.0004977 0 0 0; 0.0006221 0 0 0]  x3=[0 0 0 0; 0.0001244 0 0 0; 0.0002488 0 0 0; 0.0003733 0 0 0; 0.0004977 0 0 0; 0.0006221 0 0 0]  x4=[0 0 0 0; 0.0001244 0 0 0; 0.0002488 0 0 0; 0.0003733 0 0 0; 0.0004977 0 0 0; 0.0006221 0 0 0]  x5=0  V1=ones(3,3)  V2=ones(3,3)  I1=ones(3,3)  I2=ones(3,3)  nHarmo=1  Measurements=None
  Harku_—_Kiisa_110_kV_CN_34935436_110000_CN_34968224_110000 : powerlib/Elements/Distributed Parameters Line  Phases=3  Frequency=60  Resistance=[0.01273 0.3864]  Inductance="[0.9337e-3  4.1264e-3]"  Capacitance=[12.74e-9 7.751e-9]  Length=18.9818  x1=[0 0 0 0; 0.0001244 0 0 0; 0.0002488 0 0 0; 0.0003733 0 0 0; 0.0004977 0 0 0; 0.0006221 0 0 0]  x2=[0 0 0 0; 0.0001244 0 0 0; 0.0002488 0 0 0; 0.0003733 0 0 0; 0.0004977 0 0 0; 0.0006221 0 0 0]  x3=[0 0 0 0; 0.0001244 0 0 0; 0.0002488 0 0 0; 0.0003733 0 0 0; 0.0004977 0 0 0; 0.0006221 0 0 0]  x4=[0 0 0 0; 0.0001244 0 0 0; 0.0002488 0 0 0; 0.0003733 0 0 0; 0.0004977 0 0 0; 0.0006221 0 0 0]  x5=0  V1=ones(3,3)  V2=ones(3,3)  I1=ones(3,3)  I2=ones(3,3)  nHarmo=1  Measurements=None
  Harku_—_Veskimetsa_110_kV_CN_34968224_110000_CN_99350295_110000 : powerlib/Elements/Distributed Parameters Line  Phases=3  Frequency=60  Resistance=[0.01273 0.3864]  Inductance="[0.9337e-3  4.1264e-3]"  Capacitance=[12.74e-9 7.751e-9]  Length=7.899  x1=[0 0 0 0; 0.0001244 0 0 0; 0.0002488 0 0 0; 0.0003733 0 0 0; 0.0004977 0 0 0; 0.0006221 0 0 0]  x2=[0 0 0 0; 0.0001244 0 0 0; 0.0002488 0 0 0; 0.0003733 0 0 0; 0.0004977 0 0 0; 0.0006221 0 0 0]  x3=[0 0 0 0; 0.0001244 0 0 0; 0.0002488 0 0 0; 0.0003733 0 0 0; 0.0004977 0 0 0; 0.0006221 0 0 0]  x4=[0 0 0 0; 0.0001244 0 0 0; 0.0002488 0 0 0; 0.0003733 0 0 0; 0.0004977 0 0 0; 0.0006221 0 0 0]  x5=0  V1=ones(3,3)  V2=ones(3,3)  I1=ones(3,3)  I2=ones(3,3)  nHarmo=1  Measurements=None
  Hart___Edlitz_CN_96989592_110000_CN_96998954_110000 : powerlib/Elements/Distributed Parameters Line  Phases=3  Frequency=60  Resistance=[0.01273 0.3864]  Inductance="[0.9337e-3  4.1264e-3]"  Capacitance=[12.74e-9 7.751e-9]  Length=100  x1=[0 0 0 0; 0.0001244 0 0 0; 0.0002488 0 0 0; 0.0003733 0 0 0; 0.0004977 0 0 0; 0.0006221 0 0 0]  x2=[0 0 0 0; 0.0001244 0 0 0; 0.0002488 0 0 0; 0.0003733 0 0 0; 0.0004977 0 0 0; 0.0006221 0 0 0]  x3=[0 0 0 0; 0.0001244 0 0 0; 0.0002488 0 0 0; 0.0003733 0 0 0; 0.0004977 0 0 0; 0.0006221 0 0 0]  x4=[0 0 0 0; 0.0001244 0 0 0; 0.0002488 0 0 0; 0.0003733 0 0 0; 0.0004977 0 0 0; 0.0006221 0 0 0]  x5=0  V1=ones(3,3)  V2=ones(3,3)  I1=ones(3,3)  I2=ones(3,3)  nHarmo=1  Measurements=None
  Hartberg___Unterrohr_CN_102767009_110000_CN_96734998_110000 : powerlib/Elements/Distributed Parameters Line  Phases=3  Frequency=60  Resistance=[0.01273 0.3864]  Inductance="[0.9337e-3  4.1264e-3]"  Capacitance=[12.74e-9 7.751e-9]  Length=100  x1=[0 0 0 0; 0.0001244 0 0 0; 0.0002488 0 0 0; 0.0003733 0 0 0; 0.0004977 0 0 0; 0.0006221 0 0 0]  x2=[0 0 0 0; 0.0001244 0 0 0; 0.0002488 0 0 0; 0.0003733 0 0 0; 0.0004977 0 0 0; 0.0006221 0 0 0]  x3=[0 0 0 0; 0.0001244 0 0 0; 0.0002488 0 0 0; 0.0003733 0 0 0; 0.0004977 0 0 0; 0.0006221 0 0 0]  x4=[0 0 0 0; 0.0001244 0 0 0; 0.0002488 0 0 0; 0.0003733 0 0 0; 0.0004977 0 0 0; 0.0006221 0 0 0]  x5=0  V1=ones(3,3)  V2=ones(3,3)  I1=ones(3,3)  I2=ones(3,3)  nHarmo=1  Measurements=None
  Hartberg___Unterrohr_CN_102767009_110000_CN_99730272_110000 : powerlib/Elements/Distributed Parameters Line  Phases=3  Frequency=60  Resistance=[0.01273 0.3864]  Inductance="[0.9337e-3  4.1264e-3]"  Capacitance=[12.74e-9 7.751e-9]  Length=100  x1=[0 0 0 0; 0.0001244 0 0 0; 0.0002488 0 0 0; 0.0003733 0 0 0; 0.0004977 0 0 0; 0.0006221 0 0 0]  x2=[0 0 0 0; 0.0001244 0 0 0; 0.0002488 0 0 0; 0.0003733 0 0 0; 0.0004977 0 0 0; 0.0006221 0 0 0]  x3=[0 0 0 0; 0.0001244 0 0 0; 0.0002488 0 0 0; 0.0003733 0 0 0; 0.0004977 0 0 0; 0.0006221 0 0 0]  x4=[0 0 0 0; 0.0001244 0 0 0; 0.0002488 0 0 0; 0.0003733 0 0 0; 0.0004977 0 0 0; 0.0006221 0 0 0]  x5=0  V1=ones(3,3)  V2=ones(3,3)  I1=ones(3,3)  I2=ones(3,3)  nHarmo=1  Measurements=None
  Hessenberg___Bruck_Mur_CN_81611149_110000_CN_88680218_110000 : powerlib/Elements/Distributed Parameters Line  Phases=3  Frequency=60  Resistance=[0.01273 0.3864]  Inductance="[0.9337e-3  4.1264e-3]"  Capacitance=[12.74e-9 7.751e-9]  Length=100  x1=[0 0 0 0; 0.0001244 0 0 0; 0.0002488 0 0 0; 0.0003733 0 0 0; 0.0004977 0 0 0; 0.0006221 0 0 0]  x2=[0 0 0 0; 0.0001244 0 0 0; 0.0002488 0 0 0; 0.0003733 0 0 0; 0.0004977 0 0 0; 0.0006221 0 0 0]  x3=[0 0 0 0; 0.0001244 0 0 0; 0.0002488 0 0 0; 0.0003733 0 0 0; 0.0004977 0 0 0; 0.0006221 0 0 0]  x4=[0 0 0 0; 0.0001244 0 0 0; 0.0002488 0 0 0; 0.0003733 0 0 0; 0.0004977 0 0 0; 0.0006221 0 0 0]  x5=0  V1=ones(3,3)  V2=ones(3,3)  I1=ones(3,3)  I2=ones(3,3)  nHarmo=1  Measurements=None
  Hohe_Wand___Wiener_Neustadt_CN_96358427_110000_CN_99761298_110000 : powerlib/Elements/Distributed Parameters Line  Phases=3  Frequency=60  Resistance=[0.01273 0.3864]  Inductance="[0.9337e-3  4.1264e-3]"  Capacitance=[12.74e-9 7.751e-9]  Length=100  x1=[0 0 0 0; 0.0001244 0 0 0; 0.0002488 0 0 0; 0.0003733 0 0 0; 0.0004977 0 0 0; 0.0006221 0 0 0]  x2=[0 0 0 0; 0.0001244 0 0 0; 0.0002488 0 0 0; 0.0003733 0 0 0; 0.0004977 0 0 0; 0.0006221 0 0 0]  x3=[0 0 0 0; 0.0001244 0 0 0; 0.0002488 0 0 0; 0.0003733 0 0 0; 0.0004977 0 0 0; 0.0006221 0 0 0]  x4=[0 0 0 0; 0.0001244 0 0 0; 0.0002488 0 0 0; 0.0003733 0 0 0; 0.0004977 0 0 0; 0.0006221 0 0 0]  x5=0  V1=ones(3,3)  V2=ones(3,3)  I1=ones(3,3)  I2=ones(3,3)  nHarmo=1  Measurements=None
  Hohenems___Weiler_Klaus;Hohenems___Werben_CN_123689023_110000_CN_100478972_110000 : powerlib/Elements/Distributed Parameters Line  Phases=3  Frequency=60  Resistance=[0.01273 0.3864]  Inductance="[0.9337e-3  4.1264e-3]"  Capacitance=[12.74e-9 7.751e-9]  Length=100  x1=[0 0 0 0; 0.0001244 0 0 0; 0.0002488 0 0 0; 0.0003733 0 0 0; 0.0004977 0 0 0; 0.0006221 0 0 0]  x2=[0 0 0 0; 0.0001244 0 0 0; 0.0002488 0 0 0; 0.0003733 0 0 0; 0.0004977 0 0 0; 0.0006221 0 0 0]  x3=[0 0 0 0; 0.0001244 0 0 0; 0.0002488 0 0 0; 0.0003733 0 0 0; 0.0004977 0 0 0; 0.0006221 0 0 0]  x4=[0 0 0 0; 0.0001244 0 0 0; 0.0002488 0 0 0; 0.0003733 0 0 0; 0.0004977 0 0 0; 0.0006221 0 0 0]  x5=0  V1=ones(3,3)  V2=ones(3,3)  I1=ones(3,3)  I2=ones(3,3)  nHarmo=1  Measurements=None
  Hohenems___Weiler_Klaus;Hohenems___Werben_CN_123689023_110000_CN_169361887_110000 : powerlib/Elements/Distributed Parameters Line  Phases=3  Frequency=60  Resistance=[0.01273 0.3864]  Inductance="[0.9337e-3  4.1264e-3]"  Capacitance=[12.74e-9 7.751e-9]  Length=100  x1=[0 0 0 0; 0.0001244 0 0 0; 0.0002488 0 0 0; 0.0003733 0 0 0; 0.0004977 0 0 0; 0.0006221 0 0 0]  x2=[0 0 0 0; 0.0001244 0 0 0; 0.0002488 0 0 0; 0.0003733 0 0 0; 0.0004977 0 0 0; 0.0006221 0 0 0]  x3=[0 0 0 0; 0.0001244 0 0 0; 0.0002488 0 0 0; 0.0003733 0 0 0; 0.0004977 0 0 0; 0.0006221 0 0 0]  x4=[0 0 0 0; 0.0001244 0 0 0; 0.0002488 0 0 0; 0.0003733 0 0 0; 0.0004977 0 0 0; 0.0006221 0 0 0]  x5=0  V1=ones(3,3)  V2=ones(3,3)  I1=ones(3,3)  I2=ones(3,3)  nHarmo=1  Measurements=None
  Hohenems___Weiler_Klaus;Hohenems___Werben_CN_123689023_110000_CN_61108302_110000 : powerlib/Elements/Distributed Parameters Line  Phases=3  Frequency=60  Resistance=[0.01273 0.3864]  Inductance="[0.9337e-3  4.1264e-3]"  Capacitance=[12.74e-9 7.751e-9]  Length=100  x1=[0 0 0 0; 0.0001244 0 0 0; 0.0002488 0 0 0; 0.0003733 0 0 0; 0.0004977 0 0 0; 0.0006221 0 0 0]  x2=[0 0 0 0; 0.0001244 0 0 0; 0.0002488 0 0 0; 0.0003733 0 0 0; 0.0004977 0 0 0; 0.0006221 0 0 0]  x3=[0 0 0 0; 0.0001244 0 0 0; 0.0002488 0 0 0; 0.0003733 0 0 0; 0.0004977 0 0 0; 0.0006221 0 0 0]  x4=[0 0 0 0; 0.0001244 0 0 0; 0.0002488 0 0 0; 0.0003733 0 0 0; 0.0004977 0 0 0; 0.0006221 0 0 0]  x5=0  V1=ones(3,3)  V2=ones(3,3)  I1=ones(3,3)  I2=ones(3,3)  nHarmo=1  Measurements=None
  Iru_—_Järve_&_Järveküla_—_Järve_110_kV_CN_34968246_110000_CN_34968251_110000 : powerlib/Elements/Distributed Parameters Line  Phases=3  Frequency=60  Resistance=[0.01273 0.3864]  Inductance="[0.9337e-3  4.1264e-3]"  Capacitance=[12.74e-9 7.751e-9]  Length=6.9616  x1=[0 0 0 0; 0.0001244 0 0 0; 0.0002488 0 0 0; 0.0003733 0 0 0; 0.0004977 0 0 0; 0.0006221 0 0 0]  x2=[0 0 0 0; 0.0001244 0 0 0; 0.0002488 0 0 0; 0.0003733 0 0 0; 0.0004977 0 0 0; 0.0006221 0 0 0]  x3=[0 0 0 0; 0.0001244 0 0 0; 0.0002488 0 0 0; 0.0003733 0 0 0; 0.0004977 0 0 0; 0.0006221 0 0 0]  x4=[0 0 0 0; 0.0001244 0 0 0; 0.0002488 0 0 0; 0.0003733 0 0 0; 0.0004977 0 0 0; 0.0006221 0 0 0]  x5=0  V1=ones(3,3)  V2=ones(3,3)  I1=ones(3,3)  I2=ones(3,3)  nHarmo=1  Measurements=None
  Iru_—_Järve_&_Järveküla_—_Järve_110_kV_CN_34968246_110000_CN_72668114_110000 : powerlib/Elements/Distributed Parameters Line  Phases=3  Frequency=60  Resistance=[0.01273 0.3864]  Inductance="[0.9337e-3  4.1264e-3]"  Capacitance=[12.74e-9 7.751e-9]  Length=23.6453  x1=[0 0 0 0; 0.0001244 0 0 0; 0.0002488 0 0 0; 0.0003733 0 0 0; 0.0004977 0 0 0; 0.0006221 0 0 0]  x2=[0 0 0 0; 0.0001244 0 0 0; 0.0002488 0 0 0; 0.0003733 0 0 0; 0.0004977 0 0 0; 0.0006221 0 0 0]  x3=[0 0 0 0; 0.0001244 0 0 0; 0.0002488 0 0 0; 0.0003733 0 0 0; 0.0004977 0 0 0; 0.0006221 0 0 0]  x4=[0 0 0 0; 0.0001244 0 0 0; 0.0002488 0 0 0; 0.0003733 0 0 0; 0.0004977 0 0 0; 0.0006221 0 0 0]  x5=0  V1=ones(3,3)  V2=ones(3,3)  I1=ones(3,3)  I2=ones(3,3)  nHarmo=1  Measurements=None
  Iru_—_Kallavere_110_kV_CN_72668114_110000_CN_29979106_110000 : powerlib/Elements/Distributed Parameters Line  Phases=3  Frequency=60  Resistance=[0.01273 0.3864]  Inductance="[0.9337e-3  4.1264e-3]"  Capacitance=[12.74e-9 7.751e-9]  Length=7.4232  x1=[0 0 0 0; 0.0001244 0 0 0; 0.0002488 0 0 0; 0.0003733 0 0 0; 0.0004977 0 0 0; 0.0006221 0 0 0]  x2=[0 0 0 0; 0.0001244 0 0 0; 0.0002488 0 0 0; 0.0003733 0 0 0; 0.0004977 0 0 0; 0.0006221 0 0 0]  x3=[0 0 0 0; 0.0001244 0 0 0; 0.0002488 0 0 0; 0.0003733 0 0 0; 0.0004977 0 0 0; 0.0006221 0 0 0]  x4=[0 0 0 0; 0.0001244 0 0 0; 0.0002488 0 0 0; 0.0003733 0 0 0; 0.0004977 0 0 0; 0.0006221 0 0 0]  x5=0  V1=ones(3,3)  V2=ones(3,3)  I1=ones(3,3)  I2=ones(3,3)  nHarmo=1  Measurements=None
  Jenbach___Thaur_1;Hall___Thaur_CN_24768685_110000_CN_121265317_110000 : powerlib/Elements/Distributed Parameters Line  Phases=3  Frequency=60  Resistance=[0.01273 0.3864]  Inductance="[0.9337e-3  4.1264e-3]"  Capacitance=[12.74e-9 7.751e-9]  Length=100  x1=[0 0 0 0; 0.0001244 0 0 0; 0.0002488 0 0 0; 0.0003733 0 0 0; 0.0004977 0 0 0; 0.0006221 0 0 0]  x2=[0 0 0 0; 0.0001244 0 0 0; 0.0002488 0 0 0; 0.0003733 0 0 0; 0.0004977 0 0 0; 0.0006221 0 0 0]  x3=[0 0 0 0; 0.0001244 0 0 0; 0.0002488 0 0 0; 0.0003733 0 0 0; 0.0004977 0 0 0; 0.0006221 0 0 0]  x4=[0 0 0 0; 0.0001244 0 0 0; 0.0002488 0 0 0; 0.0003733 0 0 0; 0.0004977 0 0 0; 0.0006221 0 0 0]  x5=0  V1=ones(3,3)  V2=ones(3,3)  I1=ones(3,3)  I2=ones(3,3)  nHarmo=1  Measurements=None
  Jenbach___Thaur_1;Hall___Thaur_CN_24768685_110000_CN_30880774_110000 : powerlib/Elements/Distributed Parameters Line  Phases=3  Frequency=60  Resistance=[0.01273 0.3864]  Inductance="[0.9337e-3  4.1264e-3]"  Capacitance=[12.74e-9 7.751e-9]  Length=100  x1=[0 0 0 0; 0.0001244 0 0 0; 0.0002488 0 0 0; 0.0003733 0 0 0; 0.0004977 0 0 0; 0.0006221 0 0 0]  x2=[0 0 0 0; 0.0001244 0 0 0; 0.0002488 0 0 0; 0.0003733 0 0 0; 0.0004977 0 0 0; 0.0006221 0 0 0]  x3=[0 0 0 0; 0.0001244 0 0 0; 0.0002488 0 0 0; 0.0003733 0 0 0; 0.0004977 0 0 0; 0.0006221 0 0 0]  x4=[0 0 0 0; 0.0001244 0 0 0; 0.0002488 0 0 0; 0.0003733 0 0 0; 0.0004977 0 0 0; 0.0006221 0 0 0]  x5=0  V1=ones(3,3)  V2=ones(3,3)  I1=ones(3,3)  I2=ones(3,3)  nHarmo=1  Measurements=None
  Jenbach___Zell_CN_156973414_110000_CN_23899163_110000 : powerlib/Elements/Distributed Parameters Line  Phases=3  Frequency=60  Resistance=[0.01273 0.3864]  Inductance="[0.9337e-3  4.1264e-3]"  Capacitance=[12.74e-9 7.751e-9]  Length=100  x1=[0 0 0 0; 0.0001244 0 0 0; 0.0002488 0 0 0; 0.0003733 0 0 0; 0.0004977 0 0 0; 0.0006221 0 0 0]  x2=[0 0 0 0; 0.0001244 0 0 0; 0.0002488 0 0 0; 0.0003733 0 0 0; 0.0004977 0 0 0; 0.0006221 0 0 0]  x3=[0 0 0 0; 0.0001244 0 0 0; 0.0002488 0 0 0; 0.0003733 0 0 0; 0.0004977 0 0 0; 0.0006221 0 0 0]  x4=[0 0 0 0; 0.0001244 0 0 0; 0.0002488 0 0 0; 0.0003733 0 0 0; 0.0004977 0 0 0; 0.0006221 0 0 0]  x5=0  V1=ones(3,3)  V2=ones(3,3)  I1=ones(3,3)  I2=ones(3,3)  nHarmo=1  Measurements=None
  Jenbach___Zell_CN_156973414_110000_CN_30880774_110000 : powerlib/Elements/Distributed Parameters Line  Phases=3  Frequency=60  Resistance=[0.01273 0.3864]  Inductance="[0.9337e-3  4.1264e-3]"  Capacitance=[12.74e-9 7.751e-9]  Length=100  x1=[0 0 0 0; 0.0001244 0 0 0; 0.0002488 0 0 0; 0.0003733 0 0 0; 0.0004977 0 0 0; 0.0006221 0 0 0]  x2=[0 0 0 0; 0.0001244 0 0 0; 0.0002488 0 0 0; 0.0003733 0 0 0; 0.0004977 0 0 0; 0.0006221 0 0 0]  x3=[0 0 0 0; 0.0001244 0 0 0; 0.0002488 0 0 0; 0.0003733 0 0 0; 0.0004977 0 0 0; 0.0006221 0 0 0]  x4=[0 0 0 0; 0.0001244 0 0 0; 0.0002488 0 0 0; 0.0003733 0 0 0; 0.0004977 0 0 0; 0.0006221 0 0 0]  x5=0  V1=ones(3,3)  V2=ones(3,3)  I1=ones(3,3)  I2=ones(3,3)  nHarmo=1  Measurements=None
  Jenbach___Zell_CN_156973414_110000_CN_94514064_110000 : powerlib/Elements/Distributed Parameters Line  Phases=3  Frequency=60  Resistance=[0.01273 0.3864]  Inductance="[0.9337e-3  4.1264e-3]"  Capacitance=[12.74e-9 7.751e-9]  Length=100  x1=[0 0 0 0; 0.0001244 0 0 0; 0.0002488 0 0 0; 0.0003733 0 0 0; 0.0004977 0 0 0; 0.0006221 0 0 0]  x2=[0 0 0 0; 0.0001244 0 0 0; 0.0002488 0 0 0; 0.0003733 0 0 0; 0.0004977 0 0 0; 0.0006221 0 0 0]  x3=[0 0 0 0; 0.0001244 0 0 0; 0.0002488 0 0 0; 0.0003733 0 0 0; 0.0004977 0 0 0; 0.0006221 0 0 0]  x4=[0 0 0 0; 0.0001244 0 0 0; 0.0002488 0 0 0; 0.0003733 0 0 0; 0.0004977 0 0 0; 0.0006221 0 0 0]  x5=0  V1=ones(3,3)  V2=ones(3,3)  I1=ones(3,3)  I2=ones(3,3)  nHarmo=1  Measurements=None
  Jägala_haruliin_CN_29978896_110000_CN_29979106_110000 : powerlib/Elements/Distributed Parameters Line  Phases=3  Frequency=60  Resistance=[0.01273 0.3864]  Inductance="[0.9337e-3  4.1264e-3]"  Capacitance=[12.74e-9 7.751e-9]  Length=27.8814  x1=[0 0 0 0; 0.0001244 0 0 0; 0.0002488 0 0 0; 0.0003733 0 0 0; 0.0004977 0 0 0; 0.0006221 0 0 0]  x2=[0 0 0 0; 0.0001244 0 0 0; 0.0002488 0 0 0; 0.0003733 0 0 0; 0.0004977 0 0 0; 0.0006221 0 0 0]  x3=[0 0 0 0; 0.0001244 0 0 0; 0.0002488 0 0 0; 0.0003733 0 0 0; 0.0004977 0 0 0; 0.0006221 0 0 0]  x4=[0 0 0 0; 0.0001244 0 0 0; 0.0002488 0 0 0; 0.0003733 0 0 0; 0.0004977 0 0 0; 0.0006221 0 0 0]  x5=0  V1=ones(3,3)  V2=ones(3,3)  I1=ones(3,3)  I2=ones(3,3)  nHarmo=1  Measurements=None
  Järvakandi_—_Valgu_110_kV_CN_35550410_110000_CN_35550412_110000 : powerlib/Elements/Distributed Parameters Line  Phases=3  Frequency=60  Resistance=[0.01273 0.3864]  Inductance="[0.9337e-3  4.1264e-3]"  Capacitance=[12.74e-9 7.751e-9]  Length=15.1095  x1=[0 0 0 0; 0.0001244 0 0 0; 0.0002488 0 0 0; 0.0003733 0 0 0; 0.0004977 0 0 0; 0.0006221 0 0 0]  x2=[0 0 0 0; 0.0001244 0 0 0; 0.0002488 0 0 0; 0.0003733 0 0 0; 0.0004977 0 0 0; 0.0006221 0 0 0]  x3=[0 0 0 0; 0.0001244 0 0 0; 0.0002488 0 0 0; 0.0003733 0 0 0; 0.0004977 0 0 0; 0.0006221 0 0 0]  x4=[0 0 0 0; 0.0001244 0 0 0; 0.0002488 0 0 0; 0.0003733 0 0 0; 0.0004977 0 0 0; 0.0006221 0 0 0]  x5=0  V1=ones(3,3)  V2=ones(3,3)  I1=ones(3,3)  I2=ones(3,3)  nHarmo=1  Measurements=None
  Järve_—_Ülemiste_110_kV_CN_34968246_110000_CN_34968248_110000 : powerlib/Elements/Distributed Parameters Line  Phases=3  Frequency=60  Resistance=[0.01273 0.3864]  Inductance="[0.9337e-3  4.1264e-3]"  Capacitance=[12.74e-9 7.751e-9]  Length=5.631  x1=[0 0 0 0; 0.0001244 0 0 0; 0.0002488 0 0 0; 0.0003733 0 0 0; 0.0004977 0 0 0; 0.0006221 0 0 0]  x2=[0 0 0 0; 0.0001244 0 0 0; 0.0002488 0 0 0; 0.0003733 0 0 0; 0.0004977 0 0 0; 0.0006221 0 0 0]  x3=[0 0 0 0; 0.0001244 0 0 0; 0.0002488 0 0 0; 0.0003733 0 0 0; 0.0004977 0 0 0; 0.0006221 0 0 0]  x4=[0 0 0 0; 0.0001244 0 0 0; 0.0002488 0 0 0; 0.0003733 0 0 0; 0.0004977 0 0 0; 0.0006221 0 0 0]  x5=0  V1=ones(3,3)  V2=ones(3,3)  I1=ones(3,3)  I2=ones(3,3)  nHarmo=1  Measurements=None
  Jõgeva_—_Põdra_110_kV_CN_263282458_110000_CN_35451774_110000 : powerlib/Elements/Distributed Parameters Line  Phases=3  Frequency=60  Resistance=[0.01273 0.3864]  Inductance="[0.9337e-3  4.1264e-3]"  Capacitance=[12.74e-9 7.751e-9]  Length=13.4748  x1=[0 0 0 0; 0.0001244 0 0 0; 0.0002488 0 0 0; 0.0003733 0 0 0; 0.0004977 0 0 0; 0.0006221 0 0 0]  x2=[0 0 0 0; 0.0001244 0 0 0; 0.0002488 0 0 0; 0.0003733 0 0 0; 0.0004977 0 0 0; 0.0006221 0 0 0]  x3=[0 0 0 0; 0.0001244 0 0 0; 0.0002488 0 0 0; 0.0003733 0 0 0; 0.0004977 0 0 0; 0.0006221 0 0 0]  x4=[0 0 0 0; 0.0001244 0 0 0; 0.0002488 0 0 0; 0.0003733 0 0 0; 0.0004977 0 0 0; 0.0006221 0 0 0]  x5=0  V1=ones(3,3)  V2=ones(3,3)  I1=ones(3,3)  I2=ones(3,3)  nHarmo=1  Measurements=None
  Kallavere_—_Viimsi_110_kV_CN_34968274_110000_CN_29979106_110000 : powerlib/Elements/Distributed Parameters Line  Phases=3  Frequency=60  Resistance=[0.01273 0.3864]  Inductance="[0.9337e-3  4.1264e-3]"  Capacitance=[12.74e-9 7.751e-9]  Length=10.8007  x1=[0 0 0 0; 0.0001244 0 0 0; 0.0002488 0 0 0; 0.0003733 0 0 0; 0.0004977 0 0 0; 0.0006221 0 0 0]  x2=[0 0 0 0; 0.0001244 0 0 0; 0.0002488 0 0 0; 0.0003733 0 0 0; 0.0004977 0 0 0; 0.0006221 0 0 0]  x3=[0 0 0 0; 0.0001244 0 0 0; 0.0002488 0 0 0; 0.0003733 0 0 0; 0.0004977 0 0 0; 0.0006221 0 0 0]  x4=[0 0 0 0; 0.0001244 0 0 0; 0.0002488 0 0 0; 0.0003733 0 0 0; 0.0004977 0 0 0; 0.0006221 0 0 0]  x5=0  V1=ones(3,3)  V2=ones(3,3)  I1=ones(3,3)  I2=ones(3,3)  nHarmo=1  Measurements=None
  Kalserbach___Kienburg_CN_85703086_110000_CN_85699549_110000 : powerlib/Elements/Distributed Parameters Line  Phases=3  Frequency=60  Resistance=[0.01273 0.3864]  Inductance="[0.9337e-3  4.1264e-3]"  Capacitance=[12.74e-9 7.751e-9]  Length=100  x1=[0 0 0 0; 0.0001244 0 0 0; 0.0002488 0 0 0; 0.0003733 0 0 0; 0.0004977 0 0 0; 0.0006221 0 0 0]  x2=[0 0 0 0; 0.0001244 0 0 0; 0.0002488 0 0 0; 0.0003733 0 0 0; 0.0004977 0 0 0; 0.0006221 0 0 0]  x3=[0 0 0 0; 0.0001244 0 0 0; 0.0002488 0 0 0; 0.0003733 0 0 0; 0.0004977 0 0 0; 0.0006221 0 0 0]  x4=[0 0 0 0; 0.0001244 0 0 0; 0.0002488 0 0 0; 0.0003733 0 0 0; 0.0004977 0 0 0; 0.0006221 0 0 0]  x5=0  V1=ones(3,3)  V2=ones(3,3)  I1=ones(3,3)  I2=ones(3,3)  nHarmo=1  Measurements=None
  Kanepi_—_Võru_110_kV_CN_35445333_110000_CN_35445334_110000 : powerlib/Elements/Distributed Parameters Line  Phases=3  Frequency=60  Resistance=[0.01273 0.3864]  Inductance="[0.9337e-3  4.1264e-3]"  Capacitance=[12.74e-9 7.751e-9]  Length=24.3209  x1=[0 0 0 0; 0.0001244 0 0 0; 0.0002488 0 0 0; 0.0003733 0 0 0; 0.0004977 0 0 0; 0.0006221 0 0 0]  x2=[0 0 0 0; 0.0001244 0 0 0; 0.0002488 0 0 0; 0.0003733 0 0 0; 0.0004977 0 0 0; 0.0006221 0 0 0]  x3=[0 0 0 0; 0.0001244 0 0 0; 0.0002488 0 0 0; 0.0003733 0 0 0; 0.0004977 0 0 0; 0.0006221 0 0 0]  x4=[0 0 0 0; 0.0001244 0 0 0; 0.0002488 0 0 0; 0.0003733 0 0 0; 0.0004977 0 0 0; 0.0006221 0 0 0]  x5=0  V1=ones(3,3)  V2=ones(3,3)  I1=ones(3,3)  I2=ones(3,3)  nHarmo=1  Measurements=None
  Kehtna_—_Järvakandi_110_kV_CN_35550410_110000_CN_35550415_110000 : powerlib/Elements/Distributed Parameters Line  Phases=3  Frequency=60  Resistance=[0.01273 0.3864]  Inductance="[0.9337e-3  4.1264e-3]"  Capacitance=[12.74e-9 7.751e-9]  Length=14.7144  x1=[0 0 0 0; 0.0001244 0 0 0; 0.0002488 0 0 0; 0.0003733 0 0 0; 0.0004977 0 0 0; 0.0006221 0 0 0]  x2=[0 0 0 0; 0.0001244 0 0 0; 0.0002488 0 0 0; 0.0003733 0 0 0; 0.0004977 0 0 0; 0.0006221 0 0 0]  x3=[0 0 0 0; 0.0001244 0 0 0; 0.0002488 0 0 0; 0.0003733 0 0 0; 0.0004977 0 0 0; 0.0006221 0 0 0]  x4=[0 0 0 0; 0.0001244 0 0 0; 0.0002488 0 0 0; 0.0003733 0 0 0; 0.0004977 0 0 0; 0.0006221 0 0 0]  x5=0  V1=ones(3,3)  V2=ones(3,3)  I1=ones(3,3)  I2=ones(3,3)  nHarmo=1  Measurements=None
  Keila_—_Paldiski_110_kV_CN_35550404_110000_CN_262229346_110000 : powerlib/Elements/Distributed Parameters Line  Phases=3  Frequency=60  Resistance=[0.01273 0.3864]  Inductance="[0.9337e-3  4.1264e-3]"  Capacitance=[12.74e-9 7.751e-9]  Length=22.3573  x1=[0 0 0 0; 0.0001244 0 0 0; 0.0002488 0 0 0; 0.0003733 0 0 0; 0.0004977 0 0 0; 0.0006221 0 0 0]  x2=[0 0 0 0; 0.0001244 0 0 0; 0.0002488 0 0 0; 0.0003733 0 0 0; 0.0004977 0 0 0; 0.0006221 0 0 0]  x3=[0 0 0 0; 0.0001244 0 0 0; 0.0002488 0 0 0; 0.0003733 0 0 0; 0.0004977 0 0 0; 0.0006221 0 0 0]  x4=[0 0 0 0; 0.0001244 0 0 0; 0.0002488 0 0 0; 0.0003733 0 0 0; 0.0004977 0 0 0; 0.0006221 0 0 0]  x5=0  V1=ones(3,3)  V2=ones(3,3)  I1=ones(3,3)  I2=ones(3,3)  nHarmo=1  Measurements=None
  Keila_—_Rummu_110_kV_CN_262229346_110000_CN_34988486_110000 : powerlib/Elements/Distributed Parameters Line  Phases=3  Frequency=60  Resistance=[0.01273 0.3864]  Inductance="[0.9337e-3  4.1264e-3]"  Capacitance=[12.74e-9 7.751e-9]  Length=28.7268  x1=[0 0 0 0; 0.0001244 0 0 0; 0.0002488 0 0 0; 0.0003733 0 0 0; 0.0004977 0 0 0; 0.0006221 0 0 0]  x2=[0 0 0 0; 0.0001244 0 0 0; 0.0002488 0 0 0; 0.0003733 0 0 0; 0.0004977 0 0 0; 0.0006221 0 0 0]  x3=[0 0 0 0; 0.0001244 0 0 0; 0.0002488 0 0 0; 0.0003733 0 0 0; 0.0004977 0 0 0; 0.0006221 0 0 0]  x4=[0 0 0 0; 0.0001244 0 0 0; 0.0002488 0 0 0; 0.0003733 0 0 0; 0.0004977 0 0 0; 0.0006221 0 0 0]  x5=0  V1=ones(3,3)  V2=ones(3,3)  I1=ones(3,3)  I2=ones(3,3)  nHarmo=1  Measurements=None
  Kiikla_—_Alutaguse_110_kV_CN_35367472_110000_CN_263282454_110000 : powerlib/Elements/Distributed Parameters Line  Phases=3  Frequency=60  Resistance=[0.01273 0.3864]  Inductance="[0.9337e-3  4.1264e-3]"  Capacitance=[12.74e-9 7.751e-9]  Length=19.0986  x1=[0 0 0 0; 0.0001244 0 0 0; 0.0002488 0 0 0; 0.0003733 0 0 0; 0.0004977 0 0 0; 0.0006221 0 0 0]  x2=[0 0 0 0; 0.0001244 0 0 0; 0.0002488 0 0 0; 0.0003733 0 0 0; 0.0004977 0 0 0; 0.0006221 0 0 0]  x3=[0 0 0 0; 0.0001244 0 0 0; 0.0002488 0 0 0; 0.0003733 0 0 0; 0.0004977 0 0 0; 0.0006221 0 0 0]  x4=[0 0 0 0; 0.0001244 0 0 0; 0.0002488 0 0 0; 0.0003733 0 0 0; 0.0004977 0 0 0; 0.0006221 0 0 0]  x5=0  V1=ones(3,3)  V2=ones(3,3)  I1=ones(3,3)  I2=ones(3,3)  nHarmo=1  Measurements=None
  Kiikla_—_Alutaguse_110_kV_CN_35367472_110000_CN_34920675_110000 : powerlib/Elements/Distributed Parameters Line  Phases=3  Frequency=60  Resistance=[0.01273 0.3864]  Inductance="[0.9337e-3  4.1264e-3]"  Capacitance=[12.74e-9 7.751e-9]  Length=35.4442  x1=[0 0 0 0; 0.0001244 0 0 0; 0.0002488 0 0 0; 0.0003733 0 0 0; 0.0004977 0 0 0; 0.0006221 0 0 0]  x2=[0 0 0 0; 0.0001244 0 0 0; 0.0002488 0 0 0; 0.0003733 0 0 0; 0.0004977 0 0 0; 0.0006221 0 0 0]  x3=[0 0 0 0; 0.0001244 0 0 0; 0.0002488 0 0 0; 0.0003733 0 0 0; 0.0004977 0 0 0; 0.0006221 0 0 0]  x4=[0 0 0 0; 0.0001244 0 0 0; 0.0002488 0 0 0; 0.0003733 0 0 0; 0.0004977 0 0 0; 0.0006221 0 0 0]  x5=0  V1=ones(3,3)  V2=ones(3,3)  I1=ones(3,3)  I2=ones(3,3)  nHarmo=1  Measurements=None
  Kiisa_—_Ellamaa_CN_34935436_110000_CN_34988502_110000 : powerlib/Elements/Distributed Parameters Line  Phases=3  Frequency=60  Resistance=[0.01273 0.3864]  Inductance="[0.9337e-3  4.1264e-3]"  Capacitance=[12.74e-9 7.751e-9]  Length=52.9108  x1=[0 0 0 0; 0.0001244 0 0 0; 0.0002488 0 0 0; 0.0003733 0 0 0; 0.0004977 0 0 0; 0.0006221 0 0 0]  x2=[0 0 0 0; 0.0001244 0 0 0; 0.0002488 0 0 0; 0.0003733 0 0 0; 0.0004977 0 0 0; 0.0006221 0 0 0]  x3=[0 0 0 0; 0.0001244 0 0 0; 0.0002488 0 0 0; 0.0003733 0 0 0; 0.0004977 0 0 0; 0.0006221 0 0 0]  x4=[0 0 0 0; 0.0001244 0 0 0; 0.0002488 0 0 0; 0.0003733 0 0 0; 0.0004977 0 0 0; 0.0006221 0 0 0]  x5=0  V1=ones(3,3)  V2=ones(3,3)  I1=ones(3,3)  I2=ones(3,3)  nHarmo=1  Measurements=None
  Kiisa_—_Ellamaa_CN_34935436_110000_CN_34988535_110000 : powerlib/Elements/Distributed Parameters Line  Phases=3  Frequency=60  Resistance=[0.01273 0.3864]  Inductance="[0.9337e-3  4.1264e-3]"  Capacitance=[12.74e-9 7.751e-9]  Length=38.568  x1=[0 0 0 0; 0.0001244 0 0 0; 0.0002488 0 0 0; 0.0003733 0 0 0; 0.0004977 0 0 0; 0.0006221 0 0 0]  x2=[0 0 0 0; 0.0001244 0 0 0; 0.0002488 0 0 0; 0.0003733 0 0 0; 0.0004977 0 0 0; 0.0006221 0 0 0]  x3=[0 0 0 0; 0.0001244 0 0 0; 0.0002488 0 0 0; 0.0003733 0 0 0; 0.0004977 0 0 0; 0.0006221 0 0 0]  x4=[0 0 0 0; 0.0001244 0 0 0; 0.0002488 0 0 0; 0.0003733 0 0 0; 0.0004977 0 0 0; 0.0006221 0 0 0]  x5=0  V1=ones(3,3)  V2=ones(3,3)  I1=ones(3,3)  I2=ones(3,3)  nHarmo=1  Measurements=None
  Kiisa_—_Ellamaa_CN_34935436_110000_CN_35379710_110000 : powerlib/Elements/Distributed Parameters Line  Phases=3  Frequency=60  Resistance=[0.01273 0.3864]  Inductance="[0.9337e-3  4.1264e-3]"  Capacitance=[12.74e-9 7.751e-9]  Length=15.6846  x1=[0 0 0 0; 0.0001244 0 0 0; 0.0002488 0 0 0; 0.0003733 0 0 0; 0.0004977 0 0 0; 0.0006221 0 0 0]  x2=[0 0 0 0; 0.0001244 0 0 0; 0.0002488 0 0 0; 0.0003733 0 0 0; 0.0004977 0 0 0; 0.0006221 0 0 0]  x3=[0 0 0 0; 0.0001244 0 0 0; 0.0002488 0 0 0; 0.0003733 0 0 0; 0.0004977 0 0 0; 0.0006221 0 0 0]  x4=[0 0 0 0; 0.0001244 0 0 0; 0.0002488 0 0 0; 0.0003733 0 0 0; 0.0004977 0 0 0; 0.0006221 0 0 0]  x5=0  V1=ones(3,3)  V2=ones(3,3)  I1=ones(3,3)  I2=ones(3,3)  nHarmo=1  Measurements=None
  Kiisa_—_Järve_110_kV_CN_34935436_110000_CN_34968246_110000 : powerlib/Elements/Distributed Parameters Line  Phases=3  Frequency=60  Resistance=[0.01273 0.3864]  Inductance="[0.9337e-3  4.1264e-3]"  Capacitance=[12.74e-9 7.751e-9]  Length=24.4594  x1=[0 0 0 0; 0.0001244 0 0 0; 0.0002488 0 0 0; 0.0003733 0 0 0; 0.0004977 0 0 0; 0.0006221 0 0 0]  x2=[0 0 0 0; 0.0001244 0 0 0; 0.0002488 0 0 0; 0.0003733 0 0 0; 0.0004977 0 0 0; 0.0006221 0 0 0]  x3=[0 0 0 0; 0.0001244 0 0 0; 0.0002488 0 0 0; 0.0003733 0 0 0; 0.0004977 0 0 0; 0.0006221 0 0 0]  x4=[0 0 0 0; 0.0001244 0 0 0; 0.0002488 0 0 0; 0.0003733 0 0 0; 0.0004977 0 0 0; 0.0006221 0 0 0]  x5=0  V1=ones(3,3)  V2=ones(3,3)  I1=ones(3,3)  I2=ones(3,3)  nHarmo=1  Measurements=None
  Kiisa_—_Järve_110_kV_CN_34935436_110000_CN_34968285_110000 : powerlib/Elements/Distributed Parameters Line  Phases=3  Frequency=60  Resistance=[0.01273 0.3864]  Inductance="[0.9337e-3  4.1264e-3]"  Capacitance=[12.74e-9 7.751e-9]  Length=22.7854  x1=[0 0 0 0; 0.0001244 0 0 0; 0.0002488 0 0 0; 0.0003733 0 0 0; 0.0004977 0 0 0; 0.0006221 0 0 0]  x2=[0 0 0 0; 0.0001244 0 0 0; 0.0002488 0 0 0; 0.0003733 0 0 0; 0.0004977 0 0 0; 0.0006221 0 0 0]  x3=[0 0 0 0; 0.0001244 0 0 0; 0.0002488 0 0 0; 0.0003733 0 0 0; 0.0004977 0 0 0; 0.0006221 0 0 0]  x4=[0 0 0 0; 0.0001244 0 0 0; 0.0002488 0 0 0; 0.0003733 0 0 0; 0.0004977 0 0 0; 0.0006221 0 0 0]  x5=0  V1=ones(3,3)  V2=ones(3,3)  I1=ones(3,3)  I2=ones(3,3)  nHarmo=1  Measurements=None
  Kiisa_—_Keila_110_kV_CN_34935436_110000_CN_262229346_110000 : powerlib/Elements/Distributed Parameters Line  Phases=3  Frequency=60  Resistance=[0.01273 0.3864]  Inductance="[0.9337e-3  4.1264e-3]"  Capacitance=[12.74e-9 7.751e-9]  Length=18.4608  x1=[0 0 0 0; 0.0001244 0 0 0; 0.0002488 0 0 0; 0.0003733 0 0 0; 0.0004977 0 0 0; 0.0006221 0 0 0]  x2=[0 0 0 0; 0.0001244 0 0 0; 0.0002488 0 0 0; 0.0003733 0 0 0; 0.0004977 0 0 0; 0.0006221 0 0 0]  x3=[0 0 0 0; 0.0001244 0 0 0; 0.0002488 0 0 0; 0.0003733 0 0 0; 0.0004977 0 0 0; 0.0006221 0 0 0]  x4=[0 0 0 0; 0.0001244 0 0 0; 0.0002488 0 0 0; 0.0003733 0 0 0; 0.0004977 0 0 0; 0.0006221 0 0 0]  x5=0  V1=ones(3,3)  V2=ones(3,3)  I1=ones(3,3)  I2=ones(3,3)  nHarmo=1  Measurements=None
  Kiisa_—_Laagri_110_kV_CN_34935436_110000_CN_34935452_110000 : powerlib/Elements/Distributed Parameters Line  Phases=3  Frequency=60  Resistance=[0.01273 0.3864]  Inductance="[0.9337e-3  4.1264e-3]"  Capacitance=[12.74e-9 7.751e-9]  Length=14.6531  x1=[0 0 0 0; 0.0001244 0 0 0; 0.0002488 0 0 0; 0.0003733 0 0 0; 0.0004977 0 0 0; 0.0006221 0 0 0]  x2=[0 0 0 0; 0.0001244 0 0 0; 0.0002488 0 0 0; 0.0003733 0 0 0; 0.0004977 0 0 0; 0.0006221 0 0 0]  x3=[0 0 0 0; 0.0001244 0 0 0; 0.0002488 0 0 0; 0.0003733 0 0 0; 0.0004977 0 0 0; 0.0006221 0 0 0]  x4=[0 0 0 0; 0.0001244 0 0 0; 0.0002488 0 0 0; 0.0003733 0 0 0; 0.0004977 0 0 0; 0.0006221 0 0 0]  x5=0  V1=ones(3,3)  V2=ones(3,3)  I1=ones(3,3)  I2=ones(3,3)  nHarmo=1  Measurements=None
  Kiisa_—_Laagri_110_kV_CN_34935436_110000_CN_34988471_110000 : powerlib/Elements/Distributed Parameters Line  Phases=3  Frequency=60  Resistance=[0.01273 0.3864]  Inductance="[0.9337e-3  4.1264e-3]"  Capacitance=[12.74e-9 7.751e-9]  Length=12.5852  x1=[0 0 0 0; 0.0001244 0 0 0; 0.0002488 0 0 0; 0.0003733 0 0 0; 0.0004977 0 0 0; 0.0006221 0 0 0]  x2=[0 0 0 0; 0.0001244 0 0 0; 0.0002488 0 0 0; 0.0003733 0 0 0; 0.0004977 0 0 0; 0.0006221 0 0 0]  x3=[0 0 0 0; 0.0001244 0 0 0; 0.0002488 0 0 0; 0.0003733 0 0 0; 0.0004977 0 0 0; 0.0006221 0 0 0]  x4=[0 0 0 0; 0.0001244 0 0 0; 0.0002488 0 0 0; 0.0003733 0 0 0; 0.0004977 0 0 0; 0.0006221 0 0 0]  x5=0  V1=ones(3,3)  V2=ones(3,3)  I1=ones(3,3)  I2=ones(3,3)  nHarmo=1  Measurements=None
  Kirchdorf___Kremsmünster_CN_95025696_110000_CN_50899766_110000 : powerlib/Elements/Distributed Parameters Line  Phases=3  Frequency=60  Resistance=[0.01273 0.3864]  Inductance="[0.9337e-3  4.1264e-3]"  Capacitance=[12.74e-9 7.751e-9]  Length=100  x1=[0 0 0 0; 0.0001244 0 0 0; 0.0002488 0 0 0; 0.0003733 0 0 0; 0.0004977 0 0 0; 0.0006221 0 0 0]  x2=[0 0 0 0; 0.0001244 0 0 0; 0.0002488 0 0 0; 0.0003733 0 0 0; 0.0004977 0 0 0; 0.0006221 0 0 0]  x3=[0 0 0 0; 0.0001244 0 0 0; 0.0002488 0 0 0; 0.0003733 0 0 0; 0.0004977 0 0 0; 0.0006221 0 0 0]  x4=[0 0 0 0; 0.0001244 0 0 0; 0.0002488 0 0 0; 0.0003733 0 0 0; 0.0004977 0 0 0; 0.0006221 0 0 0]  x5=0  V1=ones(3,3)  V2=ones(3,3)  I1=ones(3,3)  I2=ones(3,3)  nHarmo=1  Measurements=None
  Kopli_—_Paljassaare_110_kV_CN_34968238_110000_CN_34968239_110000 : powerlib/Elements/Distributed Parameters Line  Phases=3  Frequency=60  Resistance=[0.01273 0.3864]  Inductance="[0.9337e-3  4.1264e-3]"  Capacitance=[12.74e-9 7.751e-9]  Length=2.4403  x1=[0 0 0 0; 0.0001244 0 0 0; 0.0002488 0 0 0; 0.0003733 0 0 0; 0.0004977 0 0 0; 0.0006221 0 0 0]  x2=[0 0 0 0; 0.0001244 0 0 0; 0.0002488 0 0 0; 0.0003733 0 0 0; 0.0004977 0 0 0; 0.0006221 0 0 0]  x3=[0 0 0 0; 0.0001244 0 0 0; 0.0002488 0 0 0; 0.0003733 0 0 0; 0.0004977 0 0 0; 0.0006221 0 0 0]  x4=[0 0 0 0; 0.0001244 0 0 0; 0.0002488 0 0 0; 0.0003733 0 0 0; 0.0004977 0 0 0; 0.0006221 0 0 0]  x5=0  V1=ones(3,3)  V2=ones(3,3)  I1=ones(3,3)  I2=ones(3,3)  nHarmo=1  Measurements=None
  Kopli_—_Paljassaare_110_kV_CN_34968238_110000_CN_85487602_110000 : powerlib/Elements/Distributed Parameters Line  Phases=3  Frequency=60  Resistance=[0.01273 0.3864]  Inductance="[0.9337e-3  4.1264e-3]"  Capacitance=[12.74e-9 7.751e-9]  Length=3.9414  x1=[0 0 0 0; 0.0001244 0 0 0; 0.0002488 0 0 0; 0.0003733 0 0 0; 0.0004977 0 0 0; 0.0006221 0 0 0]  x2=[0 0 0 0; 0.0001244 0 0 0; 0.0002488 0 0 0; 0.0003733 0 0 0; 0.0004977 0 0 0; 0.0006221 0 0 0]  x3=[0 0 0 0; 0.0001244 0 0 0; 0.0002488 0 0 0; 0.0003733 0 0 0; 0.0004977 0 0 0; 0.0006221 0 0 0]  x4=[0 0 0 0; 0.0001244 0 0 0; 0.0002488 0 0 0; 0.0003733 0 0 0; 0.0004977 0 0 0; 0.0006221 0 0 0]  x5=0  V1=ones(3,3)  V2=ones(3,3)  I1=ones(3,3)  I2=ones(3,3)  nHarmo=1  Measurements=None
  Kopli_—_Paljassaare_110_kV_CN_34968238_110000_CN_99350295_110000 : powerlib/Elements/Distributed Parameters Line  Phases=3  Frequency=60  Resistance=[0.01273 0.3864]  Inductance="[0.9337e-3  4.1264e-3]"  Capacitance=[12.74e-9 7.751e-9]  Length=4.6891  x1=[0 0 0 0; 0.0001244 0 0 0; 0.0002488 0 0 0; 0.0003733 0 0 0; 0.0004977 0 0 0; 0.0006221 0 0 0]  x2=[0 0 0 0; 0.0001244 0 0 0; 0.0002488 0 0 0; 0.0003733 0 0 0; 0.0004977 0 0 0; 0.0006221 0 0 0]  x3=[0 0 0 0; 0.0001244 0 0 0; 0.0002488 0 0 0; 0.0003733 0 0 0; 0.0004977 0 0 0; 0.0006221 0 0 0]  x4=[0 0 0 0; 0.0001244 0 0 0; 0.0002488 0 0 0; 0.0003733 0 0 0; 0.0004977 0 0 0; 0.0006221 0 0 0]  x5=0  V1=ones(3,3)  V2=ones(3,3)  I1=ones(3,3)  I2=ones(3,3)  nHarmo=1  Measurements=None
  Kuusalu_—_Kolga_110_kV_CN_35384083_110000_CN_35555166_110000 : powerlib/Elements/Distributed Parameters Line  Phases=3  Frequency=60  Resistance=[0.01273 0.3864]  Inductance="[0.9337e-3  4.1264e-3]"  Capacitance=[12.74e-9 7.751e-9]  Length=28.4298  x1=[0 0 0 0; 0.0001244 0 0 0; 0.0002488 0 0 0; 0.0003733 0 0 0; 0.0004977 0 0 0; 0.0006221 0 0 0]  x2=[0 0 0 0; 0.0001244 0 0 0; 0.0002488 0 0 0; 0.0003733 0 0 0; 0.0004977 0 0 0; 0.0006221 0 0 0]  x3=[0 0 0 0; 0.0001244 0 0 0; 0.0002488 0 0 0; 0.0003733 0 0 0; 0.0004977 0 0 0; 0.0006221 0 0 0]  x4=[0 0 0 0; 0.0001244 0 0 0; 0.0002488 0 0 0; 0.0003733 0 0 0; 0.0004977 0 0 0; 0.0006221 0 0 0]  x5=0  V1=ones(3,3)  V2=ones(3,3)  I1=ones(3,3)  I2=ones(3,3)  nHarmo=1  Measurements=None
  Kuusalu_—_Kolga_110_kV_CN_35384083_110000_CN_35555171_110000 : powerlib/Elements/Distributed Parameters Line  Phases=3  Frequency=60  Resistance=[0.01273 0.3864]  Inductance="[0.9337e-3  4.1264e-3]"  Capacitance=[12.74e-9 7.751e-9]  Length=14.1288  x1=[0 0 0 0; 0.0001244 0 0 0; 0.0002488 0 0 0; 0.0003733 0 0 0; 0.0004977 0 0 0; 0.0006221 0 0 0]  x2=[0 0 0 0; 0.0001244 0 0 0; 0.0002488 0 0 0; 0.0003733 0 0 0; 0.0004977 0 0 0; 0.0006221 0 0 0]  x3=[0 0 0 0; 0.0001244 0 0 0; 0.0002488 0 0 0; 0.0003733 0 0 0; 0.0004977 0 0 0; 0.0006221 0 0 0]  x4=[0 0 0 0; 0.0001244 0 0 0; 0.0002488 0 0 0; 0.0003733 0 0 0; 0.0004977 0 0 0; 0.0006221 0 0 0]  x5=0  V1=ones(3,3)  V2=ones(3,3)  I1=ones(3,3)  I2=ones(3,3)  nHarmo=1  Measurements=None
  Kuuste_—_Põlva_110_kV_CN_35445343_110000_CN_35445346_110000 : powerlib/Elements/Distributed Parameters Line  Phases=3  Frequency=60  Resistance=[0.01273 0.3864]  Inductance="[0.9337e-3  4.1264e-3]"  Capacitance=[12.74e-9 7.751e-9]  Length=30.4992  x1=[0 0 0 0; 0.0001244 0 0 0; 0.0002488 0 0 0; 0.0003733 0 0 0; 0.0004977 0 0 0; 0.0006221 0 0 0]  x2=[0 0 0 0; 0.0001244 0 0 0; 0.0002488 0 0 0; 0.0003733 0 0 0; 0.0004977 0 0 0; 0.0006221 0 0 0]  x3=[0 0 0 0; 0.0001244 0 0 0; 0.0002488 0 0 0; 0.0003733 0 0 0; 0.0004977 0 0 0; 0.0006221 0 0 0]  x4=[0 0 0 0; 0.0001244 0 0 0; 0.0002488 0 0 0; 0.0003733 0 0 0; 0.0004977 0 0 0; 0.0006221 0 0 0]  x5=0  V1=ones(3,3)  V2=ones(3,3)  I1=ones(3,3)  I2=ones(3,3)  nHarmo=1  Measurements=None
  L_{19881598,23709119,23899163,24253250,24768685,24830381,25539194,25539735,25541069,26209260,26524546,26644088,27673934,27719234,27763479,27795895,27797285,28100536,28447213,28449168,28504203,28596524,28766884,29563097,30042006,30076588,30222212,30244554,30840698,30842675,31659735,32293834,32465765,32489430,32493406,32496352,32674497,32809456,32821660,33003040,33003245,33004923,33041399,33058565,33064531,33066376,33066588,33077861,33463751,33482741,33624954,33631653,33631764,33632720,33682610,33685690,33750614,33840061,34258314,35034309,35953425,37232839,37337545,38821658,38868243,39271873,40641599,40917240,42306133,42330333,42352281,45544115,46724466,47001881,47002504,50650855,50729129,50899766,52954814,59531071,60222001,61108302,68193799,69859724,70497801,79122729,80855358,81216242,81540198,81611149,81611545,81684898,82201785,83202471,83424897,83500268,83529203,83643796,83730525,83740188,83740194,83742775,83742801,83803297,83805040,83805050,83823298,83823666,83831570,83892409,83892416,83892438,83896165,83947318,84006669,84014726,84014731,84622128,84789829,84880034,84880037,85387750,85387757,85389628,85391848,85405514,85471947,85489932,85489961,85586883,85586885,85620021,85639941,85699520,85699549,85703086,86119428,86119456,86119509,86166232,86258560,86321299,86385664,86415777,86499892,86693139,86869607,87131144,87246307,87264584,87365703,87372613,87526678,87702041,88180087,88285465,88381334..88381335,88381528,88381707,88680218,88684218,88802394,88844735,89043963,89451551,89555133,89985993,90051319,90060333,90073458,90431884,90498611,90675524,90683456,90866864,90904770,91013052,91067944,91071153,91071159,91236151,91250729,91579706,92220396,92220415,92340887,92686645,92870633,92873353,92938764,93044006,93187006,93206012,93206014,93215114,93331921,93370554,93483694,93982415,94098463,94149189,94159103,94232595,94239516,94372577,94406313,94452460,94505943,94514064,94552553,94790504,95003268,95024146,95025696,95025698,95094291,95096550,95124819,95194594,95211290,95227815,95289063,95297285,95456147,95640323,95642941,95644443,95743675,95783711,95790224,95812161,95812231,95828347,95828351,95837656,95837658,95843031,95848249,95860758,95972388,95975628,95978048,96168202,96176843,96187654,96193588,96210904,96323087,96346322,96355233,96358427,96596880,96600181,96616299,96657240,96689254,96702435,96734998,96826419,96855956,96959342,96970398,96989592,96998954,97094288,97094291,97094293..97094294,97144374,97207142,97217194,97218204,97224226,97224229,97226005,97264200,97348720,97379897,97384262,97392181,97402227,97586384,97870174,97989146,98007002,98245350,98249243,98290225,98308316,98371047,98383732,98635106..98635107,99730272,99731682,99745003,99755951,99761298..99761299,99791175,99841738,99877186,100275873,100404264,100409307,100478972,100602290,100619811,100868499,101976746,101997887,102151229,102572506,102601926,102699327,102767009,103387969,103394555,103401933,103774165,103800082,105065132,105080874,105431455,106525523,106530735,107117959,107248400,107296187,107322714,108120142,110540215,112481895,113597106,114715432,114873634,116018035,118060597,118091356,118098478,118104933,118132395,118927581,118938988,119489306,119687430,120014259,120014261,121265317,121293775,122351223,122454383,122462450,122592181,122669259,122763233,122849865,122942230,123098511,123115522,123121995,123173012,123174725,123384821,123444716,123689023,124415043,126218483,128132750,128185694,128191035,128196020,128225177,128228754,128503723,128734659,128963182,129009559,129643773,130797001,132457784,132468928,133669362,134565164,135260775,135931468,136384702,137946515,138407044,141871546,141875426,142188184..142188185,143024167,144202272,145583866,146122262,146978108,147563007..147563008,151942483..151942484,152299025,153783851,156818117..156818118,156973414,162826525,162834614,166614156,167350226,169304139,169361887,171066516,171116600,171672621,174466040,174474431,174531795,180468540,185860195,186110657,193604569,194940326,195015816,205801468,206394519,210191809,210505516,211095612,219909160..219909161,228092022,233040476,235546807,257384535,259327225,288347513,318616912,324055876,328978916,342158235,362660200,365493403,376356832,404737810} (447 alike) : powerlib/Elements/Three-Phase Series RLC Load  LConnTagsString=A|B|C  Configuration=Y (grounded)  NominalVoltage=1000  NominalFrequency=60  ActivePower=10e3  InductivePower=100  CapacitivePower=100  Measurements=None  LoadType=constant Z
  L_{29595798,29978896,29979106,30222062,30228363,34682059,34682089,34685113,34882447,34903268,34903294,34920675,34920683,34920691,34920699,34920702,34920713,34935436,34935452,34968224,34968238..34968239,34968246,34968248,34968251,34968269..34968270,34968274,34968276,34968285,34988471,34988480,34988486,34988495,34988502,34988518,34988522,34988525,34988527,34988531,34988535,35022081..35022082,35022087,35022089,35022100,35343343,35343349..35343350,35343353,35367472,35367480..35367481,35367491,35379710,35379726,35384064,35384083,35394600,35420117,35420119,35445333..35445335,35445340,35445343,35445346,35445348,35445361,35450869,35450872,35450875,35450914,35450919..35450920,35450930,35450940,35451763,35451772,35451774,35451776,35550404,35550410,35550412,35550415,35555161,35555163,35555165..35555166,35555171,35555173,35555175..35555176,35594687..35594689,35594697,35594708,35594719,35594731,35594741,36977398,72668114,85487602,94121285,99350295,99369449,101153487,101177924,139400061,180118919,182242759,182774903,204914596,205980356,262229346,262457166,262755193,263043288,263235177,263253461,263282453..263282454,263282458,263962720,264287766,290177759,321829090} (128 alike) : powerlib/Elements/Three-Phase Series RLC Load  LConnTagsString=A|B|C  Configuration=Y (grounded)  NominalVoltage=110000  NominalFrequency=60  ActivePower=100000  InductivePower=100  CapacitivePower=100  Measurements=None  LoadType=constant Z
  L_34685101 : powerlib/Elements/Three-Phase Series RLC Load  LConnTagsString=A|B|C  Configuration=Y (grounded)  NominalVoltage=330000  NominalFrequency=60  ActivePower=100000  InductivePower=100  CapacitivePower=100  Measurements=None  LoadType=constant Z
  Laa___Poysdorf_CN_80855358_110000_CN_96193588_110000 : powerlib/Elements/Distributed Parameters Line  Phases=3  Frequency=60  Resistance=[0.01273 0.3864]  Inductance="[0.9337e-3  4.1264e-3]"  Capacitance=[12.74e-9 7.751e-9]  Length=100  x1=[0 0 0 0; 0.0001244 0 0 0; 0.0002488 0 0 0; 0.0003733 0 0 0; 0.0004977 0 0 0; 0.0006221 0 0 0]  x2=[0 0 0 0; 0.0001244 0 0 0; 0.0002488 0 0 0; 0.0003733 0 0 0; 0.0004977 0 0 0; 0.0006221 0 0 0]  x3=[0 0 0 0; 0.0001244 0 0 0; 0.0002488 0 0 0; 0.0003733 0 0 0; 0.0004977 0 0 0; 0.0006221 0 0 0]  x4=[0 0 0 0; 0.0001244 0 0 0; 0.0002488 0 0 0; 0.0003733 0 0 0; 0.0004977 0 0 0; 0.0006221 0 0 0]  x5=0  V1=ones(3,3)  V2=ones(3,3)  I1=ones(3,3)  I2=ones(3,3)  nHarmo=1  Measurements=None
  Lambach___Puchberg_CN_37232839_110000_CN_118132395_110000 : powerlib/Elements/Distributed Parameters Line  Phases=3  Frequency=60  Resistance=[0.01273 0.3864]  Inductance="[0.9337e-3  4.1264e-3]"  Capacitance=[12.74e-9 7.751e-9]  Length=100  x1=[0 0 0 0; 0.0001244 0 0 0; 0.0002488 0 0 0; 0.0003733 0 0 0; 0.0004977 0 0 0; 0.0006221 0 0 0]  x2=[0 0 0 0; 0.0001244 0 0 0; 0.0002488 0 0 0; 0.0003733 0 0 0; 0.0004977 0 0 0; 0.0006221 0 0 0]  x3=[0 0 0 0; 0.0001244 0 0 0; 0.0002488 0 0 0; 0.0003733 0 0 0; 0.0004977 0 0 0; 0.0006221 0 0 0]  x4=[0 0 0 0; 0.0001244 0 0 0; 0.0002488 0 0 0; 0.0003733 0 0 0; 0.0004977 0 0 0; 0.0006221 0 0 0]  x5=0  V1=ones(3,3)  V2=ones(3,3)  I1=ones(3,3)  I2=ones(3,3)  nHarmo=1  Measurements=None
  Landskron___Lieserhofen;Radenthein___Lieserhofen_CN_83892438_110000_CN_84014731_110000 : powerlib/Elements/Distributed Parameters Line  Phases=3  Frequency=60  Resistance=[0.01273 0.3864]  Inductance="[0.9337e-3  4.1264e-3]"  Capacitance=[12.74e-9 7.751e-9]  Length=100  x1=[0 0 0 0; 0.0001244 0 0 0; 0.0002488 0 0 0; 0.0003733 0 0 0; 0.0004977 0 0 0; 0.0006221 0 0 0]  x2=[0 0 0 0; 0.0001244 0 0 0; 0.0002488 0 0 0; 0.0003733 0 0 0; 0.0004977 0 0 0; 0.0006221 0 0 0]  x3=[0 0 0 0; 0.0001244 0 0 0; 0.0002488 0 0 0; 0.0003733 0 0 0; 0.0004977 0 0 0; 0.0006221 0 0 0]  x4=[0 0 0 0; 0.0001244 0 0 0; 0.0002488 0 0 0; 0.0003733 0 0 0; 0.0004977 0 0 0; 0.0006221 0 0 0]  x5=0  V1=ones(3,3)  V2=ones(3,3)  I1=ones(3,3)  I2=ones(3,3)  nHarmo=1  Measurements=None
  Landskron___Lieserhofen;Radenthein___Lieserhofen_CN_83892438_110000_CN_87131144_110000 : powerlib/Elements/Distributed Parameters Line  Phases=3  Frequency=60  Resistance=[0.01273 0.3864]  Inductance="[0.9337e-3  4.1264e-3]"  Capacitance=[12.74e-9 7.751e-9]  Length=100  x1=[0 0 0 0; 0.0001244 0 0 0; 0.0002488 0 0 0; 0.0003733 0 0 0; 0.0004977 0 0 0; 0.0006221 0 0 0]  x2=[0 0 0 0; 0.0001244 0 0 0; 0.0002488 0 0 0; 0.0003733 0 0 0; 0.0004977 0 0 0; 0.0006221 0 0 0]  x3=[0 0 0 0; 0.0001244 0 0 0; 0.0002488 0 0 0; 0.0003733 0 0 0; 0.0004977 0 0 0; 0.0006221 0 0 0]  x4=[0 0 0 0; 0.0001244 0 0 0; 0.0002488 0 0 0; 0.0003733 0 0 0; 0.0004977 0 0 0; 0.0006221 0 0 0]  x5=0  V1=ones(3,3)  V2=ones(3,3)  I1=ones(3,3)  I2=ones(3,3)  nHarmo=1  Measurements=None
  Lasnamäe_—_Ülemiste_110_kV_CN_34968248_110000_CN_34968269_110000 : powerlib/Elements/Distributed Parameters Line  Phases=3  Frequency=60  Resistance=[0.01273 0.3864]  Inductance="[0.9337e-3  4.1264e-3]"  Capacitance=[12.74e-9 7.751e-9]  Length=3.1174  x1=[0 0 0 0; 0.0001244 0 0 0; 0.0002488 0 0 0; 0.0003733 0 0 0; 0.0004977 0 0 0; 0.0006221 0 0 0]  x2=[0 0 0 0; 0.0001244 0 0 0; 0.0002488 0 0 0; 0.0003733 0 0 0; 0.0004977 0 0 0; 0.0006221 0 0 0]  x3=[0 0 0 0; 0.0001244 0 0 0; 0.0002488 0 0 0; 0.0003733 0 0 0; 0.0004977 0 0 0; 0.0006221 0 0 0]  x4=[0 0 0 0; 0.0001244 0 0 0; 0.0002488 0 0 0; 0.0003733 0 0 0; 0.0004977 0 0 0; 0.0006221 0 0 0]  x5=0  V1=ones(3,3)  V2=ones(3,3)  I1=ones(3,3)  I2=ones(3,3)  nHarmo=1  Measurements=None
  Leibnitz___Gosdorf_CN_103401933_110000_CN_83740188_110000 : powerlib/Elements/Distributed Parameters Line  Phases=3  Frequency=60  Resistance=[0.01273 0.3864]  Inductance="[0.9337e-3  4.1264e-3]"  Capacitance=[12.74e-9 7.751e-9]  Length=100  x1=[0 0 0 0; 0.0001244 0 0 0; 0.0002488 0 0 0; 0.0003733 0 0 0; 0.0004977 0 0 0; 0.0006221 0 0 0]  x2=[0 0 0 0; 0.0001244 0 0 0; 0.0002488 0 0 0; 0.0003733 0 0 0; 0.0004977 0 0 0; 0.0006221 0 0 0]  x3=[0 0 0 0; 0.0001244 0 0 0; 0.0002488 0 0 0; 0.0003733 0 0 0; 0.0004977 0 0 0; 0.0006221 0 0 0]  x4=[0 0 0 0; 0.0001244 0 0 0; 0.0002488 0 0 0; 0.0003733 0 0 0; 0.0004977 0 0 0; 0.0006221 0 0 0]  x5=0  V1=ones(3,3)  V2=ones(3,3)  I1=ones(3,3)  I2=ones(3,3)  nHarmo=1  Measurements=None
  Lienz___Amlach_CN_162826525_110000_CN_85291082_110000 : powerlib/Elements/Distributed Parameters Line  Phases=3  Frequency=60  Resistance=[0.01273 0.3864]  Inductance="[0.9337e-3  4.1264e-3]"  Capacitance=[12.74e-9 7.751e-9]  Length=100  x1=[0 0 0 0; 0.0001244 0 0 0; 0.0002488 0 0 0; 0.0003733 0 0 0; 0.0004977 0 0 0; 0.0006221 0 0 0]  x2=[0 0 0 0; 0.0001244 0 0 0; 0.0002488 0 0 0; 0.0003733 0 0 0; 0.0004977 0 0 0; 0.0006221 0 0 0]  x3=[0 0 0 0; 0.0001244 0 0 0; 0.0002488 0 0 0; 0.0003733 0 0 0; 0.0004977 0 0 0; 0.0006221 0 0 0]  x4=[0 0 0 0; 0.0001244 0 0 0; 0.0002488 0 0 0; 0.0003733 0 0 0; 0.0004977 0 0 0; 0.0006221 0 0 0]  x5=0  V1=ones(3,3)  V2=ones(3,3)  I1=ones(3,3)  I2=ones(3,3)  nHarmo=1  Measurements=None
  Lienz___Kalserbach_CN_162826525_110000_CN_85703086_110000 : powerlib/Elements/Distributed Parameters Line  Phases=3  Frequency=60  Resistance=[0.01273 0.3864]  Inductance="[0.9337e-3  4.1264e-3]"  Capacitance=[12.74e-9 7.751e-9]  Length=100  x1=[0 0 0 0; 0.0001244 0 0 0; 0.0002488 0 0 0; 0.0003733 0 0 0; 0.0004977 0 0 0; 0.0006221 0 0 0]  x2=[0 0 0 0; 0.0001244 0 0 0; 0.0002488 0 0 0; 0.0003733 0 0 0; 0.0004977 0 0 0; 0.0006221 0 0 0]  x3=[0 0 0 0; 0.0001244 0 0 0; 0.0002488 0 0 0; 0.0003733 0 0 0; 0.0004977 0 0 0; 0.0006221 0 0 0]  x4=[0 0 0 0; 0.0001244 0 0 0; 0.0002488 0 0 0; 0.0003733 0 0 0; 0.0004977 0 0 0; 0.0006221 0 0 0]  x5=0  V1=ones(3,3)  V2=ones(3,3)  I1=ones(3,3)  I2=ones(3,3)  nHarmo=1  Measurements=None
  Lienz___Stribach_CN_162834614_110000_CN_162826525_110000 : powerlib/Elements/Distributed Parameters Line  Phases=3  Frequency=60  Resistance=[0.01273 0.3864]  Inductance="[0.9337e-3  4.1264e-3]"  Capacitance=[12.74e-9 7.751e-9]  Length=100  x1=[0 0 0 0; 0.0001244 0 0 0; 0.0002488 0 0 0; 0.0003733 0 0 0; 0.0004977 0 0 0; 0.0006221 0 0 0]  x2=[0 0 0 0; 0.0001244 0 0 0; 0.0002488 0 0 0; 0.0003733 0 0 0; 0.0004977 0 0 0; 0.0006221 0 0 0]  x3=[0 0 0 0; 0.0001244 0 0 0; 0.0002488 0 0 0; 0.0003733 0 0 0; 0.0004977 0 0 0; 0.0006221 0 0 0]  x4=[0 0 0 0; 0.0001244 0 0 0; 0.0002488 0 0 0; 0.0003733 0 0 0; 0.0004977 0 0 0; 0.0006221 0 0 0]  x5=0  V1=ones(3,3)  V2=ones(3,3)  I1=ones(3,3)  I2=ones(3,3)  nHarmo=1  Measurements=None
  Lieserhofen___Spittal_an_der_Drau_CN_83892438_110000_CN_86385664_110000 : powerlib/Elements/Distributed Parameters Line  Phases=3  Frequency=60  Resistance=[0.01273 0.3864]  Inductance="[0.9337e-3  4.1264e-3]"  Capacitance=[12.74e-9 7.751e-9]  Length=100  x1=[0 0 0 0; 0.0001244 0 0 0; 0.0002488 0 0 0; 0.0003733 0 0 0; 0.0004977 0 0 0; 0.0006221 0 0 0]  x2=[0 0 0 0; 0.0001244 0 0 0; 0.0002488 0 0 0; 0.0003733 0 0 0; 0.0004977 0 0 0; 0.0006221 0 0 0]  x3=[0 0 0 0; 0.0001244 0 0 0; 0.0002488 0 0 0; 0.0003733 0 0 0; 0.0004977 0 0 0; 0.0006221 0 0 0]  x4=[0 0 0 0; 0.0001244 0 0 0; 0.0002488 0 0 0; 0.0003733 0 0 0; 0.0004977 0 0 0; 0.0006221 0 0 0]  x5=0  V1=ones(3,3)  V2=ones(3,3)  I1=ones(3,3)  I2=ones(3,3)  nHarmo=1  Measurements=None
  Lihula_—_Vigala_110_kV_CN_262755193_110000_CN_34988502_110000 : powerlib/Elements/Distributed Parameters Line  Phases=3  Frequency=60  Resistance=[0.01273 0.3864]  Inductance="[0.9337e-3  4.1264e-3]"  Capacitance=[12.74e-9 7.751e-9]  Length=75.3633  x1=[0 0 0 0; 0.0001244 0 0 0; 0.0002488 0 0 0; 0.0003733 0 0 0; 0.0004977 0 0 0; 0.0006221 0 0 0]  x2=[0 0 0 0; 0.0001244 0 0 0; 0.0002488 0 0 0; 0.0003733 0 0 0; 0.0004977 0 0 0; 0.0006221 0 0 0]  x3=[0 0 0 0; 0.0001244 0 0 0; 0.0002488 0 0 0; 0.0003733 0 0 0; 0.0004977 0 0 0; 0.0006221 0 0 0]  x4=[0 0 0 0; 0.0001244 0 0 0; 0.0002488 0 0 0; 0.0003733 0 0 0; 0.0004977 0 0 0; 0.0006221 0 0 0]  x5=0  V1=ones(3,3)  V2=ones(3,3)  I1=ones(3,3)  I2=ones(3,3)  nHarmo=1  Measurements=None
  Lihula_—_Vigala_110_kV_CN_262755193_110000_CN_34988525_110000 : powerlib/Elements/Distributed Parameters Line  Phases=3  Frequency=60  Resistance=[0.01273 0.3864]  Inductance="[0.9337e-3  4.1264e-3]"  Capacitance=[12.74e-9 7.751e-9]  Length=59.6398  x1=[0 0 0 0; 0.0001244 0 0 0; 0.0002488 0 0 0; 0.0003733 0 0 0; 0.0004977 0 0 0; 0.0006221 0 0 0]  x2=[0 0 0 0; 0.0001244 0 0 0; 0.0002488 0 0 0; 0.0003733 0 0 0; 0.0004977 0 0 0; 0.0006221 0 0 0]  x3=[0 0 0 0; 0.0001244 0 0 0; 0.0002488 0 0 0; 0.0003733 0 0 0; 0.0004977 0 0 0; 0.0006221 0 0 0]  x4=[0 0 0 0; 0.0001244 0 0 0; 0.0002488 0 0 0; 0.0003733 0 0 0; 0.0004977 0 0 0; 0.0006221 0 0 0]  x5=0  V1=ones(3,3)  V2=ones(3,3)  I1=ones(3,3)  I2=ones(3,3)  nHarmo=1  Measurements=None
  Lihula_—_Vigala_110_kV_CN_262755193_110000_CN_35594731_110000 : powerlib/Elements/Distributed Parameters Line  Phases=3  Frequency=60  Resistance=[0.01273 0.3864]  Inductance="[0.9337e-3  4.1264e-3]"  Capacitance=[12.74e-9 7.751e-9]  Length=62.5453  x1=[0 0 0 0; 0.0001244 0 0 0; 0.0002488 0 0 0; 0.0003733 0 0 0; 0.0004977 0 0 0; 0.0006221 0 0 0]  x2=[0 0 0 0; 0.0001244 0 0 0; 0.0002488 0 0 0; 0.0003733 0 0 0; 0.0004977 0 0 0; 0.0006221 0 0 0]  x3=[0 0 0 0; 0.0001244 0 0 0; 0.0002488 0 0 0; 0.0003733 0 0 0; 0.0004977 0 0 0; 0.0006221 0 0 0]  x4=[0 0 0 0; 0.0001244 0 0 0; 0.0002488 0 0 0; 0.0003733 0 0 0; 0.0004977 0 0 0; 0.0006221 0 0 0]  x5=0  V1=ones(3,3)  V2=ones(3,3)  I1=ones(3,3)  I2=ones(3,3)  nHarmo=1  Measurements=None
  Linz_Mitte___Linz_Nord;Katzbach___Linz_Nord_CN_24830381_110000_CN_33077861_110000 : powerlib/Elements/Distributed Parameters Line  Phases=3  Frequency=60  Resistance=[0.01273 0.3864]  Inductance="[0.9337e-3  4.1264e-3]"  Capacitance=[12.74e-9 7.751e-9]  Length=100  x1=[0 0 0 0; 0.0001244 0 0 0; 0.0002488 0 0 0; 0.0003733 0 0 0; 0.0004977 0 0 0; 0.0006221 0 0 0]  x2=[0 0 0 0; 0.0001244 0 0 0; 0.0002488 0 0 0; 0.0003733 0 0 0; 0.0004977 0 0 0; 0.0006221 0 0 0]  x3=[0 0 0 0; 0.0001244 0 0 0; 0.0002488 0 0 0; 0.0003733 0 0 0; 0.0004977 0 0 0; 0.0006221 0 0 0]  x4=[0 0 0 0; 0.0001244 0 0 0; 0.0002488 0 0 0; 0.0003733 0 0 0; 0.0004977 0 0 0; 0.0006221 0 0 0]  x5=0  V1=ones(3,3)  V2=ones(3,3)  I1=ones(3,3)  I2=ones(3,3)  nHarmo=1  Measurements=None
  Maaritsa_—_Kanepi_110_kV_CN_35445333_110000_CN_262457166_110000 : powerlib/Elements/Distributed Parameters Line  Phases=3  Frequency=60  Resistance=[0.01273 0.3864]  Inductance="[0.9337e-3  4.1264e-3]"  Capacitance=[12.74e-9 7.751e-9]  Length=86.0718  x1=[0 0 0 0; 0.0001244 0 0 0; 0.0002488 0 0 0; 0.0003733 0 0 0; 0.0004977 0 0 0; 0.0006221 0 0 0]  x2=[0 0 0 0; 0.0001244 0 0 0; 0.0002488 0 0 0; 0.0003733 0 0 0; 0.0004977 0 0 0; 0.0006221 0 0 0]  x3=[0 0 0 0; 0.0001244 0 0 0; 0.0002488 0 0 0; 0.0003733 0 0 0; 0.0004977 0 0 0; 0.0006221 0 0 0]  x4=[0 0 0 0; 0.0001244 0 0 0; 0.0002488 0 0 0; 0.0003733 0 0 0; 0.0004977 0 0 0; 0.0006221 0 0 0]  x5=0  V1=ones(3,3)  V2=ones(3,3)  I1=ones(3,3)  I2=ones(3,3)  nHarmo=1  Measurements=None
  Maaritsa_—_Kanepi_110_kV_CN_35445333_110000_CN_34682089_110000 : powerlib/Elements/Distributed Parameters Line  Phases=3  Frequency=60  Resistance=[0.01273 0.3864]  Inductance="[0.9337e-3  4.1264e-3]"  Capacitance=[12.74e-9 7.751e-9]  Length=47.5565  x1=[0 0 0 0; 0.0001244 0 0 0; 0.0002488 0 0 0; 0.0003733 0 0 0; 0.0004977 0 0 0; 0.0006221 0 0 0]  x2=[0 0 0 0; 0.0001244 0 0 0; 0.0002488 0 0 0; 0.0003733 0 0 0; 0.0004977 0 0 0; 0.0006221 0 0 0]  x3=[0 0 0 0; 0.0001244 0 0 0; 0.0002488 0 0 0; 0.0003733 0 0 0; 0.0004977 0 0 0; 0.0006221 0 0 0]  x4=[0 0 0 0; 0.0001244 0 0 0; 0.0002488 0 0 0; 0.0003733 0 0 0; 0.0004977 0 0 0; 0.0006221 0 0 0]  x5=0  V1=ones(3,3)  V2=ones(3,3)  I1=ones(3,3)  I2=ones(3,3)  nHarmo=1  Measurements=None
  Maaritsa_—_Kanepi_110_kV_CN_35445333_110000_CN_35420117_110000 : powerlib/Elements/Distributed Parameters Line  Phases=3  Frequency=60  Resistance=[0.01273 0.3864]  Inductance="[0.9337e-3  4.1264e-3]"  Capacitance=[12.74e-9 7.751e-9]  Length=20.2735  x1=[0 0 0 0; 0.0001244 0 0 0; 0.0002488 0 0 0; 0.0003733 0 0 0; 0.0004977 0 0 0; 0.0006221 0 0 0]  x2=[0 0 0 0; 0.0001244 0 0 0; 0.0002488 0 0 0; 0.0003733 0 0 0; 0.0004977 0 0 0; 0.0006221 0 0 0]  x3=[0 0 0 0; 0.0001244 0 0 0; 0.0002488 0 0 0; 0.0003733 0 0 0; 0.0004977 0 0 0; 0.0006221 0 0 0]  x4=[0 0 0 0; 0.0001244 0 0 0; 0.0002488 0 0 0; 0.0003733 0 0 0; 0.0004977 0 0 0; 0.0006221 0 0 0]  x5=0  V1=ones(3,3)  V2=ones(3,3)  I1=ones(3,3)  I2=ones(3,3)  nHarmo=1  Measurements=None
  Maaritsa_—_Kanepi_110_kV_CN_35445333_110000_CN_35420119_110000 : powerlib/Elements/Distributed Parameters Line  Phases=3  Frequency=60  Resistance=[0.01273 0.3864]  Inductance="[0.9337e-3  4.1264e-3]"  Capacitance=[12.74e-9 7.751e-9]  Length=70.7718  x1=[0 0 0 0; 0.0001244 0 0 0; 0.0002488 0 0 0; 0.0003733 0 0 0; 0.0004977 0 0 0; 0.0006221 0 0 0]  x2=[0 0 0 0; 0.0001244 0 0 0; 0.0002488 0 0 0; 0.0003733 0 0 0; 0.0004977 0 0 0; 0.0006221 0 0 0]  x3=[0 0 0 0; 0.0001244 0 0 0; 0.0002488 0 0 0; 0.0003733 0 0 0; 0.0004977 0 0 0; 0.0006221 0 0 0]  x4=[0 0 0 0; 0.0001244 0 0 0; 0.0002488 0 0 0; 0.0003733 0 0 0; 0.0004977 0 0 0; 0.0006221 0 0 0]  x5=0  V1=ones(3,3)  V2=ones(3,3)  I1=ones(3,3)  I2=ones(3,3)  nHarmo=1  Measurements=None
  Marchtrenk___Wels_Ost_CN_40917240_110000_CN_87526678_110000 : powerlib/Elements/Distributed Parameters Line  Phases=3  Frequency=60  Resistance=[0.01273 0.3864]  Inductance="[0.9337e-3  4.1264e-3]"  Capacitance=[12.74e-9 7.751e-9]  Length=100  x1=[0 0 0 0; 0.0001244 0 0 0; 0.0002488 0 0 0; 0.0003733 0 0 0; 0.0004977 0 0 0; 0.0006221 0 0 0]  x2=[0 0 0 0; 0.0001244 0 0 0; 0.0002488 0 0 0; 0.0003733 0 0 0; 0.0004977 0 0 0; 0.0006221 0 0 0]  x3=[0 0 0 0; 0.0001244 0 0 0; 0.0002488 0 0 0; 0.0003733 0 0 0; 0.0004977 0 0 0; 0.0006221 0 0 0]  x4=[0 0 0 0; 0.0001244 0 0 0; 0.0002488 0 0 0; 0.0003733 0 0 0; 0.0004977 0 0 0; 0.0006221 0 0 0]  x5=0  V1=ones(3,3)  V2=ones(3,3)  I1=ones(3,3)  I2=ones(3,3)  nHarmo=1  Measurements=None
  Marchtrenk_–_Attnang_Puchheim_CN_33685690_110000_CN_39271873_110000 : powerlib/Elements/Distributed Parameters Line  Phases=3  Frequency=60  Resistance=[0.01273 0.3864]  Inductance="[0.9337e-3  4.1264e-3]"  Capacitance=[12.74e-9 7.751e-9]  Length=100  x1=[0 0 0 0; 0.0001244 0 0 0; 0.0002488 0 0 0; 0.0003733 0 0 0; 0.0004977 0 0 0; 0.0006221 0 0 0]  x2=[0 0 0 0; 0.0001244 0 0 0; 0.0002488 0 0 0; 0.0003733 0 0 0; 0.0004977 0 0 0; 0.0006221 0 0 0]  x3=[0 0 0 0; 0.0001244 0 0 0; 0.0002488 0 0 0; 0.0003733 0 0 0; 0.0004977 0 0 0; 0.0006221 0 0 0]  x4=[0 0 0 0; 0.0001244 0 0 0; 0.0002488 0 0 0; 0.0003733 0 0 0; 0.0004977 0 0 0; 0.0006221 0 0 0]  x5=0  V1=ones(3,3)  V2=ones(3,3)  I1=ones(3,3)  I2=ones(3,3)  nHarmo=1  Measurements=None
  Mast_144_–_Zellerndorf_CN_90683456_110000_CN_95227815_110000 : powerlib/Elements/Distributed Parameters Line  Phases=3  Frequency=60  Resistance=[0.01273 0.3864]  Inductance="[0.9337e-3  4.1264e-3]"  Capacitance=[12.74e-9 7.751e-9]  Length=100  x1=[0 0 0 0; 0.0001244 0 0 0; 0.0002488 0 0 0; 0.0003733 0 0 0; 0.0004977 0 0 0; 0.0006221 0 0 0]  x2=[0 0 0 0; 0.0001244 0 0 0; 0.0002488 0 0 0; 0.0003733 0 0 0; 0.0004977 0 0 0; 0.0006221 0 0 0]  x3=[0 0 0 0; 0.0001244 0 0 0; 0.0002488 0 0 0; 0.0003733 0 0 0; 0.0004977 0 0 0; 0.0006221 0 0 0]  x4=[0 0 0 0; 0.0001244 0 0 0; 0.0002488 0 0 0; 0.0003733 0 0 0; 0.0004977 0 0 0; 0.0006221 0 0 0]  x5=0  V1=ones(3,3)  V2=ones(3,3)  I1=ones(3,3)  I2=ones(3,3)  nHarmo=1  Measurements=None
  Mast_72_–_Dorfgastein_CN_91250729_110000_CN_90498611_110000 : powerlib/Elements/Distributed Parameters Line  Phases=3  Frequency=60  Resistance=[0.01273 0.3864]  Inductance="[0.9337e-3  4.1264e-3]"  Capacitance=[12.74e-9 7.751e-9]  Length=100  x1=[0 0 0 0; 0.0001244 0 0 0; 0.0002488 0 0 0; 0.0003733 0 0 0; 0.0004977 0 0 0; 0.0006221 0 0 0]  x2=[0 0 0 0; 0.0001244 0 0 0; 0.0002488 0 0 0; 0.0003733 0 0 0; 0.0004977 0 0 0; 0.0006221 0 0 0]  x3=[0 0 0 0; 0.0001244 0 0 0; 0.0002488 0 0 0; 0.0003733 0 0 0; 0.0004977 0 0 0; 0.0006221 0 0 0]  x4=[0 0 0 0; 0.0001244 0 0 0; 0.0002488 0 0 0; 0.0003733 0 0 0; 0.0004977 0 0 0; 0.0006221 0 0 0]  x5=0  V1=ones(3,3)  V2=ones(3,3)  I1=ones(3,3)  I2=ones(3,3)  nHarmo=1  Measurements=None
  Matrei_–_Gries_Brenner_CN_99877186_110000_CN_146122262_110000 : powerlib/Elements/Distributed Parameters Line  Phases=3  Frequency=60  Resistance=[0.01273 0.3864]  Inductance="[0.9337e-3  4.1264e-3]"  Capacitance=[12.74e-9 7.751e-9]  Length=100  x1=[0 0 0 0; 0.0001244 0 0 0; 0.0002488 0 0 0; 0.0003733 0 0 0; 0.0004977 0 0 0; 0.0006221 0 0 0]  x2=[0 0 0 0; 0.0001244 0 0 0; 0.0002488 0 0 0; 0.0003733 0 0 0; 0.0004977 0 0 0; 0.0006221 0 0 0]  x3=[0 0 0 0; 0.0001244 0 0 0; 0.0002488 0 0 0; 0.0003733 0 0 0; 0.0004977 0 0 0; 0.0006221 0 0 0]  x4=[0 0 0 0; 0.0001244 0 0 0; 0.0002488 0 0 0; 0.0003733 0 0 0; 0.0004977 0 0 0; 0.0006221 0 0 0]  x5=0  V1=ones(3,3)  V2=ones(3,3)  I1=ones(3,3)  I2=ones(3,3)  nHarmo=1  Measurements=None
  Matrei_–_Gries_Brenner_CN_99877186_110000_CN_32465765_110000 : powerlib/Elements/Distributed Parameters Line  Phases=3  Frequency=60  Resistance=[0.01273 0.3864]  Inductance="[0.9337e-3  4.1264e-3]"  Capacitance=[12.74e-9 7.751e-9]  Length=100  x1=[0 0 0 0; 0.0001244 0 0 0; 0.0002488 0 0 0; 0.0003733 0 0 0; 0.0004977 0 0 0; 0.0006221 0 0 0]  x2=[0 0 0 0; 0.0001244 0 0 0; 0.0002488 0 0 0; 0.0003733 0 0 0; 0.0004977 0 0 0; 0.0006221 0 0 0]  x3=[0 0 0 0; 0.0001244 0 0 0; 0.0002488 0 0 0; 0.0003733 0 0 0; 0.0004977 0 0 0; 0.0006221 0 0 0]  x4=[0 0 0 0; 0.0001244 0 0 0; 0.0002488 0 0 0; 0.0003733 0 0 0; 0.0004977 0 0 0; 0.0006221 0 0 0]  x5=0  V1=ones(3,3)  V2=ones(3,3)  I1=ones(3,3)  I2=ones(3,3)  nHarmo=1  Measurements=None
  Mauthausen___Friensdorf_CN_95828347_110000_CN_15734776_110000 : powerlib/Elements/Distributed Parameters Line  Phases=3  Frequency=60  Resistance=[0.01273 0.3864]  Inductance="[0.9337e-3  4.1264e-3]"  Capacitance=[12.74e-9 7.751e-9]  Length=100  x1=[0 0 0 0; 0.0001244 0 0 0; 0.0002488 0 0 0; 0.0003733 0 0 0; 0.0004977 0 0 0; 0.0006221 0 0 0]  x2=[0 0 0 0; 0.0001244 0 0 0; 0.0002488 0 0 0; 0.0003733 0 0 0; 0.0004977 0 0 0; 0.0006221 0 0 0]  x3=[0 0 0 0; 0.0001244 0 0 0; 0.0002488 0 0 0; 0.0003733 0 0 0; 0.0004977 0 0 0; 0.0006221 0 0 0]  x4=[0 0 0 0; 0.0001244 0 0 0; 0.0002488 0 0 0; 0.0003733 0 0 0; 0.0004977 0 0 0; 0.0006221 0 0 0]  x5=0  V1=ones(3,3)  V2=ones(3,3)  I1=ones(3,3)  I2=ones(3,3)  nHarmo=1  Measurements=None
  Mauthausen___Friensdorf_CN_95828347_110000_CN_33077861_110000 : powerlib/Elements/Distributed Parameters Line  Phases=3  Frequency=60  Resistance=[0.01273 0.3864]  Inductance="[0.9337e-3  4.1264e-3]"  Capacitance=[12.74e-9 7.751e-9]  Length=100  x1=[0 0 0 0; 0.0001244 0 0 0; 0.0002488 0 0 0; 0.0003733 0 0 0; 0.0004977 0 0 0; 0.0006221 0 0 0]  x2=[0 0 0 0; 0.0001244 0 0 0; 0.0002488 0 0 0; 0.0003733 0 0 0; 0.0004977 0 0 0; 0.0006221 0 0 0]  x3=[0 0 0 0; 0.0001244 0 0 0; 0.0002488 0 0 0; 0.0003733 0 0 0; 0.0004977 0 0 0; 0.0006221 0 0 0]  x4=[0 0 0 0; 0.0001244 0 0 0; 0.0002488 0 0 0; 0.0003733 0 0 0; 0.0004977 0 0 0; 0.0006221 0 0 0]  x5=0  V1=ones(3,3)  V2=ones(3,3)  I1=ones(3,3)  I2=ones(3,3)  nHarmo=1  Measurements=None
  Mauthausen___Friensdorf_CN_95828347_110000_CN_93370554_110000 : powerlib/Elements/Distributed Parameters Line  Phases=3  Frequency=60  Resistance=[0.01273 0.3864]  Inductance="[0.9337e-3  4.1264e-3]"  Capacitance=[12.74e-9 7.751e-9]  Length=100  x1=[0 0 0 0; 0.0001244 0 0 0; 0.0002488 0 0 0; 0.0003733 0 0 0; 0.0004977 0 0 0; 0.0006221 0 0 0]  x2=[0 0 0 0; 0.0001244 0 0 0; 0.0002488 0 0 0; 0.0003733 0 0 0; 0.0004977 0 0 0; 0.0006221 0 0 0]  x3=[0 0 0 0; 0.0001244 0 0 0; 0.0002488 0 0 0; 0.0003733 0 0 0; 0.0004977 0 0 0; 0.0006221 0 0 0]  x4=[0 0 0 0; 0.0001244 0 0 0; 0.0002488 0 0 0; 0.0003733 0 0 0; 0.0004977 0 0 0; 0.0006221 0 0 0]  x5=0  V1=ones(3,3)  V2=ones(3,3)  I1=ones(3,3)  I2=ones(3,3)  nHarmo=1  Measurements=None
  Mauthausen___Friensdorf_CN_95828347_110000_CN_95843031_110000 : powerlib/Elements/Distributed Parameters Line  Phases=3  Frequency=60  Resistance=[0.01273 0.3864]  Inductance="[0.9337e-3  4.1264e-3]"  Capacitance=[12.74e-9 7.751e-9]  Length=100  x1=[0 0 0 0; 0.0001244 0 0 0; 0.0002488 0 0 0; 0.0003733 0 0 0; 0.0004977 0 0 0; 0.0006221 0 0 0]  x2=[0 0 0 0; 0.0001244 0 0 0; 0.0002488 0 0 0; 0.0003733 0 0 0; 0.0004977 0 0 0; 0.0006221 0 0 0]  x3=[0 0 0 0; 0.0001244 0 0 0; 0.0002488 0 0 0; 0.0003733 0 0 0; 0.0004977 0 0 0; 0.0006221 0 0 0]  x4=[0 0 0 0; 0.0001244 0 0 0; 0.0002488 0 0 0; 0.0003733 0 0 0; 0.0004977 0 0 0; 0.0006221 0 0 0]  x5=0  V1=ones(3,3)  V2=ones(3,3)  I1=ones(3,3)  I2=ones(3,3)  nHarmo=1  Measurements=None
  Meiningen___Frastanz_gelb_CN_61108302_110000_CN_102699327_110000 : powerlib/Elements/Distributed Parameters Line  Phases=3  Frequency=60  Resistance=[0.01273 0.3864]  Inductance="[0.9337e-3  4.1264e-3]"  Capacitance=[12.74e-9 7.751e-9]  Length=100  x1=[0 0 0 0; 0.0001244 0 0 0; 0.0002488 0 0 0; 0.0003733 0 0 0; 0.0004977 0 0 0; 0.0006221 0 0 0]  x2=[0 0 0 0; 0.0001244 0 0 0; 0.0002488 0 0 0; 0.0003733 0 0 0; 0.0004977 0 0 0; 0.0006221 0 0 0]  x3=[0 0 0 0; 0.0001244 0 0 0; 0.0002488 0 0 0; 0.0003733 0 0 0; 0.0004977 0 0 0; 0.0006221 0 0 0]  x4=[0 0 0 0; 0.0001244 0 0 0; 0.0002488 0 0 0; 0.0003733 0 0 0; 0.0004977 0 0 0; 0.0006221 0 0 0]  x5=0  V1=ones(3,3)  V2=ones(3,3)  I1=ones(3,3)  I2=ones(3,3)  nHarmo=1  Measurements=None
  Meiningen___Frastanz_gelb_CN_61108302_110000_CN_119687430_110000 : powerlib/Elements/Distributed Parameters Line  Phases=3  Frequency=60  Resistance=[0.01273 0.3864]  Inductance="[0.9337e-3  4.1264e-3]"  Capacitance=[12.74e-9 7.751e-9]  Length=100  x1=[0 0 0 0; 0.0001244 0 0 0; 0.0002488 0 0 0; 0.0003733 0 0 0; 0.0004977 0 0 0; 0.0006221 0 0 0]  x2=[0 0 0 0; 0.0001244 0 0 0; 0.0002488 0 0 0; 0.0003733 0 0 0; 0.0004977 0 0 0; 0.0006221 0 0 0]  x3=[0 0 0 0; 0.0001244 0 0 0; 0.0002488 0 0 0; 0.0003733 0 0 0; 0.0004977 0 0 0; 0.0006221 0 0 0]  x4=[0 0 0 0; 0.0001244 0 0 0; 0.0002488 0 0 0; 0.0003733 0 0 0; 0.0004977 0 0 0; 0.0006221 0 0 0]  x5=0  V1=ones(3,3)  V2=ones(3,3)  I1=ones(3,3)  I2=ones(3,3)  nHarmo=1  Measurements=None
  Meiningen___Frastanz_gelb_CN_61108302_110000_CN_26524546_110000 : powerlib/Elements/Distributed Parameters Line  Phases=3  Frequency=60  Resistance=[0.01273 0.3864]  Inductance="[0.9337e-3  4.1264e-3]"  Capacitance=[12.74e-9 7.751e-9]  Length=100  x1=[0 0 0 0; 0.0001244 0 0 0; 0.0002488 0 0 0; 0.0003733 0 0 0; 0.0004977 0 0 0; 0.0006221 0 0 0]  x2=[0 0 0 0; 0.0001244 0 0 0; 0.0002488 0 0 0; 0.0003733 0 0 0; 0.0004977 0 0 0; 0.0006221 0 0 0]  x3=[0 0 0 0; 0.0001244 0 0 0; 0.0002488 0 0 0; 0.0003733 0 0 0; 0.0004977 0 0 0; 0.0006221 0 0 0]  x4=[0 0 0 0; 0.0001244 0 0 0; 0.0002488 0 0 0; 0.0003733 0 0 0; 0.0004977 0 0 0; 0.0006221 0 0 0]  x5=0  V1=ones(3,3)  V2=ones(3,3)  I1=ones(3,3)  I2=ones(3,3)  nHarmo=1  Measurements=None
  Meiningen___Frastanz_gelb_CN_61108302_110000_CN_32293834_110000 : powerlib/Elements/Distributed Parameters Line  Phases=3  Frequency=60  Resistance=[0.01273 0.3864]  Inductance="[0.9337e-3  4.1264e-3]"  Capacitance=[12.74e-9 7.751e-9]  Length=100  x1=[0 0 0 0; 0.0001244 0 0 0; 0.0002488 0 0 0; 0.0003733 0 0 0; 0.0004977 0 0 0; 0.0006221 0 0 0]  x2=[0 0 0 0; 0.0001244 0 0 0; 0.0002488 0 0 0; 0.0003733 0 0 0; 0.0004977 0 0 0; 0.0006221 0 0 0]  x3=[0 0 0 0; 0.0001244 0 0 0; 0.0002488 0 0 0; 0.0003733 0 0 0; 0.0004977 0 0 0; 0.0006221 0 0 0]  x4=[0 0 0 0; 0.0001244 0 0 0; 0.0002488 0 0 0; 0.0003733 0 0 0; 0.0004977 0 0 0; 0.0006221 0 0 0]  x5=0  V1=ones(3,3)  V2=ones(3,3)  I1=ones(3,3)  I2=ones(3,3)  nHarmo=1  Measurements=None
  Mistelbach_–_Zellerndorf_CN_90683456_110000_CN_97402227_110000 : powerlib/Elements/Distributed Parameters Line  Phases=3  Frequency=60  Resistance=[0.01273 0.3864]  Inductance="[0.9337e-3  4.1264e-3]"  Capacitance=[12.74e-9 7.751e-9]  Length=100  x1=[0 0 0 0; 0.0001244 0 0 0; 0.0002488 0 0 0; 0.0003733 0 0 0; 0.0004977 0 0 0; 0.0006221 0 0 0]  x2=[0 0 0 0; 0.0001244 0 0 0; 0.0002488 0 0 0; 0.0003733 0 0 0; 0.0004977 0 0 0; 0.0006221 0 0 0]  x3=[0 0 0 0; 0.0001244 0 0 0; 0.0002488 0 0 0; 0.0003733 0 0 0; 0.0004977 0 0 0; 0.0006221 0 0 0]  x4=[0 0 0 0; 0.0001244 0 0 0; 0.0002488 0 0 0; 0.0003733 0 0 0; 0.0004977 0 0 0; 0.0006221 0 0 0]  x5=0  V1=ones(3,3)  V2=ones(3,3)  I1=ones(3,3)  I2=ones(3,3)  nHarmo=1  Measurements=None
  Moosbrunn___Wien_Südost_CN_27795895_110000_CN_25539735_110000 : powerlib/Elements/Distributed Parameters Line  Phases=3  Frequency=60  Resistance=[0.01273 0.3864]  Inductance="[0.9337e-3  4.1264e-3]"  Capacitance=[12.74e-9 7.751e-9]  Length=100  x1=[0 0 0 0; 0.0001244 0 0 0; 0.0002488 0 0 0; 0.0003733 0 0 0; 0.0004977 0 0 0; 0.0006221 0 0 0]  x2=[0 0 0 0; 0.0001244 0 0 0; 0.0002488 0 0 0; 0.0003733 0 0 0; 0.0004977 0 0 0; 0.0006221 0 0 0]  x3=[0 0 0 0; 0.0001244 0 0 0; 0.0002488 0 0 0; 0.0003733 0 0 0; 0.0004977 0 0 0; 0.0006221 0 0 0]  x4=[0 0 0 0; 0.0001244 0 0 0; 0.0002488 0 0 0; 0.0003733 0 0 0; 0.0004977 0 0 0; 0.0006221 0 0 0]  x5=0  V1=ones(3,3)  V2=ones(3,3)  I1=ones(3,3)  I2=ones(3,3)  nHarmo=1  Measurements=None
  Muhu_haruliin_CN_35022081_110000_CN_34988518_110000 : powerlib/Elements/Distributed Parameters Line  Phases=3  Frequency=60  Resistance=[0.01273 0.3864]  Inductance="[0.9337e-3  4.1264e-3]"  Capacitance=[12.74e-9 7.751e-9]  Length=21.2382  x1=[0 0 0 0; 0.0001244 0 0 0; 0.0002488 0 0 0; 0.0003733 0 0 0; 0.0004977 0 0 0; 0.0006221 0 0 0]  x2=[0 0 0 0; 0.0001244 0 0 0; 0.0002488 0 0 0; 0.0003733 0 0 0; 0.0004977 0 0 0; 0.0006221 0 0 0]  x3=[0 0 0 0; 0.0001244 0 0 0; 0.0002488 0 0 0; 0.0003733 0 0 0; 0.0004977 0 0 0; 0.0006221 0 0 0]  x4=[0 0 0 0; 0.0001244 0 0 0; 0.0002488 0 0 0; 0.0003733 0 0 0; 0.0004977 0 0 0; 0.0006221 0 0 0]  x5=0  V1=ones(3,3)  V2=ones(3,3)  I1=ones(3,3)  I2=ones(3,3)  nHarmo=1  Measurements=None
  Muhu_haruliin_CN_35022081_110000_CN_34988522_110000 : powerlib/Elements/Distributed Parameters Line  Phases=3  Frequency=60  Resistance=[0.01273 0.3864]  Inductance="[0.9337e-3  4.1264e-3]"  Capacitance=[12.74e-9 7.751e-9]  Length=19.1107  x1=[0 0 0 0; 0.0001244 0 0 0; 0.0002488 0 0 0; 0.0003733 0 0 0; 0.0004977 0 0 0; 0.0006221 0 0 0]  x2=[0 0 0 0; 0.0001244 0 0 0; 0.0002488 0 0 0; 0.0003733 0 0 0; 0.0004977 0 0 0; 0.0006221 0 0 0]  x3=[0 0 0 0; 0.0001244 0 0 0; 0.0002488 0 0 0; 0.0003733 0 0 0; 0.0004977 0 0 0; 0.0006221 0 0 0]  x4=[0 0 0 0; 0.0001244 0 0 0; 0.0002488 0 0 0; 0.0003733 0 0 0; 0.0004977 0 0 0; 0.0006221 0 0 0]  x5=0  V1=ones(3,3)  V2=ones(3,3)  I1=ones(3,3)  I2=ones(3,3)  nHarmo=1  Measurements=None
  Nõva_—_Aulepa_110_kV_CN_101177924_110000_CN_34988495_110000 : powerlib/Elements/Distributed Parameters Line  Phases=3  Frequency=60  Resistance=[0.01273 0.3864]  Inductance="[0.9337e-3  4.1264e-3]"  Capacitance=[12.74e-9 7.751e-9]  Length=17.0454  x1=[0 0 0 0; 0.0001244 0 0 0; 0.0002488 0 0 0; 0.0003733 0 0 0; 0.0004977 0 0 0; 0.0006221 0 0 0]  x2=[0 0 0 0; 0.0001244 0 0 0; 0.0002488 0 0 0; 0.0003733 0 0 0; 0.0004977 0 0 0; 0.0006221 0 0 0]  x3=[0 0 0 0; 0.0001244 0 0 0; 0.0002488 0 0 0; 0.0003733 0 0 0; 0.0004977 0 0 0; 0.0006221 0 0 0]  x4=[0 0 0 0; 0.0001244 0 0 0; 0.0002488 0 0 0; 0.0003733 0 0 0; 0.0004977 0 0 0; 0.0006221 0 0 0]  x5=0  V1=ones(3,3)  V2=ones(3,3)  I1=ones(3,3)  I2=ones(3,3)  nHarmo=1  Measurements=None
  Obervellach_–_Pusarnitz;Mallnitz_–_Pusarnitz_CN_83892409_110000_CN_83823666_110000 : powerlib/Elements/Distributed Parameters Line  Phases=3  Frequency=60  Resistance=[0.01273 0.3864]  Inductance="[0.9337e-3  4.1264e-3]"  Capacitance=[12.74e-9 7.751e-9]  Length=100  x1=[0 0 0 0; 0.0001244 0 0 0; 0.0002488 0 0 0; 0.0003733 0 0 0; 0.0004977 0 0 0; 0.0006221 0 0 0]  x2=[0 0 0 0; 0.0001244 0 0 0; 0.0002488 0 0 0; 0.0003733 0 0 0; 0.0004977 0 0 0; 0.0006221 0 0 0]  x3=[0 0 0 0; 0.0001244 0 0 0; 0.0002488 0 0 0; 0.0003733 0 0 0; 0.0004977 0 0 0; 0.0006221 0 0 0]  x4=[0 0 0 0; 0.0001244 0 0 0; 0.0002488 0 0 0; 0.0003733 0 0 0; 0.0004977 0 0 0; 0.0006221 0 0 0]  x5=0  V1=ones(3,3)  V2=ones(3,3)  I1=ones(3,3)  I2=ones(3,3)  nHarmo=1  Measurements=None
  Obervellach_–_Pusarnitz;Mallnitz_–_Pusarnitz_CN_83892409_110000_CN_84526686_110000 : powerlib/Elements/Distributed Parameters Line  Phases=3  Frequency=60  Resistance=[0.01273 0.3864]  Inductance="[0.9337e-3  4.1264e-3]"  Capacitance=[12.74e-9 7.751e-9]  Length=100  x1=[0 0 0 0; 0.0001244 0 0 0; 0.0002488 0 0 0; 0.0003733 0 0 0; 0.0004977 0 0 0; 0.0006221 0 0 0]  x2=[0 0 0 0; 0.0001244 0 0 0; 0.0002488 0 0 0; 0.0003733 0 0 0; 0.0004977 0 0 0; 0.0006221 0 0 0]  x3=[0 0 0 0; 0.0001244 0 0 0; 0.0002488 0 0 0; 0.0003733 0 0 0; 0.0004977 0 0 0; 0.0006221 0 0 0]  x4=[0 0 0 0; 0.0001244 0 0 0; 0.0002488 0 0 0; 0.0003733 0 0 0; 0.0004977 0 0 0; 0.0006221 0 0 0]  x5=0  V1=ones(3,3)  V2=ones(3,3)  I1=ones(3,3)  I2=ones(3,3)  nHarmo=1  Measurements=None
  Ohlsdorf___Steyrermühl;Laakirchen___Traunfall_CN_32809456_110000_CN_30842675_110000 : powerlib/Elements/Distributed Parameters Line  Phases=3  Frequency=60  Resistance=[0.01273 0.3864]  Inductance="[0.9337e-3  4.1264e-3]"  Capacitance=[12.74e-9 7.751e-9]  Length=100  x1=[0 0 0 0; 0.0001244 0 0 0; 0.0002488 0 0 0; 0.0003733 0 0 0; 0.0004977 0 0 0; 0.0006221 0 0 0]  x2=[0 0 0 0; 0.0001244 0 0 0; 0.0002488 0 0 0; 0.0003733 0 0 0; 0.0004977 0 0 0; 0.0006221 0 0 0]  x3=[0 0 0 0; 0.0001244 0 0 0; 0.0002488 0 0 0; 0.0003733 0 0 0; 0.0004977 0 0 0; 0.0006221 0 0 0]  x4=[0 0 0 0; 0.0001244 0 0 0; 0.0002488 0 0 0; 0.0003733 0 0 0; 0.0004977 0 0 0; 0.0006221 0 0 0]  x5=0  V1=ones(3,3)  V2=ones(3,3)  I1=ones(3,3)  I2=ones(3,3)  nHarmo=1  Measurements=None
  Ohlsdorf___Steyrermühl;Laakirchen___Traunfall_CN_32809456_110000_CN_95456147_110000 : powerlib/Elements/Distributed Parameters Line  Phases=3  Frequency=60  Resistance=[0.01273 0.3864]  Inductance="[0.9337e-3  4.1264e-3]"  Capacitance=[12.74e-9 7.751e-9]  Length=100  x1=[0 0 0 0; 0.0001244 0 0 0; 0.0002488 0 0 0; 0.0003733 0 0 0; 0.0004977 0 0 0; 0.0006221 0 0 0]  x2=[0 0 0 0; 0.0001244 0 0 0; 0.0002488 0 0 0; 0.0003733 0 0 0; 0.0004977 0 0 0; 0.0006221 0 0 0]  x3=[0 0 0 0; 0.0001244 0 0 0; 0.0002488 0 0 0; 0.0003733 0 0 0; 0.0004977 0 0 0; 0.0006221 0 0 0]  x4=[0 0 0 0; 0.0001244 0 0 0; 0.0002488 0 0 0; 0.0003733 0 0 0; 0.0004977 0 0 0; 0.0006221 0 0 0]  x5=0  V1=ones(3,3)  V2=ones(3,3)  I1=ones(3,3)  I2=ones(3,3)  nHarmo=1  Measurements=None
  Oiu_haruliin_CN_36977398_110000_CN_180118919_110000 : powerlib/Elements/Distributed Parameters Line  Phases=3  Frequency=60  Resistance=[0.01273 0.3864]  Inductance="[0.9337e-3  4.1264e-3]"  Capacitance=[12.74e-9 7.751e-9]  Length=110.1944  x1=[0 0 0 0; 0.0001244 0 0 0; 0.0002488 0 0 0; 0.0003733 0 0 0; 0.0004977 0 0 0; 0.0006221 0 0 0]  x2=[0 0 0 0; 0.0001244 0 0 0; 0.0002488 0 0 0; 0.0003733 0 0 0; 0.0004977 0 0 0; 0.0006221 0 0 0]  x3=[0 0 0 0; 0.0001244 0 0 0; 0.0002488 0 0 0; 0.0003733 0 0 0; 0.0004977 0 0 0; 0.0006221 0 0 0]  x4=[0 0 0 0; 0.0001244 0 0 0; 0.0002488 0 0 0; 0.0003733 0 0 0; 0.0004977 0 0 0; 0.0006221 0 0 0]  x5=0  V1=ones(3,3)  V2=ones(3,3)  I1=ones(3,3)  I2=ones(3,3)  nHarmo=1  Measurements=None
  Ottensheim___Wegscheid_CN_102572506_110000_CN_91579706_110000 : powerlib/Elements/Distributed Parameters Line  Phases=3  Frequency=60  Resistance=[0.01273 0.3864]  Inductance="[0.9337e-3  4.1264e-3]"  Capacitance=[12.74e-9 7.751e-9]  Length=100  x1=[0 0 0 0; 0.0001244 0 0 0; 0.0002488 0 0 0; 0.0003733 0 0 0; 0.0004977 0 0 0; 0.0006221 0 0 0]  x2=[0 0 0 0; 0.0001244 0 0 0; 0.0002488 0 0 0; 0.0003733 0 0 0; 0.0004977 0 0 0; 0.0006221 0 0 0]  x3=[0 0 0 0; 0.0001244 0 0 0; 0.0002488 0 0 0; 0.0003733 0 0 0; 0.0004977 0 0 0; 0.0006221 0 0 0]  x4=[0 0 0 0; 0.0001244 0 0 0; 0.0002488 0 0 0; 0.0003733 0 0 0; 0.0004977 0 0 0; 0.0006221 0 0 0]  x5=0  V1=ones(3,3)  V2=ones(3,3)  I1=ones(3,3)  I2=ones(3,3)  nHarmo=1  Measurements=None
  Paide_—_Kiisa_330_kV_CN_34935436_330000_CN_35343343_330000 : powerlib/Elements/Distributed Parameters Line  Phases=3  Frequency=60  Resistance=[0.01273 0.3864]  Inductance="[0.9337e-3  4.1264e-3]"  Capacitance=[12.74e-9 7.751e-9]  Length=18.3671  x1=[0 0 0 0; 0.0001244 0 0 0; 0.0002488 0 0 0; 0.0003733 0 0 0; 0.0004977 0 0 0; 0.0006221 0 0 0]  x2=[0 0 0 0; 0.0001244 0 0 0; 0.0002488 0 0 0; 0.0003733 0 0 0; 0.0004977 0 0 0; 0.0006221 0 0 0]  x3=[0 0 0 0; 0.0001244 0 0 0; 0.0002488 0 0 0; 0.0003733 0 0 0; 0.0004977 0 0 0; 0.0006221 0 0 0]  x4=[0 0 0 0; 0.0001244 0 0 0; 0.0002488 0 0 0; 0.0003733 0 0 0; 0.0004977 0 0 0; 0.0006221 0 0 0]  x5=0  V1=ones(3,3)  V2=ones(3,3)  I1=ones(3,3)  I2=ones(3,3)  nHarmo=1  Measurements=None
